simulink model "tracking_model"  (R2017a)
(part 6 of 14)

37e-11+cos(x_3).^2.*sin(x_3).^2.*7.5816135984375e-6+cos(x_4).^2.*sin(x_3).^4.*6.757062187003037e-11+cos(x_5).^2.*sin(x_3).^4.*6.757062187003037e-11+cos(x_6).^2.*sin(x_3).^4.*6.757062187003037e-11+cos(x_3).^2.*cos(x_4).^2.*sin(x_3).^2.*1.351412437400607e-10+cos(x_3).^2.*cos(x_5).^2.*sin(x_3).^2.*1.351412437400607e-10+cos(x_3).^2.*cos(x_6).^2.*sin(x_3).^2.*1.351412437400607e-10)-(x_7.*x_9.*cos(x_3).^5.*cos(x_5).*sin(x_4).^2.*sin(x_5).*sin(x_6).^2.*2.269248239967731e-24)./(cos(x_3).^4.*3.79080679921875e-6+sin(x_3).^4.*3.79080679921875e-6+cos(x_3).^4.*cos(x_4).^2.*6.757062187003037e-11+cos(x_3).^4.*cos(x_5).^2.*6.757062187003037e-11+cos(x_3).^4.*cos(x_6).^2.*6.757062187003037e-11+cos(x_3).^2.*sin(x_3).^2.*7.5816135984375e-6+cos(x_4).^2.*sin(x_3).^4.*6.757062187003037e-11+cos(x_5).^2.*sin(x_3).^4.*6.757062187003037e-11+cos(x_6).^2.*sin(x_3).^4.*6.757062187003037e-11+cos(x_3).^2.*cos(x_4).^2.*sin(x_3).^2.*1.351412437400607e-10+cos(x_3).^2.*cos(x_5).^2.*sin(x_3).^2.*1.351412437400607e-10+cos(x_3).^2.*cos(x_6).^2.*sin(x_3).^2.*1.351412437400607e-10)-(x_8.*x_9.*cos(x_3).*cos(x_5).*sin(x_3).^4.*sin(x_5).^3.*sin(x_6).^2.*1.310151082203454e-24)./(cos(x_3).^4.*3.79080679921875e-6+sin(x_3).^4.*3.79080679921875e-6+cos(x_3).^4.*cos(x_4).^2.*6.757062187003037e-11+cos(x_3).^4.*cos(x_5).^2.*6.757062187003037e-11+cos(x_3).^4.*cos(x_6).^2.*6.757062187003037e-11+cos(x_3).^2.*sin(x_3).^2.*7.5816135984375e-6+cos(x_4).^2.*sin(x_3).^4.*6.757062187003037e-11+cos(x_5).^2.*sin(x_3).^4.*6.757062187003037e-11+cos(x_6).^2.*sin(x_3).^4.*6.757062187003037e-11+cos(x_3).^2.*cos(x_4).^2.*sin(x_3).^2.*1.351412437400607e-10+cos(x_3).^2.*cos(x_5).^2.*sin(x_3).^2.*1.351412437400607e-10+cos(x_3).^2.*cos(x_6).^2.*sin(x_3).^2.*1.351412437400607e-10)-(x_8.*x_9.*cos(x_3).*cos(x_6).*sin(x_3).^4.*sin(x_4).^2.*sin(x_6).^3.*1.310151082203454e-24)./(cos(x_3).^4.*3.79080679921875e-6+sin(x_3).^4.*3.79080679921875e-6+cos(x_3).^4.*cos(x_4).^2.*6.757062187003037e-11+cos(x_3).^4.*cos(x_5).^2.*6.757062187003037e-11+cos(x_3).^4.*cos(x_6).^2.*6.757062187003037e-11+cos(x_3).^2.*sin(x_3).^2.*7.5816135984375e-6+cos(x_4).^2.*sin(x_3).^4.*6.757062187003037e-11+cos(x_5).^2.*sin(x_3).^4.*6.757062187003037e-11+cos(x_6).^2.*sin(x_3).^4.*6.757062187003037e-11+cos(x_3).^2.*cos(x_4).^2.*sin(x_3).^2.*1.351412437400607e-10+cos(x_3).^2.*cos(x_5).^2.*sin(x_3).^2.*1.351412437400607e-10+cos(x_3).^2.*cos(x_6).^2.*sin(x_3).^2.*1.351412437400607e-10)-(x_8.*x_9.*cos(x_3).^2.*cos(x_5).*sin(x_3).^3.*sin(x_5).*sin(x_6).^4.*2.269248239967731e-24)./(cos(x_3).^4.*3.79080679921875e-6+sin(x_3).^4.*3.79080679921875e-6+cos(x_3).^4.*cos(x_4).^2.*6.757062187003037e-11+cos(x_3).^4.*cos(x_5).^2.*6.757062187003037e-11+cos(x_3).^4.*cos(x_6).^2.*6.757062187003037e-11+cos(x_3).^2.*sin(x_3).^2.*7.5816135984375e-6+cos(x_4).^2.*sin(x_3).^4.*6.757062187003037e-11+cos(x_5).^2.*sin(x_3).^4.*6.757062187003037e-11+cos(x_6).^2.*sin(x_3).^4.*6.757062187003037e-11+cos(x_3).^2.*cos(x_4).^2.*sin(x_3).^2.*1.351412437400607e-10+cos(x_3).^2.*cos(x_5).^2.*sin(x_3).^2.*1.351412437400607e-10+cos(x_3).^2.*cos(x_6).^2.*sin(x_3).^2.*1.351412437400607e-10)+(x_8.*x_9.*cos(x_3).^2.*cos(x_6).*sin(x_3).^3.*sin(x_4).^4.*sin(x_6).*2.269248239967731e-24)./(cos(x_3).^4.*3.79080679921875e-6+sin(x_3).^4.*3.79080679921875e-6+cos(x_3).^4.*cos(x_4).^2.*6.757062187003037e-11+cos(x_3).^4.*cos(x_5).^2.*6.757062187003037e-11+cos(x_3).^4.*cos(x_6).^2.*6.757062187003037e-11+cos(x_3).^2.*sin(x_3).^2.*7.5816135984375e-6+cos(x_4).^2.*sin(x_3).^4.*6.757062187003037e-11+cos(x_5).^2.*sin(x_3).^4.*6.757062187003037e-11+cos(x_6).^2.*sin(x_3).^4.*6.757062187003037e-11+cos(x_3).^2.*cos(x_4).^2.*sin(x_3).^2.*1.351412437400607e-10+cos(x_3).^2.*cos(x_5).^2.*sin(x_3).^2.*1.351412437400607e-10+cos(x_3).^2.*cos(x_6).^2.*sin(x_3).^2.*1.351412437400607e-10)-(x_8.*x_9.*cos(x_3).^3.*cos(x_5).*sin(x_3).^2.*sin(x_5).*sin(x_6).^4.*1.310151082203454e-24)./(cos(x_3).^4.*3.79080679921875e-6+sin(x_3).^4.*3.79080679921875e-6+cos(x_3).^4.*cos(x_4).^2.*6.757062187003037e-11+cos(x_3).^4.*cos(x_5).^2.*6.757062187003037e-11+cos(x_3).^4.*cos(x_6).^2.*6.757062187003037e-11+cos(x_3).^2.*sin(x_3).^2.*7.5816135984375e-6+cos(x_4).^2.*sin(x_3).^4.*6.757062187003037e-11+cos(x_5).^2.*sin(x_3).^4.*6.757062187003037e-11+cos(x_6).^2.*sin(x_3).^4.*6.757062187003037e-11+cos(x_3).^2.*cos(x_4).^2.*sin(x_3).^2.*1.351412437400607e-10+cos(x_3).^2.*cos(x_5).^2.*sin(x_3).^2.*1.351412437400607e-10+cos(x_3).^2.*cos(x_6).^2.*sin(x_3).^2.*1.351412437400607e-10)-(x_8.*x_9.*cos(x_3).^3.*cos(x_6).*sin(x_3).^2.*sin(x_4).^4.*sin(x_6).*1.310151082203454e-24)./(cos(x_3).^4.*3.79080679921875e-6+sin(x_3).^4.*3.79080679921875e-6+cos(x_3).^4.*cos(x_4).^2.*6.757062187003037e-11+cos(x_3).^4.*cos(x_5).^2.*6.757062187003037e-11+cos(x_3).^4.*cos(x_6).^2.*6.757062187003037e-11+cos(x_3).^2.*sin(x_3).^2.*7.5816135984375e-6+cos(x_4).^2.*sin(x_3).^4.*6.757062187003037e-11+cos(x_5).^2.*sin(x_3).^4.*6.757062187003037e-11+cos(x_6).^2.*sin(x_3).^4.*6.757062187003037e-11+cos(x_3).^2.*cos(x_4).^2.*sin(x_3).^2.*1.351412437400607e-10+cos(x_3).^2.*cos(x_5).^2.*sin(x_3).^2.*1.351412437400607e-10+cos(x_3).^2.*cos(x_6).^2.*sin(x_3).^2.*1.351412437400607e-10)-(x_8.*x_9.*cos(x_3).^4.*cos(x_5).*sin(x_3).*sin(x_5).^3.*sin(x_6).^2.*2.269248239967731e-24)./(cos(x_3).^4.*3.79080679921875e-6+sin(x_3).^4.*3.79080679921875e-6+cos(x_3).^4.*cos(x_4).^2.*6.757062187003037e-11+cos(x_3).^4.*cos(x_5).^2.*6.757062187003037e-11+cos(x_3).^4.*cos(x_6).^2.*6.757062187003037e-11+cos(x_3).^2.*sin(x_3).^2.*7.5816135984375e-6+cos(x_4).^2.*sin(x_3).^4.*6.757062187003037e-11+cos(x_5).^2.*sin(x_3).^4.*6.757062187003037e-11+cos(x_6).^2.*sin(x_3).^4.*6.757062187003037e-11+cos(x_3).^2.*cos(x_4).^2.*sin(x_3).^2.*1.351412437400607e-10+cos(x_3).^2.*cos(x_5).^2.*sin(x_3).^2.*1.351412437400607e-10+cos(x_3).^2.*cos(x_6).^2.*sin(x_3).^2.*1.351412437400607e-10)+(x_8.*x_9.*cos(x_3).^4.*cos(x_6).*sin(x_3).*sin(x_4).^2.*sin(x_6).^3.*2.269248239967731e-24)./(cos(x_3).^4.*3.79080679921875e-6+sin(x_3).^4.*3.79080679921875e-6+cos(x_3).^4.*cos(x_4).^2.*6.757062187003037e-11+cos(x_3).^4.*cos(x_5).^2.*6.757062187003037e-11+cos(x_3).^4.*cos(x_6).^2.*6.757062187003037e-11+cos(x_3).^2.*sin(x_3).^2.*7.5816135984375e-6+cos(x_4).^2.*sin(x_3).^4.*6.757062187003037e-11+cos(x_5).^2.*sin(x_3).^4.*6.757062187003037e-11+cos(x_6).^2.*sin(x_3).^4.*6.757062187003037e-11+cos(x_3).^2.*cos(x_4).^2.*sin(x_3).^2.*1.351412437400607e-10+cos(x_3).^2.*cos(x_5).^2.*sin(x_3).^2.*1.351412437400607e-10+cos(x_3).^2.*cos(x_6).^2.*sin(x_3).^2.*1.351412437400607e-10)+(x_8.*x_9.*cos(x_3).^5.*cos(x_4).*sin(x_4).*sin(x_5).^2.*sin(x_6).^2.*2.620302164406908e-24)./(cos(x_3).^4.*3.79080679921875e-6+sin(x_3).^4.*3.79080679921875e-6+cos(x_3).^4.*cos(x_4).^2.*6.757062187003037e-11+cos(x_3).^4.*cos(x_5).^2.*6.757062187003037e-11+cos(x_3).^4.*cos(x_6).^2.*6.757062187003037e-11+cos(x_3).^2.*sin(x_3).^2.*7.5816135984375e-6+cos(x_4).^2.*sin(x_3).^4.*6.757062187003037e-11+cos(x_5).^2.*sin(x_3).^4.*6.757062187003037e-11+cos(x_6).^2.*sin(x_3).^4.*6.757062187003037e-11+cos(x_3).^2.*cos(x_4).^2.*sin(x_3).^2.*1.351412437400607e-10+cos(x_3).^2.*cos(x_5).^2.*sin(x_3).^2.*1.351412437400607e-10+cos(x_3).^2.*cos(x_6).^2.*sin(x_3).^2.*1.351412437400607e-10)+(x_7.*x_9.*cos(x_3).^5.*cos(x_6).*sin(x_4).^2.*sin(x_5).^2.*sin(x_6).*2.269248239967731e-24)./(cos(x_3).^4.*3.79080679921875e-6+sin(x_3).^4.*3.79080679921875e-6+cos(x_3).^4.*cos(x_4).^2.*6.757062187003037e-11+cos(x_3).^4.*cos(x_5).^2.*6.757062187003037e-11+cos(x_3).^4.*cos(x_6).^2.*6.757062187003037e-11+cos(x_3).^2.*sin(x_3).^2.*7.5816135984375e-6+cos(x_4).^2.*sin(x_3).^4.*6.757062187003037e-11+cos(x_5).^2.*sin(x_3).^4.*6.757062187003037e-11+cos(x_6).^2.*sin(x_3).^4.*6.757062187003037e-11+cos(x_3).^2.*cos(x_4).^2.*sin(x_3).^2.*1.351412437400607e-10+cos(x_3).^2.*cos(x_5).^2.*sin(x_3).^2.*1.351412437400607e-10+cos(x_3).^2.*cos(x_6).^2.*sin(x_3).^2.*1.351412437400607e-10)-(x_8.*x_9.*cos(x_3).*cos(x_6).*sin(x_3).^4.*sin(x_5).^2.*sin(x_6).^3.*1.310151082203454e-24)./(cos(x_3).^4.*3.79080679921875e-6+sin(x_3).^4.*3.79080679921875e-6+cos(x_3).^4.*cos(x_4).^2.*6.757062187003037e-11+cos(x_3).^4.*cos(x_5).^2.*6.757062187003037e-11+cos(x_3).^4.*cos(x_6).^2.*6.757062187003037e-11+cos(x_3).^2.*sin(x_3).^2.*7.5816135984375e-6+cos(x_4).^2.*sin(x_3).^4.*6.757062187003037e-11+cos(x_5).^2.*sin(x_3).^4.*6.757062187003037e-11+cos(x_6).^2.*sin(x_3).^4.*6.757062187003037e-11+cos(x_3).^2.*cos(x_4).^2.*sin(x_3).^2.*1.351412437400607e-10+cos(x_3).^2.*cos(x_5).^2.*sin(x_3).^2.*1.351412437400607e-10+cos(x_3).^2.*cos(x_6).^2.*sin(x_3).^2.*1.351412437400607e-10)+(x_8.*x_9.*cos(x_3).^2.*cos(x_6).*sin(x_3).^3.*sin(x_5).^4.*sin(x_6).*2.269248239967731e-24)./(cos(x_3).^4.*3.79080679921875e-6+sin(x_3).^4.*3.79080679921875e-6+cos(x_3).^4.*cos(x_4).^2.*6.757062187003037e-11+cos(x_3).^4.*cos(x_5).^2.*6.757062187003037e-11+cos(x_3).^4.*cos(x_6).^2.*6.757062187003037e-11+cos(x_3).^2.*sin(x_3).^2.*7.5816135984375e-6+cos(x_4).^2.*sin(x_3).^4.*6.757062187003037e-11+cos(x_5).^2.*sin(x_3).^4.*6.757062187003037e-11+cos(x_6).^2.*sin(x_3).^4.*6.757062187003037e-11+cos(x_3).^2.*cos(x_4).^2.*sin(x_3).^2.*1.351412437400607e-10+cos(x_3).^2.*cos(x_5).^2.*sin(x_3).^2.*1.351412437400607e-10+cos(x_3).^2.*cos(x_6).^2.*sin(x_3).^2.*1.351412437400607e-10)-(x_8.*x_9.*cos(x_3).^3.*cos(x_6).*sin(x_3).^2.*sin(x_5).^4.*sin(x_6).*1.310151082203454e-24)./(cos(x_3).^4.*3.79080679921875e-6+sin(x_3).^4.*3.79080679921875e-6+cos(x_3).^4.*cos(x_4).^2.*6.757062187003037e-11+cos(x_3).^4.*cos(x_5).^2.*6.757062187003037e-11+cos(x_3).^4.*cos(x_6).^2.*6.757062187003037e-11+cos(x_3).^2.*sin(x_3).^2.*7.5816135984375e-6+cos(x_4).^2.*sin(x_3).^4.*6.757062187003037e-11+cos(x_5).^2.*sin(x_3).^4.*6.757062187003037e-11+cos(x_6).^2.*sin(x_3).^4.*6.757062187003037e-11+cos(x_3).^2.*cos(x_4).^2.*sin(x_3).^2.*1.351412437400607e-10+cos(x_3).^2.*cos(x_5).^2.*sin(x_3).^2.*1.351412437400607e-10+cos(x_3).^2.*cos(x_6).^2.*sin(x_3).^2.*1.351412437400607e-10)+(x_8.*x_9.*cos(x_3).^4.*cos(x_6).*sin(x_3).*sin(x_5).^2.*sin(x_6).^3.*2.269248239967731e-24)./(cos(x_3).^4.*3.79080679921875e-6+sin(x_3).^4.*3.79080679921875e-6+cos(x_3).^4.*cos(x_4).^2.*6.757062187003037e-11+cos(x_3).^4.*cos(x_5).^2.*6.757062187003037e-11+cos(x_3).^4.*cos(x_6).^2.*6.757062187003037e-11+cos(x_3).^2.*sin(x_3).^2.*7.5816135984375e-6+cos(x_4).^2.*sin(x_3).^4.*6.757062187003037e-11+cos(x_5).^2.*sin(x_3).^4.*6.757062187003037e-11+cos(x_6).^2.*sin(x_3).^4.*6.757062187003037e-11+cos(x_3).^2.*cos(x_4).^2.*sin(x_3).^2.*1.351412437400607e-10+cos(x_3).^2.*cos(x_5).^2.*sin(x_3).^2.*1.351412437400607e-10+cos(x_3).^2.*cos(x_6).^2.*sin(x_3).^2.*1.351412437400607e-10)-(x_8.*x_9.*cos(x_3).^5.*cos(x_5).*sin(x_4).^2.*sin(x_5).*sin(x_6).^2.*1.310151082203454e-24)./(cos(x_3).^4.*3.79080679921875e-6+sin(x_3).^4.*3.79080679921875e-6+cos(x_3).^4.*cos(x_4).^2.*6.757062187003037e-11+cos(x_3).^4.*cos(x_5).^2.*6.757062187003037e-11+cos(x_3).^4.*cos(x_6).^2.*6.757062187003037e-11+cos(x_3).^2.*sin(x_3).^2.*7.5816135984375e-6+cos(x_4).^2.*sin(x_3).^4.*6.757062187003037e-11+cos(x_5).^2.*sin(x_3).^4.*6.757062187003037e-11+cos(x_6).^2.*sin(x_3).^4.*6.757062187003037e-11+cos(x_3).^2.*cos(x_4).^2.*sin(x_3).^2.*1.351412437400607e-10+cos(x_3).^2.*cos(x_5).^2.*sin(x_3).^2.*1.351412437400607e-10+cos(x_3).^2.*cos(x_6).^2.*sin(x_3).^2.*1.351412437400607e-10)-(x_8.*x_9.*cos(x_3).^5.*cos(x_6).*sin(x_4).^2.*sin(x_5).^2.*sin(x_6).*1.310151082203454e-24)./(cos(x_3).^4.*3.79080679921875e-6+sin(x_3).^4.*3.79080679921875e-6+cos(x_3).^4.*cos(x_4).^2.*6.757062187003037e-11+cos(x_3).^4.*cos(x_5).^2.*6.757062187003037e-11+cos(x_3).^4.*cos(x_6).^2.*6.757062187003037e-11+cos(x_3).^2.*sin(x_3).^2.*7.5816135984375e-6+cos(x_4).^2.*sin(x_3).^4.*6.757062187003037e-11+cos(x_5).^2.*sin(x_3).^4.*6.757062187003037e-11+cos(x_6).^2.*sin(x_3).^4.*6.757062187003037e-11+cos(x_3).^2.*cos(x_4).^2.*sin(x_3).^2.*1.351412437400607e-10+cos(x_3).^2.*cos(x_5).^2.*sin(x_3).^2.*1.351412437400607e-10+cos(x_3).^2.*cos(x_6).^2.*sin(x_3).^2.*1.351412437400607e-10)-(x_7.*x_9.*cos(x_3).^2.*cos(x_4).*sin(x_3).^2.*sin(x_4).*sin(x_5).^2.*4.39121857220618e-18)./(cos(x_3).^4.*1.5163227196875e-5+sin(x_3).^4.*1.5163227196875e-5+cos(x_3).^4.*cos(x_4).^2.*2.702824874801215e-10+cos(x_3).^4.*cos(x_5).^2.*2.702824874801215e-10+cos(x_3).^4.*cos(x_6).^2.*2.702824874801215e-10+cos(x_3).^2.*sin(x_3).^2.*3.032645439375e-5+cos(x_4).^2.*sin(x_3).^4.*2.702824874801215e-10+cos(x_5).^2.*sin(x_3).^4.*2.702824874801215e-10+cos(x_6).^2.*sin(x_3).^4.*2.702824874801215e-10+cos(x_3).^2.*cos(x_4).^2.*sin(x_3).^2.*5.40564974960243e-10+cos(x_3).^2.*cos(x_5).^2.*sin(x_3).^2.*5.40564974960243e-10+cos(x_3).^2.*cos(x_6).^2.*sin(x_3).^2.*5.40564974960243e-10)-(x_7.*x_9.*cos(x_3).^2.*cos(x_4).*sin(x_3).^2.*sin(x_4).*sin(x_6).^2.*4.39121857220618e-18)./(cos(x_3).^4.*1.5163227196875e-5+sin(x_3).^4.*1.5163227196875e-5+cos(x_3).^4.*cos(x_4).^2.*2.702824874801215e-10+cos(x_3).^4.*cos(x_5).^2.*2.702824874801215e-10+cos(x_3).^4.*cos(x_6).^2.*2.702824874801215e-10+cos(x_3).^2.*sin(x_3).^2.*3.032645439375e-5+cos(x_4).^2.*sin(x_3).^4.*2.702824874801215e-10+cos(x_5).^2.*sin(x_3).^4.*2.702824874801215e-10+cos(x_6).^2.*sin(x_3).^4.*2.702824874801215e-10+cos(x_3).^2.*cos(x_4).^2.*sin(x_3).^2.*5.40564974960243e-10+cos(x_3).^2.*cos(x_5).^2.*sin(x_3).^2.*5.40564974960243e-10+cos(x_3).^2.*cos(x_6).^2.*sin(x_3).^2.*5.40564974960243e-10)+(x_7.*x_9.*cos(x_3).^2.*cos(x_5).*sin(x_3).^2.*sin(x_4).^2.*sin(x_5).*5.998516123203674e-18)./(cos(x_3).^4.*1.5163227196875e-5+sin(x_3).^4.*1.5163227196875e-5+cos(x_3).^4.*cos(x_4).^2.*2.702824874801215e-10+cos(x_3).^4.*cos(x_5).^2.*2.702824874801215e-10+cos(x_3).^4.*cos(x_6).^2.*2.702824874801215e-10+cos(x_3).^2.*sin(x_3).^2.*3.032645439375e-5+cos(x_4).^2.*sin(x_3).^4.*2.702824874801215e-10+cos(x_5).^2.*sin(x_3).^4.*2.702824874801215e-10+cos(x_6).^2.*sin(x_3).^4.*2.702824874801215e-10+cos(x_3).^2.*cos(x_4).^2.*sin(x_3).^2.*5.40564974960243e-10+cos(x_3).^2.*cos(x_5).^2.*sin(x_3).^2.*5.40564974960243e-10+cos(x_3).^2.*cos(x_6).^2.*sin(x_3).^2.*5.40564974960243e-10)-(x_8.*x_9.*cos(x_3).^2.*cos(x_4).*sin(x_3).^2.*sin(x_4).*sin(x_5).^2.*4.39121857220618e-18)./(cos(x_3).^4.*1.5163227196875e-5+sin(x_3).^4.*1.5163227196875e-5+cos(x_3).^4.*cos(x_4).^2.*2.702824874801215e-10+cos(x_3).^4.*cos(x_5).^2.*2.702824874801215e-10+cos(x_3).^4.*cos(x_6).^2.*2.702824874801215e-10+cos(x_3).^2.*sin(x_3).^2.*3.032645439375e-5+cos(x_4).^2.*sin(x_3).^4.*2.702824874801215e-10+cos(x_5).^2.*sin(x_3).^4.*2.702824874801215e-10+cos(x_6).^2.*sin(x_3).^4.*2.702824874801215e-10+cos(x_3).^2.*cos(x_4).^2.*sin(x_3).^2.*5.40564974960243e-10+cos(x_3).^2.*cos(x_5).^2.*sin(x_3).^2.*5.40564974960243e-10+cos(x_3).^2.*cos(x_6).^2.*sin(x_3).^2.*5.40564974960243e-10)-(x_8.*x_9.*cos(x_3).^2.*cos(x_4).*sin(x_3).^2.*sin(x_4).*sin(x_6).^2.*4.39121857220618e-18)./(cos(x_3).^4.*1.5163227196875e-5+sin(x_3).^4.*1.5163227196875e-5+cos(x_3).^4.*cos(x_4).^2.*2.702824874801215e-10+cos(x_3).^4.*cos(x_5).^2.*2.702824874801215e-10+cos(x_3).^4.*cos(x_6).^2.*2.702824874801215e-10+cos(x_3).^2.*sin(x_3).^2.*3.032645439375e-5+cos(x_4).^2.*sin(x_3).^4.*2.702824874801215e-10+cos(x_5).^2.*sin(x_3).^4.*2.702824874801215e-10+cos(x_6).^2.*sin(x_3).^4.*2.702824874801215e-10+cos(x_3).^2.*cos(x_4).^2.*sin(x_3).^2.*5.40564974960243e-10+cos(x_3).^2.*cos(x_5).^2.*sin(x_3).^2.*5.40564974960243e-10+cos(x_3).^2.*cos(x_6).^2.*sin(x_3).^2.*5.40564974960243e-10)-(x_8.*x_9.*cos(x_3).^2.*cos(x_5).*sin(x_3).^2.*sin(x_4).^2.*sin(x_5).*1.607297550997493e-18)./(cos(x_3).^4.*1.5163227196875e-5+sin(x_3).^4.*1.5163227196875e-5+cos(x_3).^4.*cos(x_4).^2.*2.702824874801215e-10+cos(x_3).^4.*cos(x_5).^2.*2.702824874801215e-10+cos(x_3).^4.*cos(x_6).^2.*2.702824874801215e-10+cos(x_3).^2.*sin(x_3).^2.*3.032645439375e-5+cos(x_4).^2.*sin(x_3).^4.*2.702824874801215e-10+cos(x_5).^2.*sin(x_3).^4.*2.702824874801215e-10+cos(x_6).^2.*sin(x_3).^4.*2.702824874801215e-10+cos(x_3).^2.*cos(x_4).^2.*sin(x_3).^2.*5.40564974960243e-10+cos(x_3).^2.*cos(x_5).^2.*sin(x_3).^2.*5.40564974960243e-10+cos(x_3).^2.*cos(x_6).^2.*sin(x_3).^2.*5.40564974960243e-10)+(x_7.*x_9.*cos(x_3).^2.*cos(x_5).*sin(x_3).^2.*sin(x_5).*sin(x_6).^2.*5.998516123203674e-18)./(cos(x_3).^4.*1.5163227196875e-5+sin(x_3).^4.*1.5163227196875e-5+cos(x_3).^4.*cos(x_4).^2.*2.702824874801215e-10+cos(x_3).^4.*cos(x_5).^2.*2.702824874801215e-10+cos(x_3).^4.*cos(x_6).^2.*2.702824874801215e-10+cos(x_3).^2.*sin(x_3).^2.*3.032645439375e-5+cos(x_4).^2.*sin(x_3).^4.*2.702824874801215e-10+cos(x_5).^2.*sin(x_3).^4.*2.702824874801215e-10+cos(x_6).^2.*sin(x_3).^4.*2.702824874801215e-10+cos(x_3).^2.*cos(x_4).^2.*sin(x_3).^2.*5.40564974960243e-10+cos(x_3).^2.*cos(x_5).^2.*sin(x_3).^2.*5.40564974960243e-10+cos(x_3).^2.*cos(x_6).^2.*sin(x_3).^2.*5.40564974960243e-10)-(x_7.*x_9.*cos(x_3).^2.*cos(x_6).*sin(x_3).^2.*sin(x_4).^2.*sin(x_6).*1.607297550997493e-18)./(cos(x_3).^4.*1.5163227196875e-5+sin(x_3).^4.*1.5163227196875e-5+cos(x_3).^4.*cos(x_4).^2.*2.702824874801215e-10+cos(x_3).^4.*cos(x_5).^2.*2.702824874801215e-10+cos(x_3).^4.*cos(x_6).^2.*2.702824874801215e-10+cos(x_3).^2.*sin(x_3).^2.*3.032645439375e-5+cos(x_4).^2.*sin(x_3).^4.*2.702824874801215e-10+cos(x_5).^2.*sin(x_3).^4.*2.702824874801215e-10+cos(x_6).^2.*sin(x_3).^4.*2.702824874801215e-10+cos(x_3).^2.*cos(x_4).^2.*sin(x_3).^2.*5.40564974960243e-10+cos(x_3).^2.*cos(x_5).^2.*sin(x_3).^2.*5.40564974960243e-10+cos(x_3).^2.*cos(x_6).^2.*sin(x_3).^2.*5.40564974960243e-10)-(x_7.*x_9.*cos(x_3).^2.*cos(x_6).*sin(x_3).^2.*sin(x_5).^2.*sin(x_6).*1.607297550997493e-18)./(cos(x_3).^4.*1.5163227196875e-5+sin(x_3).^4.*1.5163227196875e-5+cos(x_3).^4.*cos(x_4).^2.*2.702824874801215e-10+cos(x_3).^4.*cos(x_5).^2.*2.702824874801215e-10+cos(x_3).^4.*cos(x_6).^2.*2.702824874801215e-10+cos(x_3).^2.*sin(x_3).^2.*3.032645439375e-5+cos(x_4).^2.*sin(x_3).^4.*2.702824874801215e-10+cos(x_5).^2.*sin(x_3).^4.*2.702824874801215e-10+cos(x_6).^2.*sin(x_3).^4.*2.702824874801215e-10+cos(x_3).^2.*cos(x_4).^2.*sin(x_3).^2.*5.40564974960243e-10+cos(x_3).^2.*cos(x_5).^2.*sin(x_3).^2.*5.40564974960243e-10+cos(x_3).^2.*cos(x_6).^2.*sin(x_3).^2.*5.40564974960243e-10)-(x_8.*x_9.*cos(x_3).^2.*cos(x_5).*sin(x_3).^2.*sin(x_5).*sin(x_6).^2.*1.607297550997493e-18)./(cos(x_3).^4.*1.5163227196875e-5+sin(x_3).^4.*1.5163227196875e-5+cos(x_3).^4.*cos(x_4).^2.*2.702824874801215e-10+cos(x_3).^4.*cos(x_5).^2.*2.702824874801215e-10+cos(x_3).^4.*cos(x_6).^2.*2.702824874801215e-10+cos(x_3).^2.*sin(x_3).^2.*3.032645439375e-5+cos(x_4).^2.*sin(x_3).^4.*2.702824874801215e-10+cos(x_5).^2.*sin(x_3).^4.*2.702824874801215e-10+cos(x_6).^2.*sin(x_3).^4.*2.702824874801215e-10+cos(x_3).^2.*cos(x_4).^2.*sin(x_3).^2.*5.40564974960243e-10+cos(x_3).^2.*cos(x_5).^2.*sin(x_3).^2.*5.40564974960243e-10+cos(x_3).^2.*cos(x_6).^2.*sin(x_3).^2.*5.40564974960243e-10)+(x_8.*x_9.*cos(x_3).^2.*cos(x_6).*sin(x_3).^2.*sin(x_4).^2.*sin(x_6).*5.998516123203674e-18)./(cos(x_3).^4.*1.5163227196875e-5+sin(x_3).^4.*1.5163227196875e-5+cos(x_3).^4.*cos(x_4).^2.*2.702824874801215e-10+cos(x_3).^4.*cos(x_5).^2.*2.702824874801215e-10+cos(x_3).^4.*cos(x_6).^2.*2.702824874801215e-10+cos(x_3).^2.*sin(x_3).^2.*3.032645439375e-5+cos(x_4).^2.*sin(x_3).^4.*2.702824874801215e-10+cos(x_5).^2.*sin(x_3).^4.*2.702824874801215e-10+cos(x_6).^2.*sin(x_3).^4.*2.702824874801215e-10+cos(x_3).^2.*cos(x_4).^2.*sin(x_3).^2.*5.40564974960243e-10+cos(x_3).^2.*cos(x_5).^2.*sin(x_3).^2.*5.40564974960243e-10+cos(x_3).^2.*cos(x_6).^2.*sin(x_3).^2.*5.40564974960243e-10)+(x_8.*x_9.*cos(x_3).^2.*cos(x_6).*sin(x_3).^2.*sin(x_5).^2.*sin(x_6).*5.998516123203674e-18)./(cos(x_3).^4.*1.5163227196875e-5+sin(x_3).^4.*1.5163227196875e-5+cos(x_3).^4.*cos(x_4).^2.*2.702824874801215e-10+cos(x_3).^4.*cos(x_5).^2.*2.702824874801215e-10+cos(x_3).^4.*cos(x_6).^2.*2.702824874801215e-10+cos(x_3).^2.*sin(x_3).^2.*3.032645439375e-5+cos(x_4).^2.*sin(x_3).^4.*2.702824874801215e-10+cos(x_5).^2.*sin(x_3).^4.*2.702824874801215e-10+cos(x_6).^2.*sin(x_3).^4.*2.702824874801215e-10+cos(x_3).^2.*cos(x_4).^2.*sin(x_3).^2.*5.40564974960243e-10+cos(x_3).^2.*cos(x_5).^2.*sin(x_3).^2.*5.40564974960243e-10+cos(x_3).^2.*cos(x_6).^2.*sin(x_3).^2.*5.40564974960243e-10)-(x_7.*x_9.*cos(x_4).*sin(x_3).^5.*sin(x_4).*sin(x_5).^2.*sin(x_6).^2.*2.620302164406908e-24)./(cos(x_3).^4.*3.79080679921875e-6+sin(x_3).^4.*3.79080679921875e-6+cos(x_3).^4.*cos(x_4).^2.*6.757062187003037e-11+cos(x_3).^4.*cos(x_5).^2.*6.757062187003037e-11+cos(x_3).^4.*cos(x_6).^2.*6.757062187003037e-11+cos(x_3).^2.*sin(x_3).^2.*7.5816135984375e-6+cos(x_4).^2.*sin(x_3).^4.*6.757062187003037e-11+cos(x_5).^2.*sin(x_3).^4.*6.757062187003037e-11+cos(x_6).^2.*sin(x_3).^4.*6.757062187003037e-11+cos(x_3).^2.*cos(x_4).^2.*sin(x_3).^2.*1.351412437400607e-10+cos(x_3).^2.*cos(x_5).^2.*sin(x_3).^2.*1.351412437400607e-10+cos(x_3).^2.*cos(x_6).^2.*sin(x_3).^2.*1.351412437400607e-10)+(x_7.*x_9.*cos(x_5).*sin(x_3).^5.*sin(x_4).^2.*sin(x_5).*sin(x_6).^2.*1.310151082203454e-24)./(cos(x_3).^4.*3.79080679921875e-6+sin(x_3).^4.*3.79080679921875e-6+cos(x_3).^4.*cos(x_4).^2.*6.757062187003037e-11+cos(x_3).^4.*cos(x_5).^2.*6.757062187003037e-11+cos(x_3).^4.*cos(x_6).^2.*6.757062187003037e-11+cos(x_3).^2.*sin(x_3).^2.*7.5816135984375e-6+cos(x_4).^2.*sin(x_3).^4.*6.757062187003037e-11+cos(x_5).^2.*sin(x_3).^4.*6.757062187003037e-11+cos(x_6).^2.*sin(x_3).^4.*6.757062187003037e-11+cos(x_3).^2.*cos(x_4).^2.*sin(x_3).^2.*1.351412437400607e-10+cos(x_3).^2.*cos(x_5).^2.*sin(x_3).^2.*1.351412437400607e-10+cos(x_3).^2.*cos(x_6).^2.*sin(x_3).^2.*1.351412437400607e-10)+(x_7.*x_9.*cos(x_6).*sin(x_3).^5.*sin(x_4).^2.*sin(x_5).^2.*sin(x_6).*1.310151082203454e-24)./(cos(x_3).^4.*3.79080679921875e-6+sin(x_3).^4.*3.79080679921875e-6+cos(x_3).^4.*cos(x_4).^2.*6.757062187003037e-11+cos(x_3).^4.*cos(x_5).^2.*6.757062187003037e-11+cos(x_3).^4.*cos(x_6).^2.*6.757062187003037e-11+cos(x_3).^2.*sin(x_3).^2.*7.5816135984375e-6+cos(x_4).^2.*sin(x_3).^4.*6.757062187003037e-11+cos(x_5).^2.*sin(x_3).^4.*6.757062187003037e-11+cos(x_6).^2.*sin(x_3).^4.*6.757062187003037e-11+cos(x_3).^2.*cos(x_4).^2.*sin(x_3).^2.*1.351412437400607e-10+cos(x_3).^2.*cos(x_5).^2.*sin(x_3).^2.*1.351412437400607e-10+cos(x_3).^2.*cos(x_6).^2.*sin(x_3).^2.*1.351412437400607e-10)-(x_8.*x_9.*cos(x_5).*sin(x_3).^5.*sin(x_4).^2.*sin(x_5).*sin(x_6).^2.*2.269248239967731e-24)./(cos(x_3).^4.*3.79080679921875e-6+sin(x_3).^4.*3.79080679921875e-6+cos(x_3).^4.*cos(x_4).^2.*6.757062187003037e-11+cos(x_3).^4.*cos(x_5).^2.*6.757062187003037e-11+cos(x_3).^4.*cos(x_6).^2.*6.757062187003037e-11+cos(x_3).^2.*sin(x_3).^2.*7.5816135984375e-6+cos(x_4).^2.*sin(x_3).^4.*6.757062187003037e-11+cos(x_5).^2.*sin(x_3).^4.*6.757062187003037e-11+cos(x_6).^2.*sin(x_3).^4.*6.757062187003037e-11+cos(x_3).^2.*cos(x_4).^2.*sin(x_3).^2.*1.351412437400607e-10+cos(x_3).^2.*cos(x_5).^2.*sin(x_3).^2.*1.351412437400607e-10+cos(x_3).^2.*cos(x_6).^2.*sin(x_3).^2.*1.351412437400607e-10)+(x_8.*x_9.*cos(x_6).*sin(x_3).^5.*sin(x_4).^2.*sin(x_5).^2.*sin(x_6).*2.269248239967731e-24)./(cos(x_3).^4.*3.79080679921875e-6+sin(x_3).^4.*3.79080679921875e-6+cos(x_3).^4.*cos(x_4).^2.*6.757062187003037e-11+cos(x_3).^4.*cos(x_5).^2.*6.757062187003037e-11+cos(x_3).^4.*cos(x_6).^2.*6.757062187003037e-11+cos(x_3).^2.*sin(x_3).^2.*7.5816135984375e-6+cos(x_4).^2.*sin(x_3).^4.*6.757062187003037e-11+cos(x_5).^2.*sin(x_3).^4.*6.757062187003037e-11+cos(x_6).^2.*sin(x_3).^4.*6.757062187003037e-11+cos(x_3).^2.*cos(x_4).^2.*sin(x_3).^2.*1.351412437400607e-10+cos(x_3).^2.*cos(x_5).^2.*sin(x_3).^2.*1.351412437400607e-10+cos(x_3).^2.*cos(x_6).^2.*sin(x_3).^2.*1.351412437400607e-10)-(x_7.*x_9.*cos(x_3).^2.*cos(x_4).*sin(x_3).^3.*sin(x_4).^3.*sin(x_5).^2.*5.240604328813817e-24)./(cos(x_3).^4.*3.79080679921875e-6+sin(x_3).^4.*3.79080679921875e-6+cos(x_3).^4.*cos(x_4).^2.*6.757062187003037e-11+cos(x_3).^4.*cos(x_5).^2.*6.757062187003037e-11+cos(x_3).^4.*cos(x_6).^2.*6.757062187003037e-11+cos(x_3).^2.*sin(x_3).^2.*7.5816135984375e-6+cos(x_4).^2.*sin(x_3).^4.*6.757062187003037e-11+cos(x_5).^2.*sin(x_3).^4.*6.757062187003037e-11+cos(x_6).^2.*sin(x_3).^4.*6.757062187003037e-11+cos(x_3).^2.*cos(x_4).^2.*sin(x_3).^2.*1.351412437400607e-10+cos(x_3).^2.*cos(x_5).^2.*sin(x_3).^2.*1.351412437400607e-10+cos(x_3).^2.*cos(x_6).^2.*sin(x_3).^2.*1.351412437400607e-10)-(x_7.*x_9.*cos(x_3).^2.*cos(x_4).*sin(x_3).^3.*sin(x_4).^3.*sin(x_6).^2.*5.240604328813817e-24)./(cos(x_3).^4.*3.79080679921875e-6+sin(x_3).^4.*3.79080679921875e-6+cos(x_3).^4.*cos(x_4).^2.*6.757062187003037e-11+cos(x_3).^4.*cos(x_5).^2.*6.757062187003037e-11+cos(x_3).^4.*cos(x_6).^2.*6.757062187003037e-11+cos(x_3).^2.*sin(x_3).^2.*7.5816135984375e-6+cos(x_4).^2.*sin(x_3).^4.*6.757062187003037e-11+cos(x_5).^2.*sin(x_3).^4.*6.757062187003037e-11+cos(x_6).^2.*sin(x_3).^4.*6.757062187003037e-11+cos(x_3).^2.*cos(x_4).^2.*sin(x_3).^2.*1.351412437400607e-10+cos(x_3).^2.*cos(x_5).^2.*sin(x_3).^2.*1.351412437400607e-10+cos(x_3).^2.*cos(x_6).^2.*sin(x_3).^2.*1.351412437400607e-10)+(x_7.*x_9.*cos(x_3).^2.*cos(x_5).*sin(x_3).^3.*sin(x_4).^2.*sin(x_5).^3.*2.620302164406908e-24)./(cos(x_3).^4.*3.79080679921875e-6+sin(x_3).^4.*3.79080679921875e-6+cos(x_3).^4.*cos(x_4).^2.*6.757062187003037e-11+cos(x_3).^4.*cos(x_5).^2.*6.757062187003037e-11+cos(x_3).^4.*cos(x_6).^2.*6.757062187003037e-11+cos(x_3).^2.*sin(x_3).^2.*7.5816135984375e-6+cos(x_4).^2.*sin(x_3).^4.*6.757062187003037e-11+cos(x_5).^2.*sin(x_3).^4.*6.757062187003037e-11+cos(x_6).^2.*sin(x_3).^4.*6.757062187003037e-11+cos(x_3).^2.*cos(x_4).^2.*sin(x_3).^2.*1.351412437400607e-10+cos(x_3).^2.*cos(x_5).^2.*sin(x_3).^2.*1.351412437400607e-10+cos(x_3).^2.*cos(x_6).^2.*sin(x_3).^2.*1.351412437400607e-10)-(x_7.*x_9.*cos(x_3).^3.*cos(x_5).*sin(x_3).^2.*sin(x_4).^2.*sin(x_5).^3.*4.538496479935463e-24)./(cos(x_3).^4.*3.79080679921875e-6+sin(x_3).^4.*3.79080679921875e-6+cos(x_3).^4.*cos(x_4).^2.*6.757062187003037e-11+cos(x_3).^4.*cos(x_5).^2.*6.757062187003037e-11+cos(x_3).^4.*cos(x_6).^2.*6.757062187003037e-11+cos(x_3).^2.*sin(x_3).^2.*7.5816135984375e-6+cos(x_4).^2.*sin(x_3).^4.*6.757062187003037e-11+cos(x_5).^2.*sin(x_3).^4.*6.757062187003037e-11+cos(x_6).^2.*sin(x_3).^4.*6.757062187003037e-11+cos(x_3).^2.*cos(x_4).^2.*sin(x_3).^2.*1.351412437400607e-10+cos(x_3).^2.*cos(x_5).^2.*sin(x_3).^2.*1.351412437400607e-10+cos(x_3).^2.*cos(x_6).^2.*sin(x_3).^2.*1.351412437400607e-10)+(x_8.*x_9.*cos(x_3).^3.*cos(x_4).*sin(x_3).^2.*sin(x_4).^3.*sin(x_5).^2.*5.240604328813817e-24)./(cos(x_3).^4.*3.79080679921875e-6+sin(x_3).^4.*3.79080679921875e-6+cos(x_3).^4.*cos(x_4).^2.*6.757062187003037e-11+cos(x_3).^4.*cos(x_5).^2.*6.757062187003037e-11+cos(x_3).^4.*cos(x_6).^2.*6.757062187003037e-11+cos(x_3).^2.*sin(x_3).^2.*7.5816135984375e-6+cos(x_4).^2.*sin(x_3).^4.*6.757062187003037e-11+cos(x_5).^2.*sin(x_3).^4.*6.757062187003037e-11+cos(x_6).^2.*sin(x_3).^4.*6.757062187003037e-11+cos(x_3).^2.*cos(x_4).^2.*sin(x_3).^2.*1.351412437400607e-10+cos(x_3).^2.*cos(x_5).^2.*sin(x_3).^2.*1.351412437400607e-10+cos(x_3).^2.*cos(x_6).^2.*sin(x_3).^2.*1.351412437400607e-10)-(x_8.*x_9.*cos(x_3).^2.*cos(x_5).*sin(x_3).^3.*sin(x_4).^2.*sin(x_5).^3.*4.538496479935463e-24)./(cos(x_3).^4.*3.79080679921875e-6+sin(x_3).^4.*3.79080679921875e-6+cos(x_3).^4.*cos(x_4).^2.*6.757062187003037e-11+cos(x_3).^4.*cos(x_5).^2.*6.757062187003037e-11+cos(x_3).^4.*cos(x_6).^2.*6.757062187003037e-11+cos(x_3).^2.*sin(x_3).^2.*7.5816135984375e-6+cos(x_4).^2.*sin(x_3).^4.*6.757062187003037e-11+cos(x_5).^2.*sin(x_3).^4.*6.757062187003037e-11+cos(x_6).^2.*sin(x_3).^4.*6.757062187003037e-11+cos(x_3).^2.*cos(x_4).^2.*sin(x_3).^2.*1.351412437400607e-10+cos(x_3).^2.*cos(x_5).^2.*sin(x_3).^2.*1.351412437400607e-10+cos(x_3).^2.*cos(x_6).^2.*sin(x_3).^2.*1.351412437400607e-10)+(x_8.*x_9.*cos(x_3).^3.*cos(x_4).*sin(x_3).^2.*sin(x_4).^3.*sin(x_6).^2.*5.240604328813817e-24)./(cos(x_3).^4.*3.79080679921875e-6+sin(x_3).^4.*3.79080679921875e-6+cos(x_3).^4.*cos(x_4).^2.*6.757062187003037e-11+cos(x_3).^4.*cos(x_5).^2.*6.757062187003037e-11+cos(x_3).^4.*cos(x_6).^2.*6.757062187003037e-11+cos(x_3).^2.*sin(x_3).^2.*7.5816135984375e-6+cos(x_4).^2.*sin(x_3).^4.*6.757062187003037e-11+cos(x_5).^2.*sin(x_3).^4.*6.757062187003037e-11+cos(x_6).^2.*sin(x_3).^4.*6.757062187003037e-11+cos(x_3).^2.*cos(x_4).^2.*sin(x_3).^2.*1.351412437400607e-10+cos(x_3).^2.*cos(x_5).^2.*sin(x_3).^2.*1.351412437400607e-10+cos(x_3).^2.*cos(x_6).^2.*sin(x_3).^2.*1.351412437400607e-10)-(x_8.*x_9.*cos(x_3).^3.*cos(x_5).*sin(x_3).^2.*sin(x_4).^2.*sin(x_5).^3.*2.620302164406908e-24)./(cos(x_3).^4.*3.79080679921875e-6+sin(x_3).^4.*3.79080679921875e-6+cos(x_3).^4.*cos(x_4).^2.*6.757062187003037e-11+cos(x_3).^4.*cos(x_5).^2.*6.757062187003037e-11+cos(x_3).^4.*cos(x_6).^2.*6.757062187003037e-11+cos(x_3).^2.*sin(x_3).^2.*7.5816135984375e-6+cos(x_4).^2.*sin(x_3).^4.*6.757062187003037e-11+cos(x_5).^2.*sin(x_3).^4.*6.757062187003037e-11+cos(x_6).^2.*sin(x_3).^4.*6.757062187003037e-11+cos(x_3).^2.*cos(x_4).^2.*sin(x_3).^2.*1.351412437400607e-10+cos(x_3).^2.*cos(x_5).^2.*sin(x_3).^2.*1.351412437400607e-10+cos(x_3).^2.*cos(x_6).^2.*sin(x_3).^2.*1.351412437400607e-10)+(x_7.*x_9.*cos(x_3).^2.*cos(x_5).*sin(x_3).^3.*sin(x_5).^3.*sin(x_6).^2.*2.620302164406908e-24)./(cos(x_3).^4.*3.79080679921875e-6+sin(x_3).^4.*3.79080679921875e-6+cos(x_3).^4.*cos(x_4).^2.*6.757062187003037e-11+cos(x_3).^4.*cos(x_5).^2.*6.757062187003037e-11+cos(x_3).^4.*cos(x_6).^2.*6.757062187003037e-11+cos(x_3).^2.*sin(x_3).^2.*7.5816135984375e-6+cos(x_4).^2.*sin(x_3).^4.*6.757062187003037e-11+cos(x_5).^2.*sin(x_3).^4.*6.757062187003037e-11+cos(x_6).^2.*sin(x_3).^4.*6.757062187003037e-11+cos(x_3).^2.*cos(x_4).^2.*sin(x_3).^2.*1.351412437400607e-10+cos(x_3).^2.*cos(x_5).^2.*sin(x_3).^2.*1.351412437400607e-10+cos(x_3).^2.*cos(x_6).^2.*sin(x_3).^2.*1.351412437400607e-10)+(x_7.*x_9.*cos(x_3).^2.*cos(x_6).*sin(x_3).^3.*sin(x_4).^2.*sin(x_6).^3.*2.620302164406908e-24)./(cos(x_3).^4.*3.79080679921875e-6+sin(x_3).^4.*3.79080679921875e-6+cos(x_3).^4.*cos(x_4).^2.*6.757062187003037e-11+cos(x_3).^4.*cos(x_5).^2.*6.757062187003037e-11+cos(x_3).^4.*cos(x_6).^2.*6.757062187003037e-11+cos(x_3).^2.*sin(x_3).^2.*7.5816135984375e-6+cos(x_4).^2.*sin(x_3).^4.*6.757062187003037e-11+cos(x_5).^2.*sin(x_3).^4.*6.757062187003037e-11+cos(x_6).^2.*sin(x_3).^4.*6.757062187003037e-11+cos(x_3).^2.*cos(x_4).^2.*sin(x_3).^2.*1.351412437400607e-10+cos(x_3).^2.*cos(x_5).^2.*sin(x_3).^2.*1.351412437400607e-10+cos(x_3).^2.*cos(x_6).^2.*sin(x_3).^2.*1.351412437400607e-10)-(x_7.*x_9.*cos(x_3).^3.*cos(x_5).*sin(x_3).^2.*sin(x_5).^3.*sin(x_6).^2.*4.538496479935463e-24)./(cos(x_3).^4.*3.79080679921875e-6+sin(x_3).^4.*3.79080679921875e-6+cos(x_3).^4.*cos(x_4).^2.*6.757062187003037e-11+cos(x_3).^4.*cos(x_5).^2.*6.757062187003037e-11+cos(x_3).^4.*cos(x_6).^2.*6.757062187003037e-11+cos(x_3).^2.*sin(x_3).^2.*7.5816135984375e-6+cos(x_4).^2.*sin(x_3).^4.*6.757062187003037e-11+cos(x_5).^2.*sin(x_3).^4.*6.757062187003037e-11+cos(x_6).^2.*sin(x_3).^4.*6.757062187003037e-11+cos(x_3).^2.*cos(x_4).^2.*sin(x_3).^2.*1.351412437400607e-10+cos(x_3).^2.*cos(x_5).^2.*sin(x_3).^2.*1.351412437400607e-10+cos(x_3).^2.*cos(x_6).^2.*sin(x_3).^2.*1.351412437400607e-10)+(x_7.*x_9.*cos(x_3).^3.*cos(x_6).*sin(x_3).^2.*sin(x_4).^2.*sin(x_6).^3.*4.538496479935463e-24)./(cos(x_3).^4.*3.79080679921875e-6+sin(x_3).^4.*3.79080679921875e-6+cos(x_3).^4.*cos(x_4).^2.*6.757062187003037e-11+cos(x_3).^4.*cos(x_5).^2.*6.757062187003037e-11+cos(x_3).^4.*cos(x_6).^2.*6.757062187003037e-11+cos(x_3).^2.*sin(x_3).^2.*7.5816135984375e-6+cos(x_4).^2.*sin(x_3).^4.*6.757062187003037e-11+cos(x_5).^2.*sin(x_3).^4.*6.757062187003037e-11+cos(x_6).^2.*sin(x_3).^4.*6.757062187003037e-11+cos(x_3).^2.*cos(x_4).^2.*sin(x_3).^2.*1.351412437400607e-10+cos(x_3).^2.*cos(x_5).^2.*sin(x_3).^2.*1.351412437400607e-10+cos(x_3).^2.*cos(x_6).^2.*sin(x_3).^2.*1.351412437400607e-10)+(x_7.*x_9.*cos(x_3).^2.*cos(x_6).*sin(x_3).^3.*sin(x_5).^2.*sin(x_6).^3.*2.620302164406908e-24)./(cos(x_3).^4.*3.79080679921875e-6+sin(x_3).^4.*3.79080679921875e-6+cos(x_3).^4.*cos(x_4).^2.*6.757062187003037e-11+cos(x_3).^4.*cos(x_5).^2.*6.757062187003037e-11+cos(x_3).^4.*cos(x_6).^2.*6.757062187003037e-11+cos(x_3).^2.*sin(x_3).^2.*7.5816135984375e-6+cos(x_4).^2.*sin(x_3).^4.*6.757062187003037e-11+cos(x_5).^2.*sin(x_3).^4.*6.757062187003037e-11+cos(x_6).^2.*sin(x_3).^4.*6.757062187003037e-11+cos(x_3).^2.*cos(x_4).^2.*sin(x_3).^2.*1.351412437400607e-10+cos(x_3).^2.*cos(x_5).^2.*sin(x_3).^2.*1.351412437400607e-10+cos(x_3).^2.*cos(x_6).^2.*sin(x_3).^2.*1.351412437400607e-10)+(x_7.*x_9.*cos(x_3).^3.*cos(x_6).*sin(x_3).^2.*sin(x_5).^2.*sin(x_6).^3.*4.538496479935463e-24)./(cos(x_3).^4.*3.79080679921875e-6+sin(x_3).^4.*3.79080679921875e-6+cos(x_3).^4.*cos(x_4).^2.*6.757062187003037e-11+cos(x_3).^4.*cos(x_5).^2.*6.757062187003037e-11+cos(x_3).^4.*cos(x_6).^2.*6.757062187003037e-11+cos(x_3).^2.*sin(x_3).^2.*7.5816135984375e-6+cos(x_4).^2.*sin(x_3).^4.*6.757062187003037e-11+cos(x_5).^2.*sin(x_3).^4.*6.757062187003037e-11+cos(x_6).^2.*sin(x_3).^4.*6.757062187003037e-11+cos(x_3).^2.*cos(x_4).^2.*sin(x_3).^2.*1.351412437400607e-10+cos(x_3).^2.*cos(x_5).^2.*sin(x_3).^2.*1.351412437400607e-10+cos(x_3).^2.*cos(x_6).^2.*sin(x_3).^2.*1.351412437400607e-10)-(x_8.*x_9.*cos(x_3).^2.*cos(x_5).*sin(x_3).^3.*sin(x_5).^3.*sin(x_6).^2.*4.538496479935463e-24)./(cos(x_3).^4.*3.79080679921875e-6+sin(x_3).^4.*3.79080679921875e-6+cos(x_3).^4.*cos(x_4).^2.*6.757062187003037e-11+cos(x_3).^4.*cos(x_5).^2.*6.757062187003037e-11+cos(x_3).^4.*cos(x_6).^2.*6.757062187003037e-11+cos(x_3).^2.*sin(x_3).^2.*7.5816135984375e-6+cos(x_4).^2.*sin(x_3).^4.*6.757062187003037e-11+cos(x_5).^2.*sin(x_3).^4.*6.757062187003037e-11+cos(x_6).^2.*sin(x_3).^4.*6.757062187003037e-11+cos(x_3).^2.*cos(x_4).^2.*sin(x_3).^2.*1.351412437400607e-10+cos(x_3).^2.*cos(x_5).^2.*sin(x_3).^2.*1.351412437400607e-10+cos(x_3).^2.*cos(x_6).^2.*sin(x_3).^2.*1.351412437400607e-10)+(x_8.*x_9.*cos(x_3).^2.*cos(x_6).*sin(x_3).^3.*sin(x_4).^2.*sin(x_6).^3.*4.538496479935463e-24)./(cos(x_3).^4.*3.79080679921875e-6+sin(x_3).^4.*3.79080679921875e-6+cos(x_3).^4.*cos(x_4).^2.*6.757062187003037e-11+cos(x_3).^4.*cos(x_5).^2.*6.757062187003037e-11+cos(x_3).^4.*cos(x_6).^2.*6.757062187003037e-11+cos(x_3).^2.*sin(x_3).^2.*7.5816135984375e-6+cos(x_4).^2.*sin(x_3).^4.*6.757062187003037e-11+cos(x_5).^2.*sin(x_3).^4.*6.757062187003037e-11+cos(x_6).^2.*sin(x_3).^4.*6.757062187003037e-11+cos(x_3).^2.*cos(x_4).^2.*sin(x_3).^2.*1.351412437400607e-10+cos(x_3).^2.*cos(x_5).^2.*sin(x_3).^2.*1.351412437400607e-10+cos(x_3).^2.*cos(x_6).^2.*sin(x_3).^2.*1.351412437400607e-10)-(x_8.*x_9.*cos(x_3).^3.*cos(x_5).*sin(x_3).^2.*sin(x_5).^3.*sin(x_6).^2.*2.620302164406908e-24)./(cos(x_3).^4.*3.79080679921875e-6+sin(x_3).^4.*3.79080679921875e-6+cos(x_3).^4.*cos(x_4).^2.*6.757062187003037e-11+cos(x_3).^4.*cos(x_5).^2.*6.757062187003037e-11+cos(x_3).^4.*cos(x_6).^2.*6.757062187003037e-11+cos(x_3).^2.*sin(x_3).^2.*7.5816135984375e-6+cos(x_4).^2.*sin(x_3).^4.*6.757062187003037e-11+cos(x_5).^2.*sin(x_3).^4.*6.757062187003037e-11+cos(x_6).^2.*sin(x_3).^4.*6.757062187003037e-11+cos(x_3).^2.*cos(x_4).^2.*sin(x_3).^2.*1.351412437400607e-10+cos(x_3).^2.*cos(x_5).^2.*sin(x_3).^2.*1.351412437400607e-10+cos(x_3).^2.*cos(x_6).^2.*sin(x_3).^2.*1.351412437400607e-10)-(x_8.*x_9.*cos(x_3).^3.*cos(x_6).*sin(x_3).^2.*sin(x_4).^2.*sin(x_6).^3.*2.620302164406908e-24)./(cos(x_3).^4.*3.79080679921875e-6+sin(x_3).^4.*3.79080679921875e-6+cos(x_3).^4.*cos(x_4).^2.*6.757062187003037e-11+cos(x_3).^4.*cos(x_5).^2.*6.757062187003037e-11+cos(x_3).^4.*cos(x_6).^2.*6.757062187003037e-11+cos(x_3).^2.*sin(x_3).^2.*7.5816135984375e-6+cos(x_4).^2.*sin(x_3).^4.*6.757062187003037e-11+cos(x_5).^2.*sin(x_3).^4.*6.757062187003037e-11+cos(x_6).^2.*sin(x_3).^4.*6.757062187003037e-11+cos(x_3).^2.*cos(x_4).^2.*sin(x_3).^2.*1.351412437400607e-10+cos(x_3).^2.*cos(x_5).^2.*sin(x_3).^2.*1.351412437400607e-10+cos(x_3).^2.*cos(x_6).^2.*sin(x_3).^2.*1.351412437400607e-10)+(x_8.*x_9.*cos(x_3).^2.*cos(x_6).*sin(x_3).^3.*sin(x_5).^2.*sin(x_6).^3.*4.538496479935463e-24)./(cos(x_3).^4.*3.79080679921875e-6+sin(x_3).^4.*3.79080679921875e-6+cos(x_3).^4.*cos(x_4).^2.*6.757062187003037e-11+cos(x_3).^4.*cos(x_5).^2.*6.757062187003037e-11+cos(x_3).^4.*cos(x_6).^2.*6.757062187003037e-11+cos(x_3).^2.*sin(x_3).^2.*7.5816135984375e-6+cos(x_4).^2.*sin(x_3).^4.*6.757062187003037e-11+cos(x_5).^2.*sin(x_3).^4.*6.757062187003037e-11+cos(x_6).^2.*sin(x_3).^4.*6.757062187003037e-11+cos(x_3).^2.*cos(x_4).^2.*sin(x_3).^2.*1.351412437400607e-10+cos(x_3).^2.*cos(x_5).^2.*sin(x_3).^2.*1.351412437400607e-10+cos(x_3).^2.*cos(x_6).^2.*sin(x_3).^2.*1.351412437400607e-10)-(x_8.*x_9.*cos(x_3).^3.*cos(x_6).*sin(x_3).^2.*sin(x_5).^2.*sin(x_6).^3.*2.620302164406908e-24)./(cos(x_3).^4.*3.79080679921875e-6+sin(x_3).^4.*3.79080679921875e-6+cos(x_3).^4.*cos(x_4).^2.*6.757062187003037e-11+cos(x_3).^4.*cos(x_5).^2.*6.757062187003037e-11+cos(x_3).^4.*cos(x_6).^2.*6.757062187003037e-11+cos(x_3).^2.*sin(x_3).^2.*7.5816135984375e-6+cos(x_4).^2.*sin(x_3).^4.*6.757062187003037e-11+cos(x_5).^2.*sin(x_3).^4.*6.757062187003037e-11+cos(x_6).^2.*sin(x_3).^4.*6.757062187003037e-11+cos(x_3).^2.*cos(x_4).^2.*sin(x_3).^2.*1.351412437400607e-10+cos(x_3).^2.*cos(x_5).^2.*sin(x_3).^2.*1.351412437400607e-10+cos(x_3).^2.*cos(x_6).^2.*sin(x_3).^2.*1.351412437400607e-10)-(x_7.*x_9.*cos(x_3).^4.*cos(x_4).*sin(x_3).*sin(x_4).*sin(x_5).^2.*sin(x_6).^2.*2.620302164406908e-24)./(cos(x_3).^4.*3.79080679921875e-6+sin(x_3).^4.*3.79080679921875e-6+cos(x_3).^4.*cos(x_4).^2.*6.757062187003037e-11+cos(x_3).^4.*cos(x_5).^2.*6.757062187003037e-11+cos(x_3).^4.*cos(x_6).^2.*6.757062187003037e-11+cos(x_3).^2.*sin(x_3).^2.*7.5816135984375e-6+cos(x_4).^2.*sin(x_3).^4.*6.757062187003037e-11+cos(x_5).^2.*sin(x_3).^4.*6.757062187003037e-11+cos(x_6).^2.*sin(x_3).^4.*6.757062187003037e-11+cos(x_3).^2.*cos(x_4).^2.*sin(x_3).^2.*1.351412437400607e-10+cos(x_3).^2.*cos(x_5).^2.*sin(x_3).^2.*1.351412437400607e-10+cos(x_3).^2.*cos(x_6).^2.*sin(x_3).^2.*1.351412437400607e-10)-(x_7.*x_9.*cos(x_3).*cos(x_5).*sin(x_3).^4.*sin(x_4).^2.*sin(x_5).*sin(x_6).^2.*2.269248239967731e-24)./(cos(x_3).^4.*3.79080679921875e-6+sin(x_3).^4.*3.79080679921875e-6+cos(x_3).^4.*cos(x_4).^2.*6.757062187003037e-11+cos(x_3).^4.*cos(x_5).^2.*6.757062187003037e-11+cos(x_3).^4.*cos(x_6).^2.*6.757062187003037e-11+cos(x_3).^2.*sin(x_3).^2.*7.5816135984375e-6+cos(x_4).^2.*sin(x_3).^4.*6.757062187003037e-11+cos(x_5).^2.*sin(x_3).^4.*6.757062187003037e-11+cos(x_6).^2.*sin(x_3).^4.*6.757062187003037e-11+cos(x_3).^2.*cos(x_4).^2.*sin(x_3).^2.*1.351412437400607e-10+cos(x_3).^2.*cos(x_5).^2.*sin(x_3).^2.*1.351412437400607e-10+cos(x_3).^2.*cos(x_6).^2.*sin(x_3).^2.*1.351412437400607e-10)+(x_7.*x_9.*cos(x_3).^4.*cos(x_5).*sin(x_3).*sin(x_4).^2.*sin(x_5).*sin(x_6).^2.*1.310151082203454e-24)./(cos(x_3).^4.*3.79080679921875e-6+sin(x_3).^4.*3.79080679921875e-6+cos(x_3).^4.*cos(x_4).^2.*6.757062187003037e-11+cos(x_3).^4.*cos(x_5).^2.*6.757062187003037e-11+cos(x_3).^4.*cos(x_6).^2.*6.757062187003037e-11+cos(x_3).^2.*sin(x_3).^2.*7.5816135984375e-6+cos(x_4).^2.*sin(x_3).^4.*6.757062187003037e-11+cos(x_5).^2.*sin(x_3).^4.*6.757062187003037e-11+cos(x_6).^2.*sin(x_3).^4.*6.757062187003037e-11+cos(x_3).^2.*cos(x_4).^2.*sin(x_3).^2.*1.351412437400607e-10+cos(x_3).^2.*cos(x_5).^2.*sin(x_3).^2.*1.351412437400607e-10+cos(x_3).^2.*cos(x_6).^2.*sin(x_3).^2.*1.351412437400607e-10)+(x_8.*x_9.*cos(x_3).*cos(x_4).*sin(x_3).^4.*sin(x_4).*sin(x_5).^2.*sin(x_6).^2.*2.620302164406908e-24)./(cos(x_3).^4.*3.79080679921875e-6+sin(x_3).^4.*3.79080679921875e-6+cos(x_3).^4.*cos(x_4).^2.*6.757062187003037e-11+cos(x_3).^4.*cos(x_5).^2.*6.757062187003037e-11+cos(x_3).^4.*cos(x_6).^2.*6.757062187003037e-11+cos(x_3).^2.*sin(x_3).^2.*7.5816135984375e-6+cos(x_4).^2.*sin(x_3).^4.*6.757062187003037e-11+cos(x_5).^2.*sin(x_3).^4.*6.757062187003037e-11+cos(x_6).^2.*sin(x_3).^4.*6.757062187003037e-11+cos(x_3).^2.*cos(x_4).^2.*sin(x_3).^2.*1.351412437400607e-10+cos(x_3).^2.*cos(x_5).^2.*sin(x_3).^2.*1.351412437400607e-10+cos(x_3).^2.*cos(x_6).^2.*sin(x_3).^2.*1.351412437400607e-10)+(x_7.*x_9.*cos(x_3).*cos(x_6).*sin(x_3).^4.*sin(x_4).^2.*sin(x_5).^2.*sin(x_6).*2.269248239967731e-24)./(cos(x_3).^4.*3.79080679921875e-6+sin(x_3).^4.*3.79080679921875e-6+cos(x_3).^4.*cos(x_4).^2.*6.757062187003037e-11+cos(x_3).^4.*cos(x_5).^2.*6.757062187003037e-11+cos(x_3).^4.*cos(x_6).^2.*6.757062187003037e-11+cos(x_3).^2.*sin(x_3).^2.*7.5816135984375e-6+cos(x_4).^2.*sin(x_3).^4.*6.757062187003037e-11+cos(x_5).^2.*sin(x_3).^4.*6.757062187003037e-11+cos(x_6).^2.*sin(x_3).^4.*6.757062187003037e-11+cos(x_3).^2.*cos(x_4).^2.*sin(x_3).^2.*1.351412437400607e-10+cos(x_3).^2.*cos(x_5).^2.*sin(x_3).^2.*1.351412437400607e-10+cos(x_3).^2.*cos(x_6).^2.*sin(x_3).^2.*1.351412437400607e-10)+(x_7.*x_9.*cos(x_3).^4.*cos(x_6).*sin(x_3).*sin(x_4).^2.*sin(x_5).^2.*sin(x_6).*1.310151082203454e-24)./(cos(x_3).^4.*3.79080679921875e-6+sin(x_3).^4.*3.79080679921875e-6+cos(x_3).^4.*cos(x_4).^2.*6.757062187003037e-11+cos(x_3).^4.*cos(x_5).^2.*6.757062187003037e-11+cos(x_3).^4.*cos(x_6).^2.*6.757062187003037e-11+cos(x_3).^2.*sin(x_3).^2.*7.5816135984375e-6+cos(x_4).^2.*sin(x_3).^4.*6.757062187003037e-11+cos(x_5).^2.*sin(x_3).^4.*6.757062187003037e-11+cos(x_6).^2.*sin(x_3).^4.*6.757062187003037e-11+cos(x_3).^2.*cos(x_4).^2.*sin(x_3).^2.*1.351412437400607e-10+cos(x_3).^2.*cos(x_5).^2.*sin(x_3).^2.*1.351412437400607e-10+cos(x_3).^2.*cos(x_6).^2.*sin(x_3).^2.*1.351412437400607e-10)-(x_8.*x_9.*cos(x_3).*cos(x_5).*sin(x_3).^4.*sin(x_4).^2.*sin(x_5).*sin(x_6).^2.*1.310151082203454e-24)./(cos(x_3).^4.*3.79080679921875e-6+sin(x_3).^4.*3.79080679921875e-6+cos(x_3).^4.*cos(x_4).^2.*6.757062187003037e-11+cos(x_3).^4.*cos(x_5).^2.*6.757062187003037e-11+cos(x_3).^4.*cos(x_6).^2.*6.757062187003037e-11+cos(x_3).^2.*sin(x_3).^2.*7.5816135984375e-6+cos(x_4).^2.*sin(x_3).^4.*6.757062187003037e-11+cos(x_5).^2.*sin(x_3).^4.*6.757062187003037e-11+cos(x_6).^2.*sin(x_3).^4.*6.757062187003037e-11+cos(x_3).^2.*cos(x_4).^2.*sin(x_3).^2.*1.351412437400607e-10+cos(x_3).^2.*cos(x_5).^2.*sin(x_3).^2.*1.351412437400607e-10+cos(x_3).^2.*cos(x_6).^2.*sin(x_3).^2.*1.351412437400607e-10)-(x_8.*x_9.*cos(x_3).^4.*cos(x_5).*sin(x_3).*sin(x_4).^2.*sin(x_5).*sin(x_6).^2.*2.269248239967731e-24)./(cos(x_3).^4.*3.79080679921875e-6+sin(x_3).^4.*3.79080679921875e-6+cos(x_3).^4.*cos(x_4).^2.*6.757062187003037e-11+cos(x_3).^4.*cos(x_5).^2.*6.757062187003037e-11+cos(x_3).^4.*cos(x_6).^2.*6.757062187003037e-11+cos(x_3).^2.*sin(x_3).^2.*7.5816135984375e-6+cos(x_4).^2.*sin(x_3).^4.*6.757062187003037e-11+cos(x_5).^2.*sin(x_3).^4.*6.757062187003037e-11+cos(x_6).^2.*sin(x_3).^4.*6.757062187003037e-11+cos(x_3).^2.*cos(x_4).^2.*sin(x_3).^2.*1.351412437400607e-10+cos(x_3).^2.*cos(x_5).^2.*sin(x_3).^2.*1.351412437400607e-10+cos(x_3).^2.*cos(x_6).^2.*sin(x_3).^2.*1.351412437400607e-10)-(x_8.*x_9.*cos(x_3).*cos(x_6).*sin(x_3).^4.*sin(x_4).^2.*sin(x_5).^2.*sin(x_6).*1.310151082203454e-24)./(cos(x_3).^4.*3.79080679921875e-6+sin(x_3).^4.*3.79080679921875e-6+cos(x_3).^4.*cos(x_4).^2.*6.757062187003037e-11+cos(x_3).^4.*cos(x_5).^2.*6.757062187003037e-11+cos(x_3).^4.*cos(x_6).^2.*6.757062187003037e-11+cos(x_3).^2.*sin(x_3).^2.*7.5816135984375e-6+cos(x_4).^2.*sin(x_3).^4.*6.757062187003037e-11+cos(x_5).^2.*sin(x_3).^4.*6.757062187003037e-11+cos(x_6).^2.*sin(x_3).^4.*6.757062187003037e-11+cos(x_3).^2.*cos(x_4).^2.*sin(x_3).^2.*1.351412437400607e-10+cos(x_3).^2.*cos(x_5).^2.*sin(x_3).^2.*1.351412437400607e-10+cos(x_3).^2.*cos(x_6).^2.*sin(x_3).^2.*1.351412437400607e-10)+(x_8.*x_9.*cos(x_3).^4.*cos(x_6).*sin(x_3).*sin(x_4).^2.*sin(x_5).^2.*sin(x_6).*2.269248239967731e-24)./(cos(x_3).^4.*3.79080679921875e-6+sin(x_3).^4.*3.79080679921875e-6+cos(x_3).^4.*cos(x_4).^2.*6.757062187003037e-11+cos(x_3).^4.*cos(x_5).^2.*6.757062187003037e-11+cos(x_3).^4.*cos(x_6).^2.*6.757062187003037e-11+cos(x_3).^2.*sin(x_3).^2.*7.5816135984375e-6+cos(x_4).^2.*sin(x_3).^4.*6.757062187003037e-11+cos(x_5).^2.*sin(x_3).^4.*6.757062187003037e-11+cos(x_6).^2.*sin(x_3).^4.*6.757062187003037e-11+cos(x_3).^2.*cos(x_4).^2.*sin(x_3).^2.*1.351412437400607e-10+cos(x_3).^2.*cos(x_5).^2.*sin(x_3).^2.*1.351412437400607e-10+cos(x_3).^2.*cos(x_6).^2.*sin(x_3).^2.*1.351412437400607e-10)-(x_7.*x_9.*cos(x_3).^2.*cos(x_4).*sin(x_3).^3.*sin(x_4).*sin(x_5).^2.*sin(x_6).^2.*5.240604328813817e-24)./(cos(x_3).^4.*3.79080679921875e-6+sin(x_3).^4.*3.79080679921875e-6+cos(x_3).^4.*cos(x_4).^2.*6.757062187003037e-11+cos(x_3).^4.*cos(x_5).^2.*6.757062187003037e-11+cos(x_3).^4.*cos(x_6).^2.*6.757062187003037e-11+cos(x_3).^2.*sin(x_3).^2.*7.5816135984375e-6+cos(x_4).^2.*sin(x_3).^4.*6.757062187003037e-11+cos(x_5).^2.*sin(x_3).^4.*6.757062187003037e-11+cos(x_6).^2.*sin(x_3).^4.*6.757062187003037e-11+cos(x_3).^2.*cos(x_4).^2.*sin(x_3).^2.*1.351412437400607e-10+cos(x_3).^2.*cos(x_5).^2.*sin(x_3).^2.*1.351412437400607e-10+cos(x_3).^2.*cos(x_6).^2.*sin(x_3).^2.*1.351412437400607e-10)+(x_7.*x_9.*cos(x_3).^2.*cos(x_5).*sin(x_3).^3.*sin(x_4).^2.*sin(x_5).*sin(x_6).^2.*2.620302164406908e-24)./(cos(x_3).^4.*3.79080679921875e-6+sin(x_3).^4.*3.79080679921875e-6+cos(x_3).^4.*cos(x_4).^2.*6.757062187003037e-11+cos(x_3).^4.*cos(x_5).^2.*6.757062187003037e-11+cos(x_3).^4.*cos(x_6).^2.*6.757062187003037e-11+cos(x_3).^2.*sin(x_3).^2.*7.5816135984375e-6+cos(x_4).^2.*sin(x_3).^4.*6.757062187003037e-11+cos(x_5).^2.*sin(x_3).^4.*6.757062187003037e-11+cos(x_6).^2.*sin(x_3).^4.*6.757062187003037e-11+cos(x_3).^2.*cos(x_4).^2.*sin(x_3).^2.*1.351412437400607e-10+cos(x_3).^2.*cos(x_5).^2.*sin(x_3).^2.*1.351412437400607e-10+cos(x_3).^2.*cos(x_6).^2.*sin(x_3).^2.*1.351412437400607e-10)-(x_7.*x_9.*cos(x_3).^3.*cos(x_5).*sin(x_3).^2.*sin(x_4).^2.*sin(x_5).*sin(x_6).^2.*4.538496479935463e-24)./(cos(x_3).^4.*3.79080679921875e-6+sin(x_3).^4.*3.79080679921875e-6+cos(x_3).^4.*cos(x_4).^2.*6.757062187003037e-11+cos(x_3).^4.*cos(x_5).^2.*6.757062187003037e-11+cos(x_3).^4.*cos(x_6).^2.*6.757062187003037e-11+cos(x_3).^2.*sin(x_3).^2.*7.5816135984375e-6+cos(x_4).^2.*sin(x_3).^4.*6.757062187003037e-11+cos(x_5).^2.*sin(x_3).^4.*6.757062187003037e-11+cos(x_6).^2.*sin(x_3).^4.*6.757062187003037e-11+cos(x_3).^2.*cos(x_4).^2.*sin(x_3).^2.*1.351412437400607e-10+cos(x_3).^2.*cos(x_5).^2.*sin(x_3).^2.*1.351412437400607e-10+cos(x_3).^2.*cos(x_6).^2.*sin(x_3).^2.*1.351412437400607e-10)+(x_8.*x_9.*cos(x_3).^3.*cos(x_4).*sin(x_3).^2.*sin(x_4).*sin(x_5).^2.*sin(x_6).^2.*5.240604328813817e-24)./(cos(x_3).^4.*3.79080679921875e-6+sin(x_3).^4.*3.79080679921875e-6+cos(x_3).^4.*cos(x_4).^2.*6.757062187003037e-11+cos(x_3).^4.*cos(x_5).^2.*6.757062187003037e-11+cos(x_3).^4.*cos(x_6).^2.*6.757062187003037e-11+cos(x_3).^2.*sin(x_3).^2.*7.5816135984375e-6+cos(x_4).^2.*sin(x_3).^4.*6.757062187003037e-11+cos(x_5).^2.*sin(x_3).^4.*6.757062187003037e-11+cos(x_6).^2.*sin(x_3).^4.*6.757062187003037e-11+cos(x_3).^2.*cos(x_4).^2.*sin(x_3).^2.*1.351412437400607e-10+cos(x_3).^2.*cos(x_5).^2.*sin(x_3).^2.*1.351412437400607e-10+cos(x_3).^2.*cos(x_6).^2.*sin(x_3).^2.*1.351412437400607e-10)+(x_7.*x_9.*cos(x_3).^2.*cos(x_6).*sin(x_3).^3.*sin(x_4).^2.*sin(x_5).^2.*sin(x_6).*2.620302164406908e-24)./(cos(x_3).^4.*3.79080679921875e-6+sin(x_3).^4.*3.79080679921875e-6+cos(x_3).^4.*cos(x_4).^2.*6.757062187003037e-11+cos(x_3).^4.*cos(x_5).^2.*6.757062187003037e-11+cos(x_3).^4.*cos(x_6).^2.*6.757062187003037e-11+cos(x_3).^2.*sin(x_3).^2.*7.5816135984375e-6+cos(x_4).^2.*sin(x_3).^4.*6.757062187003037e-11+cos(x_5).^2.*sin(x_3).^4.*6.757062187003037e-11+cos(x_6).^2.*sin(x_3).^4.*6.757062187003037e-11+cos(x_3).^2.*cos(x_4).^2.*sin(x_3).^2.*1.351412437400607e-10+cos(x_3).^2.*cos(x_5).^2.*sin(x_3).^2.*1.351412437400607e-10+cos(x_3).^2.*cos(x_6).^2.*sin(x_3).^2.*1.351412437400607e-10)+(x_7.*x_9.*cos(x_3).^3.*cos(x_6).*sin(x_3).^2.*sin(x_4).^2.*sin(x_5).^2.*sin(x_6).*4.538496479935463e-24)./(cos(x_3).^4.*3.79080679921875e-6+sin(x_3).^4.*3.79080679921875e-6+cos(x_3).^4.*cos(x_4).^2.*6.757062187003037e-11+cos(x_3).^4.*cos(x_5).^2.*6.757062187003037e-11+cos(x_3).^4.*cos(x_6).^2.*6.757062187003037e-11+cos(x_3).^2.*sin(x_3).^2.*7.5816135984375e-6+cos(x_4).^2.*sin(x_3).^4.*6.757062187003037e-11+cos(x_5).^2.*sin(x_3).^4.*6.757062187003037e-11+cos(x_6).^2.*sin(x_3).^4.*6.757062187003037e-11+cos(x_3).^2.*cos(x_4).^2.*sin(x_3).^2.*1.351412437400607e-10+cos(x_3).^2.*cos(x_5).^2.*sin(x_3).^2.*1.351412437400607e-10+cos(x_3).^2.*cos(x_6).^2.*sin(x_3).^2.*1.351412437400607e-10)-(x_8.*x_9.*cos(x_3).^2.*cos(x_5).*sin(x_3).^3.*sin(x_4).^2.*sin(x_5).*sin(x_6).^2.*4.538496479935463e-24)./(cos(x_3).^4.*3.79080679921875e-6+sin(x_3).^4.*3.79080679921875e-6+cos(x_3).^4.*cos(x_4).^2.*6.757062187003037e-11+cos(x_3).^4.*cos(x_5).^2.*6.757062187003037e-11+cos(x_3).^4.*cos(x_6).^2.*6.757062187003037e-11+cos(x_3).^2.*sin(x_3).^2.*7.5816135984375e-6+cos(x_4).^2.*sin(x_3).^4.*6.757062187003037e-11+cos(x_5).^2.*sin(x_3).^4.*6.757062187003037e-11+cos(x_6).^2.*sin(x_3).^4.*6.757062187003037e-11+cos(x_3).^2.*cos(x_4).^2.*sin(x_3).^2.*1.351412437400607e-10+cos(x_3).^2.*cos(x_5).^2.*sin(x_3).^2.*1.351412437400607e-10+cos(x_3).^2.*cos(x_6).^2.*sin(x_3).^2.*1.351412437400607e-10)-(x_8.*x_9.*cos(x_3).^3.*cos(x_5).*sin(x_3).^2.*sin(x_4).^2.*sin(x_5).*sin(x_6).^2.*2.620302164406908e-24)./(cos(x_3).^4.*3.79080679921875e-6+sin(x_3).^4.*3.79080679921875e-6+cos(x_3).^4.*cos(x_4).^2.*6.757062187003037e-11+cos(x_3).^4.*cos(x_5).^2.*6.757062187003037e-11+cos(x_3).^4.*cos(x_6).^2.*6.757062187003037e-11+cos(x_3).^2.*sin(x_3).^2.*7.5816135984375e-6+cos(x_4).^2.*sin(x_3).^4.*6.757062187003037e-11+cos(x_5).^2.*sin(x_3).^4.*6.757062187003037e-11+cos(x_6).^2.*sin(x_3).^4.*6.757062187003037e-11+cos(x_3).^2.*cos(x_4).^2.*sin(x_3).^2.*1.351412437400607e-10+cos(x_3).^2.*cos(x_5).^2.*sin(x_3).^2.*1.351412437400607e-10+cos(x_3).^2.*cos(x_6).^2.*sin(x_3).^2.*1.351412437400607e-10)+(x_8.*x_9.*cos(x_3).^2.*cos(x_6).*sin(x_3).^3.*sin(x_4).^2.*sin(x_5).^2.*sin(x_6).*4.538496479935463e-24)./(cos(x_3).^4.*3.79080679921875e-6+sin(x_3).^4.*3.79080679921875e-6+cos(x_3).^4.*cos(x_4).^2.*6.757062187003037e-11+cos(x_3).^4.*cos(x_5).^2.*6.757062187003037e-11+cos(x_3).^4.*cos(x_6).^2.*6.757062187003037e-11+cos(x_3).^2.*sin(x_3).^2.*7.5816135984375e-6+cos(x_4).^2.*sin(x_3).^4.*6.757062187003037e-11+cos(x_5).^2.*sin(x_3).^4.*6.757062187003037e-11+cos(x_6).^2.*sin(x_3).^4.*6.757062187003037e-11+cos(x_3).^2.*cos(x_4).^2.*sin(x_3).^2.*1.351412437400607e-10+cos(x_3).^2.*cos(x_5).^2.*sin(x_3).^2.*1.351412437400607e-10+cos(x_3).^2.*cos(x_6).^2.*sin(x_3).^2.*1.351412437400607e-10)-(x_8.*x_9.*cos(x_3).^3.*cos(x_6).*sin(x_3).^2.*sin(x_4).^2.*sin(x_5).^2.*sin(x_6).*2.620302164406908e-24)./(cos(x_3).^4.*3.79080679921875e-6+sin(x_3).^4.*3.79080679921875e-6+cos(x_3).^4.*cos(x_4).^2.*6.757062187003037e-11+cos(x_3).^4.*cos(x_5).^2.*6.757062187003037e-11+cos(x_3).^4.*cos(x_6).^2.*6.757062187003037e-11+cos(x_3).^2.*sin(x_3).^2.*7.5816135984375e-6+cos(x_4).^2.*sin(x_3).^4.*6.757062187003037e-11+cos(x_5).^2.*sin(x_3).^4.*6.757062187003037e-11+cos(x_6).^2.*sin(x_3).^4.*6.757062187003037e-11+cos(x_3).^2.*cos(x_4).^2.*sin(x_3).^2.*1.351412437400607e-10+cos(x_3).^2.*cos(x_5).^2.*sin(x_3).^2.*1.351412437400607e-10+cos(x_3).^2.*cos(x_6).^2.*sin(x_3).^2.*1.351412437400607e-10);(x_9.^2.*cos(x_3).^4.*5.98214987126306e-52)./(cos(x_3).^4.*3.79080679921875e-6+sin(x_3).^4.*3.79080679921875e-6+cos(x_3).^4.*cos(x_4).^2.*6.757062187003037e-11+cos(x_3).^4.*cos(x_5).^2.*6.757062187003037e-11+cos(x_3).^4.*cos(x_6).^2.*6.757062187003037e-11+cos(x_3).^2.*sin(x_3).^2.*7.5816135984375e-6+cos(x_4).^2.*sin(x_3).^4.*6.757062187003037e-11+cos(x_5).^2.*sin(x_3).^4.*6.757062187003037e-11+cos(x_6).^2.*sin(x_3).^4.*6.757062187003037e-11+cos(x_3).^2.*cos(x_4).^2.*sin(x_3).^2.*1.351412437400607e-10+cos(x_3).^2.*cos(x_5).^2.*sin(x_3).^2.*1.351412437400607e-10+cos(x_3).^2.*cos(x_6).^2.*sin(x_3).^2.*1.351412437400607e-10)-(x_9.^2.*cos(x_3).^3.*4.881831459032421e-50)./(cos(x_3).^4.*1.5163227196875e-5+sin(x_3).^4.*1.5163227196875e-5+cos(x_3).^4.*cos(x_4).^2.*2.702824874801215e-10+cos(x_3).^4.*cos(x_5).^2.*2.702824874801215e-10+cos(x_3).^4.*cos(x_6).^2.*2.702824874801215e-10+cos(x_3).^2.*sin(x_3).^2.*3.032645439375e-5+cos(x_4).^2.*sin(x_3).^4.*2.702824874801215e-10+cos(x_5).^2.*sin(x_3).^4.*2.702824874801215e-10+cos(x_6).^2.*sin(x_3).^4.*2.702824874801215e-10+cos(x_3).^2.*cos(x_4).^2.*sin(x_3).^2.*5.40564974960243e-10+cos(x_3).^2.*cos(x_5).^2.*sin(x_3).^2.*5.40564974960243e-10+cos(x_3).^2.*cos(x_6).^2.*sin(x_3).^2.*5.40564974960243e-10)-(x_9.^2.*cos(x_3).^2.*6.326760468668602e-44)./(cos(x_3).^2.*6.49519052838329e-1+sin(x_3).^2.*6.49519052838329e-1)+(x_9.^2.*sin(x_3).^4.*5.98214987126306e-52)./(cos(x_3).^4.*3.79080679921875e-6+sin(x_3).^4.*3.79080679921875e-6+cos(x_3).^4.*cos(x_4).^2.*6.757062187003037e-11+cos(x_3).^4.*cos(x_5).^2.*6.757062187003037e-11+cos(x_3).^4.*cos(x_6).^2.*6.757062187003037e-11+cos(x_3).^2.*sin(x_3).^2.*7.5816135984375e-6+cos(x_4).^2.*sin(x_3).^4.*6.757062187003037e-11+cos(x_5).^2.*sin(x_3).^4.*6.757062187003037e-11+cos(x_6).^2.*sin(x_3).^4.*6.757062187003037e-11+cos(x_3).^2.*cos(x_4).^2.*sin(x_3).^2.*1.351412437400607e-10+cos(x_3).^2.*cos(x_5).^2.*sin(x_3).^2.*1.351412437400607e-10+cos(x_3).^2.*cos(x_6).^2.*sin(x_3).^2.*1.351412437400607e-10)-(x_9.^2.*sin(x_3).^3.*1.308082797032587e-50)./(cos(x_3).^4.*1.5163227196875e-5+sin(x_3).^4.*1.5163227196875e-5+cos(x_3).^4.*cos(x_4).^2.*2.702824874801215e-10+cos(x_3).^4.*cos(x_5).^2.*2.702824874801215e-10+cos(x_3).^4.*cos(x_6).^2.*2.702824874801215e-10+cos(x_3).^2.*sin(x_3).^2.*3.032645439375e-5+cos(x_4).^2.*sin(x_3).^4.*2.702824874801215e-10+cos(x_5).^2.*sin(x_3).^4.*2.702824874801215e-10+cos(x_6).^2.*sin(x_3).^4.*2.702824874801215e-10+cos(x_3).^2.*cos(x_4).^2.*sin(x_3).^2.*5.40564974960243e-10+cos(x_3).^2.*cos(x_5).^2.*sin(x_3).^2.*5.40564974960243e-10+cos(x_3).^2.*cos(x_6).^2.*sin(x_3).^2.*5.40564974960243e-10)-(x_9.^2.*sin(x_3).^2.*6.326760468668602e-44)./(cos(x_3).^2.*6.49519052838329e-1+sin(x_3).^2.*6.49519052838329e-1)+(th_ref.*cos(x_3).^4.*3.808623727011755e-7)./(cos(x_3).^4.*3.628125e-2+sin(x_3).^4.*3.628125e-2+cos(x_3).^2.*sin(x_3).^2.*7.25625e-2)-(th_ref.*cos(x_3).^3.*3.108089821597464e-5)./(cos(x_3).^4.*1.45125e-1+sin(x_3).^4.*1.45125e-1+cos(x_3).^2.*sin(x_3).^2.*2.9025e-1)+(thp_ref.*cos(x_3).^4.*3.808623727011755e-7)./(cos(x_3).^4.*3.628125e-2+sin(x_3).^4.*3.628125e-2+cos(x_3).^2.*sin(x_3).^2.*7.25625e-2)-(thp_ref.*cos(x_3).^3.*3.108089821597464e-5)./(cos(x_3).^4.*1.45125e-1+sin(x_3).^4.*1.45125e-1+cos(x_3).^2.*sin(x_3).^2.*2.9025e-1)+(thpp_ref.*cos(x_3).^4.*9.521559317529389e-8)./(cos(x_3).^4.*3.628125e-2+sin(x_3).^4.*3.628125e-2+cos(x_3).^2.*sin(x_3).^2.*7.25625e-2)-(thpp_ref.*cos(x_3).^3.*7.770224553993659e-6)./(cos(x_3).^4.*1.45125e-1+sin(x_3).^4.*1.45125e-1+cos(x_3).^2.*sin(x_3).^2.*2.9025e-1)-(x_3.*cos(x_3).^4.*3.808623727011755e-7)./(cos(x_3).^4.*3.628125e-2+sin(x_3).^4.*3.628125e-2+cos(x_3).^2.*sin(x_3).^2.*7.25625e-2)-(x_1.*cos(x_3).^3.*1.970449989648948e-5)./(cos(x_3).^4.*1.45125e-1+sin(x_3).^4.*1.45125e-1+cos(x_3).^2.*sin(x_3).^2.*2.9025e-1)+(x_2.*cos(x_3).^3.*1.137639831948516e-5)./(cos(x_3).^4.*1.45125e-1+sin(x_3).^4.*1.45125e-1+cos(x_3).^2.*sin(x_3).^2.*2.9025e-1)+(x_3.*cos(x_3).^3.*3.108089821597464e-5)./(cos(x_3).^4.*1.45125e-1+sin(x_3).^4.*1.45125e-1+cos(x_3).^2.*sin(x_3).^2.*2.9025e-1)-(x_9.*cos(x_3).^4.*3.808623727011755e-7)./(cos(x_3).^4.*3.628125e-2+sin(x_3).^4.*3.628125e-2+cos(x_3).^2.*sin(x_3).^2.*7.25625e-2)-(x_1.*cos(x_3).^2.*5.885754424068536e-4)./(cos(x_3).^4.*5.805e-1+sin(x_3).^4.*5.805e-1+cos(x_3).^2.*sin(x_3).^2.*1.161)+(x_2.*cos(x_3).^2.*8.373366947017072e-4)./(cos(x_3).^4.*5.805e-1+sin(x_3).^4.*5.805e-1+cos(x_3).^2.*sin(x_3).^2.*1.161)-(x_7.*cos(x_3).^3.*1.970449989648948e-5)./(cos(x_3).^4.*1.45125e-1+sin(x_3).^4.*1.45125e-1+cos(x_3).^2.*sin(x_3).^2.*2.9025e-1)+(x_8.*cos(x_3).^3.*1.137639831948516e-5)./(cos(x_3).^4.*1.45125e-1+sin(x_3).^4.*1.45125e-1+cos(x_3).^2.*sin(x_3).^2.*2.9025e-1)+(x_9.*cos(x_3).^3.*3.108089821597464e-5)./(cos(x_3).^4.*1.45125e-1+sin(x_3).^4.*1.45125e-1+cos(x_3).^2.*sin(x_3).^2.*2.9025e-1)-(x_7.*cos(x_3).^2.*5.885754424068536e-4)./(cos(x_3).^4.*5.805e-1+sin(x_3).^4.*5.805e-1+cos(x_3).^2.*sin(x_3).^2.*1.161)+(x_8.*cos(x_3).^2.*8.373366947017072e-4)./(cos(x_3).^4.*5.805e-1+sin(x_3).^4.*5.805e-1+cos(x_3).^2.*sin(x_3).^2.*1.161)+(x_ref.*cos(x_3).^3.*1.970449989648948e-5)./(cos(x_3).^4.*1.45125e-1+sin(x_3).^4.*1.45125e-1+cos(x_3).^2.*sin(x_3).^2.*2.9025e-1)+(x_ref.*cos(x_3).^2.*5.885754424068536e-4)./(cos(x_3).^4.*5.805e-1+sin(x_3).^4.*5.805e-1+cos(x_3).^2.*sin(x_3).^2.*1.161)+(xp_ref.*cos(x_3).^3.*1.970449989648948e-5)./(cos(x_3).^4.*1.45125e-1+sin(x_3).^4.*1.45125e-1+cos(x_3).^2.*sin(x_3).^2.*2.9025e-1)+(xp_ref.*cos(x_3).^2.*5.885754424068536e-4)./(cos(x_3).^4.*5.805e-1+sin(x_3).^4.*5.805e-1+cos(x_3).^2.*sin(x_3).^2.*1.161)+(xpp_ref.*cos(x_3).^3.*4.92612497412237e-6)./(cos(x_3).^4.*1.45125e-1+sin(x_3).^4.*1.45125e-1+cos(x_3).^2.*sin(x_3).^2.*2.9025e-1)+(xpp_ref.*cos(x_3).^2.*1.471438606017134e-4)./(cos(x_3).^4.*5.805e-1+sin(x_3).^4.*5.805e-1+cos(x_3).^2.*sin(x_3).^2.*1.161)-(y_ref.*cos(x_3).^3.*1.137639831948516e-5)./(cos(x_3).^4.*1.45125e-1+sin(x_3).^4.*1.45125e-1+cos(x_3).^2.*sin(x_3).^2.*2.9025e-1)-(y_ref.*cos(x_3).^2.*8.373366947017072e-4)./(cos(x_3).^4.*5.805e-1+sin(x_3).^4.*5.805e-1+cos(x_3).^2.*sin(x_3).^2.*1.161)-(yp_ref.*cos(x_3).^3.*1.137639831948516e-5)./(cos(x_3).^4.*1.45125e-1+sin(x_3).^4.*1.45125e-1+cos(x_3).^2.*sin(x_3).^2.*2.9025e-1)-(yp_ref.*cos(x_3).^2.*8.373366947017072e-4)./(cos(x_3).^4.*5.805e-1+sin(x_3).^4.*5.805e-1+cos(x_3).^2.*sin(x_3).^2.*1.161)-(ypp_ref.*cos(x_3).^3.*2.844099579871289e-6)./(cos(x_3).^4.*1.45125e-1+sin(x_3).^4.*1.45125e-1+cos(x_3).^2.*sin(x_3).^2.*2.9025e-1)-(ypp_ref.*cos(x_3).^2.*2.093341736754268e-4)./(cos(x_3).^4.*5.805e-1+sin(x_3).^4.*5.805e-1+cos(x_3).^2.*sin(x_3).^2.*1.161)+(th_ref.*sin(x_3).^4.*3.808623727011755e-7)./(cos(x_3).^4.*3.628125e-2+sin(x_3).^4.*3.628125e-2+cos(x_3).^2.*sin(x_3).^2.*7.25625e-2)-(th_ref.*sin(x_3).^3.*8.328101577004326e-6)./(cos(x_3).^4.*1.45125e-1+sin(x_3).^4.*1.45125e-1+cos(x_3).^2.*sin(x_3).^2.*2.9025e-1)+(thp_ref.*sin(x_3).^4.*3.808623727011755e-7)./(cos(x_3).^4.*3.628125e-2+sin(x_3).^4.*3.628125e-2+cos(x_3).^2.*sin(x_3).^2.*7.25625e-2)-(thp_ref.*sin(x_3).^3.*8.328101577004326e-6)./(cos(x_3).^4.*1.45125e-1+sin(x_3).^4.*1.45125e-1+cos(x_3).^2.*sin(x_3).^2.*2.9025e-1)+(thpp_ref.*sin(x_3).^4.*9.521559317529389e-8)./(cos(x_3).^4.*3.628125e-2+sin(x_3).^4.*3.628125e-2+cos(x_3).^2.*sin(x_3).^2.*7.25625e-2)-(thpp_ref.*sin(x_3).^3.*2.082025394251082e-6)./(cos(x_3).^4.*1.45125e-1+sin(x_3).^4.*1.45125e-1+cos(x_3).^2.*sin(x_3).^2.*2.9025e-1)-(x_3.*sin(x_3).^4.*3.808623727011755e-7)./(cos(x_3).^4.*3.628125e-2+sin(x_3).^4.*3.628125e-2+cos(x_3).^2.*sin(x_3).^2.*7.25625e-2)-(x_1.*sin(x_3).^3.*1.137639831948516e-5)./(cos(x_3).^4.*1.45125e-1+sin(x_3).^4.*1.45125e-1+cos(x_3).^2.*sin(x_3).^2.*2.9025e-1)-(x_2.*sin(x_3).^3.*1.970449989648948e-5)./(cos(x_3).^4.*1.45125e-1+sin(x_3).^4.*1.45125e-1+cos(x_3).^2.*sin(x_3).^2.*2.9025e-1)+(x_3.*sin(x_3).^3.*8.328101577004326e-6)./(cos(x_3).^4.*1.45125e-1+sin(x_3).^4.*1.45125e-1+cos(x_3).^2.*sin(x_3).^2.*2.9025e-1)-(x_9.*sin(x_3).^4.*3.808623727011755e-7)./(cos(x_3).^4.*3.628125e-2+sin(x_3).^4.*3.628125e-2+cos(x_3).^2.*sin(x_3).^2.*7.25625e-2)+(x_1.*sin(x_3).^2.*1.268203822630854e-3)./(cos(x_3).^4.*5.805e-1+sin(x_3).^4.*5.805e-1+cos(x_3).^2.*sin(x_3).^2.*1.161)-(x_2.*sin(x_3).^2.*1.019442570336e-3)./(cos(x_3).^4.*5.805e-1+sin(x_3).^4.*5.805e-1+cos(x_3).^2.*sin(x_3).^2.*1.161)-(x_7.*sin(x_3).^3.*1.137639831948516e-5)./(cos(x_3).^4.*1.45125e-1+sin(x_3).^4.*1.45125e-1+cos(x_3).^2.*sin(x_3).^2.*2.9025e-1)-(x_8.*sin(x_3).^3.*1.970449989648948e-5)./(cos(x_3).^4.*1.45125e-1+sin(x_3).^4.*1.45125e-1+cos(x_3).^2.*sin(x_3).^2.*2.9025e-1)+(x_9.*sin(x_3).^3.*8.328101577004326e-6)./(cos(x_3).^4.*1.45125e-1+sin(x_3).^4.*1.45125e-1+cos(x_3).^2.*sin(x_3).^2.*2.9025e-1)+(x_7.*sin(x_3).^2.*1.268203822630854e-3)./(cos(x_3).^4.*5.805e-1+sin(x_3).^4.*5.805e-1+cos(x_3).^2.*sin(x_3).^2.*1.161)-(x_8.*sin(x_3).^2.*1.019442570336e-3)./(cos(x_3).^4.*5.805e-1+sin(x_3).^4.*5.805e-1+cos(x_3).^2.*sin(x_3).^2.*1.161)+(x_ref.*sin(x_3).^3.*1.137639831948516e-5)./(cos(x_3).^4.*1.45125e-1+sin(x_3).^4.*1.45125e-1+cos(x_3).^2.*sin(x_3).^2.*2.9025e-1)-(x_ref.*sin(x_3).^2.*1.268203822630854e-3)./(cos(x_3).^4.*5.805e-1+sin(x_3).^4.*5.805e-1+cos(x_3).^2.*sin(x_3).^2.*1.161)+(xp_ref.*sin(x_3).^3.*1.137639831948516e-5)./(cos(x_3).^4.*1.45125e-1+sin(x_3).^4.*1.45125e-1+cos(x_3).^2.*sin(x_3).^2.*2.9025e-1)-(xp_ref.*sin(x_3).^2.*1.268203822630854e-3)./(cos(x_3).^4.*5.805e-1+sin(x_3).^4.*5.805e-1+cos(x_3).^2.*sin(x_3).^2.*1.161)+(xpp_ref.*sin(x_3).^3.*2.844099579871289e-6)./(cos(x_3).^4.*1.45125e-1+sin(x_3).^4.*1.45125e-1+cos(x_3).^2.*sin(x_3).^2.*2.9025e-1)-(xpp_ref.*sin(x_3).^2.*3.170509556577134e-4)./(cos(x_3).^4.*5.805e-1+sin(x_3).^4.*5.805e-1+cos(x_3).^2.*sin(x_3).^2.*1.161)+(y_ref.*sin(x_3).^3.*1.970449989648948e-5)./(cos(x_3).^4.*1.45125e-1+sin(x_3).^4.*1.45125e-1+cos(x_3).^2.*sin(x_3).^2.*2.9025e-1)+(y_ref.*sin(x_3).^2.*1.019442570336e-3)./(cos(x_3).^4.*5.805e-1+sin(x_3).^4.*5.805e-1+cos(x_3).^2.*sin(x_3).^2.*1.161)+(yp_ref.*sin(x_3).^3.*1.970449989648948e-5)./(cos(x_3).^4.*1.45125e-1+sin(x_3).^4.*1.45125e-1+cos(x_3).^2.*sin(x_3).^2.*2.9025e-1)+(yp_ref.*sin(x_3).^2.*1.019442570336e-3)./(cos(x_3).^4.*5.805e-1+sin(x_3).^4.*5.805e-1+cos(x_3).^2.*sin(x_3).^2.*1.161)+(ypp_ref.*sin(x_3).^3.*4.92612497412237e-6)./(cos(x_3).^4.*1.45125e-1+sin(x_3).^4.*1.45125e-1+cos(x_3).^2.*sin(x_3).^2.*2.9025e-1)+(ypp_ref.*sin(x_3).^2.*2.54860642584e-4)./(cos(x_3).^4.*5.805e-1+sin(x_3).^4.*5.805e-1+cos(x_3).^2.*sin(x_3).^2.*1.161)+(th_ref.*cos(x_3).^2.*sin(x_3).^2.*7.617247454023511e-7)./(cos(x_3).^4.*3.628125e-2+sin(x_3).^4.*3.628125e-2+cos(x_3).^2.*sin(x_3).^2.*7.25625e-2)-(th_ref.*cos(x_3).^4.*sin(x_4).^2.*1.357691522274898e-11)./(cos(x_3).^4.*3.628125e-2+sin(x_3).^4.*3.628125e-2+cos(x_3).^2.*sin(x_3).^2.*7.25625e-2)-(th_ref.*cos(x_3).^4.*sin(x_5).^2.*1.357691522274898e-11)./(cos(x_3).^4.*3.628125e-2+sin(x_3).^4.*3.628125e-2+cos(x_3).^2.*sin(x_3).^2.*7.25625e-2)+(th_ref.*cos(x_3).^4.*sin(x_4).^4.*1.209968745785898e-16)./(cos(x_3).^4.*3.628125e-2+sin(x_3).^4.*3.628125e-2+cos(x_3).^2.*sin(x_3).^2.*7.25625e-2)-(th_ref.*cos(x_3).^4.*sin(x_6).^2.*1.357691522274898e-11)./(cos(x_3).^4.*3.628125e-2+sin(x_3).^4.*3.628125e-2+cos(x_3).^2.*sin(x_3).^2.*7.25625e-2)+(th_ref.*cos(x_3).^4.*sin(x_5).^4.*1.209968745785898e-16)./(cos(x_3).^4.*3.628125e-2+sin(x_3).^4.*3.628125e-2+cos(x_3).^2.*sin(x_3).^2.*7.25625e-2)+(th_ref.*cos(x_3).^4.*sin(x_6).^4.*1.209968745785898e-16)./(cos(x_3).^4.*3.628125e-2+sin(x_3).^4.*3.628125e-2+cos(x_3).^2.*sin(x_3).^2.*7.25625e-2)+(th_ref.*cos(x_3).^3.*sin(x_4).^2.*5.539832106967747e-10)./(cos(x_3).^4.*1.45125e-1+sin(x_3).^4.*1.45125e-1+cos(x_3).^2.*sin(x_3).^2.*2.9025e-1)+(th_ref.*cos(x_3).^3.*sin(x_5).^2.*5.539832106967747e-10)./(cos(x_3).^4.*1.45125e-1+sin(x_3).^4.*1.45125e-1+cos(x_3).^2.*sin(x_3).^2.*2.9025e-1)+(th_ref.*cos(x_3).^3.*sin(x_6).^2.*5.539832106967747e-10)./(cos(x_3).^4.*1.45125e-1+sin(x_3).^4.*1.45125e-1+cos(x_3).^2.*sin(x_3).^2.*2.9025e-1)+(thp_ref.*cos(x_3).^2.*sin(x_3).^2.*7.617247454023511e-7)./(cos(x_3).^4.*3.628125e-2+sin(x_3).^4.*3.628125e-2+cos(x_3).^2.*sin(x_3).^2.*7.25625e-2)-(thp_ref.*cos(x_3).^4.*sin(x_4).^2.*1.357691522274898e-11)./(cos(x_3).^4.*3.628125e-2+sin(x_3).^4.*3.628125e-2+cos(x_3).^2.*sin(x_3).^2.*7.25625e-2)-(thp_ref.*cos(x_3).^4.*sin(x_5).^2.*1.357691522274898e-11)./(cos(x_3).^4.*3.628125e-2+sin(x_3).^4.*3.628125e-2+cos(x_3).^2.*sin(x_3).^2.*7.25625e-2)+(thp_ref.*cos(x_3).^4.*sin(x_4).^4.*1.209968745785898e-16)./(cos(x_3).^4.*3.628125e-2+sin(x_3).^4.*3.628125e-2+cos(x_3).^2.*sin(x_3).^2.*7.25625e-2)-(thp_ref.*cos(x_3).^4.*sin(x_6).^2.*1.357691522274898e-11)./(cos(x_3).^4.*3.628125e-2+sin(x_3).^4.*3.628125e-2+cos(x_3).^2.*sin(x_3).^2.*7.25625e-2)+(thp_ref.*cos(x_3).^4.*sin(x_5).^4.*1.209968745785898e-16)./(cos(x_3).^4.*3.628125e-2+sin(x_3).^4.*3.628125e-2+cos(x_3).^2.*sin(x_3).^2.*7.25625e-2)+(thp_ref.*cos(x_3).^4.*sin(x_6).^4.*1.209968745785898e-16)./(cos(x_3).^4.*3.628125e-2+sin(x_3).^4.*3.628125e-2+cos(x_3).^2.*sin(x_3).^2.*7.25625e-2)+(thp_ref.*cos(x_3).^3.*sin(x_4).^2.*5.539832106967747e-10)./(cos(x_3).^4.*1.45125e-1+sin(x_3).^4.*1.45125e-1+cos(x_3).^2.*sin(x_3).^2.*2.9025e-1)+(thp_ref.*cos(x_3).^3.*sin(x_5).^2.*5.539832106967747e-10)./(cos(x_3).^4.*1.45125e-1+sin(x_3).^4.*1.45125e-1+cos(x_3).^2.*sin(x_3).^2.*2.9025e-1)+(thp_ref.*cos(x_3).^3.*sin(x_6).^2.*5.539832106967747e-10)./(cos(x_3).^4.*1.45125e-1+sin(x_3).^4.*1.45125e-1+cos(x_3).^2.*sin(x_3).^2.*2.9025e-1)+(thpp_ref.*cos(x_3).^2.*sin(x_3).^2.*1.904311863505878e-7)./(cos(x_3).^4.*3.628125e-2+sin(x_3).^4.*3.628125e-2+cos(x_3).^2.*sin(x_3).^2.*7.25625e-2)-(thpp_ref.*cos(x_3).^4.*sin(x_4).^2.*3.394228805687245e-12)./(cos(x_3).^4.*3.628125e-2+sin(x_3).^4.*3.628125e-2+cos(x_3).^2.*sin(x_3).^2.*7.25625e-2)-(thpp_ref.*cos(x_3).^4.*sin(x_5).^2.*3.394228805687245e-12)./(cos(x_3).^4.*3.628125e-2+sin(x_3).^4.*3.628125e-2+cos(x_3).^2.*sin(x_3).^2.*7.25625e-2)+(thpp_ref.*cos(x_3).^4.*sin(x_4).^4.*3.024921864464745e-17)./(cos(x_3).^4.*3.628125e-2+sin(x_3).^4.*3.628125e-2+cos(x_3).^2.*sin(x_3).^2.*7.25625e-2)-(thpp_ref.*cos(x_3).^4.*sin(x_6).^2.*3.394228805687245e-12)./(cos(x_3).^4.*3.628125e-2+sin(x_3).^4.*3.628125e-2+cos(x_3).^2.*sin(x_3).^2.*7.25625e-2)+(thpp_ref.*cos(x_3).^4.*sin(x_5).^4.*3.024921864464745e-17)./(cos(x_3).^4.*3.628125e-2+sin(x_3).^4.*3.628125e-2+cos(x_3).^2.*sin(x_3).^2.*7.25625e-2)+(thpp_ref.*cos(x_3).^4.*sin(x_6).^4.*3.024921864464745e-17)./(cos(x_3).^4.*3.628125e-2+sin(x_3).^4.*3.628125e-2+cos(x_3).^2.*sin(x_3).^2.*7.25625e-2)+(thpp_ref.*cos(x_3).^3.*sin(x_4).^2.*1.384958026741937e-10)./(cos(x_3).^4.*1.45125e-1+sin(x_3).^4.*1.45125e-1+cos(x_3).^2.*sin(x_3).^2.*2.9025e-1)+(thpp_ref.*cos(x_3).^3.*sin(x_5).^2.*1.384958026741937e-10)./(cos(x_3).^4.*1.45125e-1+sin(x_3).^4.*1.45125e-1+cos(x_3).^2.*sin(x_3).^2.*2.9025e-1)+(thpp_ref.*cos(x_3).^3.*sin(x_6).^2.*1.384958026741937e-10)./(cos(x_3).^4.*1.45125e-1+sin(x_3).^4.*1.45125e-1+cos(x_3).^2.*sin(x_3).^2.*2.9025e-1)-(x_3.*cos(x_3).^2.*sin(x_3).^2.*7.617247454023511e-7)./(cos(x_3).^4.*3.628125e-2+sin(x_3).^4.*3.628125e-2+cos(x_3).^2.*sin(x_3).^2.*7.25625e-2)+(x_3.*cos(x_3).^4.*sin(x_4).^2.*1.357691522274898e-11)./(cos(x_3).^4.*3.628125e-2+sin(x_3).^4.*3.628125e-2+cos(x_3).^2.*sin(x_3).^2.*7.25625e-2)+(x_3.*cos(x_3).^4.*sin(x_5).^2.*1.357691522274898e-11)./(cos(x_3).^4.*3.628125e-2+sin(x_3).^4.*3.628125e-2+cos(x_3).^2.*sin(x_3).^2.*7.25625e-2)-(x_3.*cos(x_3).^4.*sin(x_4).^4.*1.209968745785898e-16)./(cos(x_3).^4.*3.628125e-2+sin(x_3).^4.*3.628125e-2+cos(x_3).^2.*sin(x_3).^2.*7.25625e-2)+(x_3.*cos(x_3).^4.*sin(x_6).^2.*1.357691522274898e-11)./(cos(x_3).^4.*3.628125e-2+sin(x_3).^4.*3.628125e-2+cos(x_3).^2.*sin(x_3).^2.*7.25625e-2)+(x_1.*cos(x_3).^3.*sin(x_4).^2.*3.51211282311688e-10)./(cos(x_3).^4.*1.45125e-1+sin(x_3).^4.*1.45125e-1+cos(x_3).^2.*sin(x_3).^2.*2.9025e-1)-(x_3.*cos(x_3).^4.*sin(x_5).^4.*1.209968745785898e-16)./(cos(x_3).^4.*3.628125e-2+sin(x_3).^4.*3.628125e-2+cos(x_3).^2.*sin(x_3).^2.*7.25625e-2)-(x_9.*cos(x_3).^2.*sin(x_3).^2.*7.617247454023511e-7)./(cos(x_3).^4.*3.628125e-2+sin(x_3).^4.*3.628125e-2+cos(x_3).^2.*sin(x_3).^2.*7.25625e-2)+(x_1.*cos(x_3).^3.*sin(x_5).^2.*3.51211282311688e-10)./(cos(x_3).^4.*1.45125e-1+sin(x_3).^4.*1.45125e-1+cos(x_3).^2.*sin(x_3).^2.*2.9025e-1)-(x_2.*cos(x_3).^3.*sin(x_4).^2.*2.027719283850867e-10)./(cos(x_3).^4.*1.45125e-1+sin(x_3).^4.*1.45125e-1+cos(x_3).^2.*sin(x_3).^2.*2.9025e-1)-(x_3.*cos(x_3).^4.*sin(x_6).^4.*1.209968745785898e-16)./(cos(x_3).^4.*3.628125e-2+sin(x_3).^4.*3.628125e-2+cos(x_3).^2.*sin(x_3).^2.*7.25625e-2)+(x_1.*cos(x_3).^3.*sin(x_6).^2.*3.51211282311688e-10)./(cos(x_3).^4.*1.45125e-1+sin(x_3).^4.*1.45125e-1+cos(x_3).^2.*sin(x_3).^2.*2.9025e-1)-(x_2.*cos(x_3).^3.*sin(x_5).^2.*2.027719283850867e-10)./(cos(x_3).^4.*1.45125e-1+sin(x_3).^4.*1.45125e-1+cos(x_3).^2.*sin(x_3).^2.*2.9025e-1)-(x_3.*cos(x_3).^3.*sin(x_4).^2.*5.539832106967747e-10)./(cos(x_3).^4.*1.45125e-1+sin(x_3).^4.*1.45125e-1+cos(x_3).^2.*sin(x_3).^2.*2.9025e-1)-(x_2.*cos(x_3).^3.*sin(x_6).^2.*2.027719283850867e-10)./(cos(x_3).^4.*1.45125e-1+sin(x_3).^4.*1.45125e-1+cos(x_3).^2.*sin(x_3).^2.*2.9025e-1)-(x_3.*cos(x_3).^3.*sin(x_5).^2.*5.539832106967747e-10)./(cos(x_3).^4.*1.45125e-1+sin(x_3).^4.*1.45125e-1+cos(x_3).^2.*sin(x_3).^2.*2.9025e-1)+(x_9.*cos(x_3).^4.*sin(x_4).^2.*1.357691522274898e-11)./(cos(x_3).^4.*3.628125e-2+sin(x_3).^4.*3.628125e-2+cos(x_3).^2.*sin(x_3).^2.*7.25625e-2)-(x_3.*cos(x_3).^3.*sin(x_6).^2.*5.539832106967747e-10)./(cos(x_3).^4.*1.45125e-1+sin(x_3).^4.*1.45125e-1+cos(x_3).^2.*sin(x_3).^2.*2.9025e-1)+(x_9.*cos(x_3).^4.*sin(x_5).^2.*1.357691522274898e-11)./(cos(x_3).^4.*3.628125e-2+sin(x_3).^4.*3.628125e-2+cos(x_3).^2.*sin(x_3).^2.*7.25625e-2)-(x_9.*cos(x_3).^4.*sin(x_4).^4.*1.209968745785898e-16)./(cos(x_3).^4.*3.628125e-2+sin(x_3).^4.*3.628125e-2+cos(x_3).^2.*sin(x_3).^2.*7.25625e-2)+(x_9.*cos(x_3).^4.*sin(x_6).^2.*1.357691522274898e-11)./(cos(x_3).^4.*3.628125e-2+sin(x_3).^4.*3.628125e-2+cos(x_3).^2.*sin(x_3).^2.*7.25625e-2)+(x_7.*cos(x_3).^3.*sin(x_4).^2.*3.51211282311688e-10)./(cos(x_3).^4.*1.45125e-1+sin(x_3).^4.*1.45125e-1+cos(x_3).^2.*sin(x_3).^2.*2.9025e-1)-(x_9.*cos(x_3).^4.*sin(x_5).^4.*1.209968745785898e-16)./(cos(x_3).^4.*3.628125e-2+sin(x_3).^4.*3.628125e-2+cos(x_3).^2.*sin(x_3).^2.*7.25625e-2)+(x_7.*cos(x_3).^3.*sin(x_5).^2.*3.51211282311688e-10)./(cos(x_3).^4.*1.45125e-1+sin(x_3).^4.*1.45125e-1+cos(x_3).^2.*sin(x_3).^2.*2.9025e-1)-(x_8.*cos(x_3).^3.*sin(x_4).^2.*2.027719283850867e-10)./(cos(x_3).^4.*1.45125e-1+sin(x_3).^4.*1.45125e-1+cos(x_3).^2.*sin(x_3).^2.*2.9025e-1)-(x_9.*cos(x_3).^4.*sin(x_6).^4.*1.209968745785898e-16)./(cos(x_3).^4.*3.628125e-2+sin(x_3).^4.*3.628125e-2+cos(x_3).^2.*sin(x_3).^2.*7.25625e-2)+(x_7.*cos(x_3).^3.*sin(x_6).^2.*3.51211282311688e-10)./(cos(x_3).^4.*1.45125e-1+sin(x_3).^4.*1.45125e-1+cos(x_3).^2.*sin(x_3).^2.*2.9025e-1)-(x_8.*cos(x_3).^3.*sin(x_5).^2.*2.027719283850867e-10)./(cos(x_3).^4.*1.45125e-1+sin(x_3).^4.*1.45125e-1+cos(x_3).^2.*sin(x_3).^2.*2.9025e-1)-(x_9.*cos(x_3).^3.*sin(x_4).^2.*5.539832106967747e-10)./(cos(x_3).^4.*1.45125e-1+sin(x_3).^4.*1.45125e-1+cos(x_3).^2.*sin(x_3).^2.*2.9025e-1)-(x_8.*cos(x_3).^3.*sin(x_6).^2.*2.027719283850867e-10)./(cos(x_3).^4.*1.45125e-1+sin(x_3).^4.*1.45125e-1+cos(x_3).^2.*sin(x_3).^2.*2.9025e-1)-(x_9.*cos(x_3).^3.*sin(x_5).^2.*5.539832106967747e-10)./(cos(x_3).^4.*1.45125e-1+sin(x_3).^4.*1.45125e-1+cos(x_3).^2.*sin(x_3).^2.*2.9025e-1)-(x_9.*cos(x_3).^3.*sin(x_6).^2.*5.539832106967747e-10)./(cos(x_3).^4.*1.45125e-1+sin(x_3).^4.*1.45125e-1+cos(x_3).^2.*sin(x_3).^2.*2.9025e-1)-(x_ref.*cos(x_3).^3.*sin(x_4).^2.*3.51211282311688e-10)./(cos(x_3).^4.*1.45125e-1+sin(x_3).^4.*1.45125e-1+cos(x_3).^2.*sin(x_3).^2.*2.9025e-1)-(x_ref.*cos(x_3).^3.*sin(x_5).^2.*3.51211282311688e-10)./(cos(x_3).^4.*1.45125e-1+sin(x_3).^4.*1.45125e-1+cos(x_3).^2.*sin(x_3).^2.*2.9025e-1)-(x_ref.*cos(x_3).^3.*sin(x_6).^2.*3.51211282311688e-10)./(cos(x_3).^4.*1.45125e-1+sin(x_3).^4.*1.45125e-1+cos(x_3).^2.*sin(x_3).^2.*2.9025e-1)-(xp_ref.*cos(x_3).^3.*sin(x_4).^2.*3.51211282311688e-10)./(cos(x_3).^4.*1.45125e-1+sin(x_3).^4.*1.45125e-1+cos(x_3).^2.*sin(x_3).^2.*2.9025e-1)-(xp_ref.*cos(x_3).^3.*sin(x_5).^2.*3.51211282311688e-10)./(cos(x_3).^4.*1.45125e-1+sin(x_3).^4.*1.45125e-1+cos(x_3).^2.*sin(x_3).^2.*2.9025e-1)-(xp_ref.*cos(x_3).^3.*sin(x_6).^2.*3.51211282311688e-10)./(cos(x_3).^4.*1.45125e-1+sin(x_3).^4.*1.45125e-1+cos(x_3).^2.*sin(x_3).^2.*2.9025e-1)-(xpp_ref.*cos(x_3).^3.*sin(x_4).^2.*8.780282057792199e-11)./(cos(x_3).^4.*1.45125e-1+sin(x_3).^4.*1.45125e-1+cos(x_3).^2.*sin(x_3).^2.*2.9025e-1)-(xpp_ref.*cos(x_3).^3.*sin(x_5).^2.*8.780282057792199e-11)./(cos(x_3).^4.*1.45125e-1+sin(x_3).^4.*1.45125e-1+cos(x_3).^2.*sin(x_3).^2.*2.9025e-1)-(xpp_ref.*cos(x_3).^3.*sin(x_6).^2.*8.780282057792199e-11)./(cos(x_3).^4.*1.45125e-1+sin(x_3).^4.*1.45125e-1+cos(x_3).^2.*sin(x_3).^2.*2.9025e-1)+(y_ref.*cos(x_3).^3.*sin(x_4).^2.*2.027719283850867e-10)./(cos(x_3).^4.*1.45125e-1+sin(x_3).^4.*1.45125e-1+cos(x_3).^2.*sin(x_3).^2.*2.9025e-1)+(y_ref.*cos(x_3).^3.*sin(x_5).^2.*2.027719283850867e-10)./(cos(x_3).^4.*1.45125e-1+sin(x_3).^4.*1.45125e-1+cos(x_3).^2.*sin(x_3).^2.*2.9025e-1)+(y_ref.*cos(x_3).^3.*sin(x_6).^2.*2.027719283850867e-10)./(cos(x_3).^4.*1.45125e-1+sin(x_3).^4.*1.45125e-1+cos(x_3).^2.*sin(x_3).^2.*2.9025e-1)+(yp_ref.*cos(x_3).^3.*sin(x_4).^2.*2.027719283850867e-10)./(cos(x_3).^4.*1.45125e-1+sin(x_3).^4.*1.45125e-1+cos(x_3).^2.*sin(x_3).^2.*2.9025e-1)+(yp_ref.*cos(x_3).^3.*sin(x_5).^2.*2.027719283850867e-10)./(cos(x_3).^4.*1.45125e-1+sin(x_3).^4.*1.45125e-1+cos(x_3).^2.*sin(x_3).^2.*2.9025e-1)+(yp_ref.*cos(x_3).^3.*sin(x_6).^2.*2.027719283850867e-10)./(cos(x_3).^4.*1.45125e-1+sin(x_3).^4.*1.45125e-1+cos(x_3).^2.*sin(x_3).^2.*2.9025e-1)+(ypp_ref.*cos(x_3).^3.*sin(x_4).^2.*5.069298209627167e-11)./(cos(x_3).^4.*1.45125e-1+sin(x_3).^4.*1.45125e-1+cos(x_3).^2.*sin(x_3).^2.*2.9025e-1)+(ypp_ref.*cos(x_3).^3.*sin(x_5).^2.*5.069298209627167e-11)./(cos(x_3).^4.*1.45125e-1+sin(x_3).^4.*1.45125e-1+cos(x_3).^2.*sin(x_3).^2.*2.9025e-1)+(ypp_ref.*cos(x_3).^3.*sin(x_6).^2.*5.069298209627167e-11)./(cos(x_3).^4.*1.45125e-1+sin(x_3).^4.*1.45125e-1+cos(x_3).^2.*sin(x_3).^2.*2.9025e-1)-(th_ref.*sin(x_3).^4.*sin(x_4).^2.*1.357691522274898e-11)./(cos(x_3).^4.*3.628125e-2+sin(x_3).^4.*3.628125e-2+cos(x_3).^2.*sin(x_3).^2.*7.25625e-2)-(th_ref.*sin(x_3).^4.*sin(x_5).^2.*1.357691522274898e-11)./(cos(x_3).^4.*3.628125e-2+sin(x_3).^4.*3.628125e-2+cos(x_3).^2.*sin(x_3).^2.*7.25625e-2)+(th_ref.*sin(x_3).^4.*sin(x_4).^4.*1.209968745785898e-16)./(cos(x_3).^4.*3.628125e-2+sin(x_3).^4.*3.628125e-2+cos(x_3).^2.*sin(x_3).^2.*7.25625e-2)-(th_ref.*sin(x_3).^4.*sin(x_6).^2.*1.357691522274898e-11)./(cos(x_3).^4.*3.628125e-2+sin(x_3).^4.*3.628125e-2+cos(x_3).^2.*sin(x_3).^2.*7.25625e-2)+(th_ref.*sin(x_3).^4.*sin(x_5).^4.*1.209968745785898e-16)./(cos(x_3).^4.*3.628125e-2+sin(x_3).^4.*3.628125e-2+cos(x_3).^2.*sin(x_3).^2.*7.25625e-2)+(th_ref.*sin(x_3).^4.*sin(x_6).^4.*1.209968745785898e-16)./(cos(x_3).^4.*3.628125e-2+sin(x_3).^4.*3.628125e-2+cos(x_3).^2.*sin(x_3).^2.*7.25625e-2)+(th_ref.*sin(x_3).^3.*sin(x_4).^2.*1.484393539266013e-10)./(cos(x_3).^4.*1.45125e-1+sin(x_3).^4.*1.45125e-1+cos(x_3).^2.*sin(x_3).^2.*2.9025e-1)+(th_ref.*sin(x_3).^3.*sin(x_5).^2.*1.484393539266013e-10)./(cos(x_3).^4.*1.45125e-1+sin(x_3).^4.*1.45125e-1+cos(x_3).^2.*sin(x_3).^2.*2.9025e-1)+(th_ref.*sin(x_3).^3.*sin(x_6).^2.*1.484393539266013e-10)./(cos(x_3).^4.*1.45125e-1+sin(x_3).^4.*1.45125e-1+cos(x_3).^2.*sin(x_3).^2.*2.9025e-1)-(thp_ref.*sin(x_3).^4.*sin(x_4).^2.*1.357691522274898e-11)./(cos(x_3).^4.*3.628125e-2+sin(x_3).^4.*3.628125e-2+cos(x_3).^2.*sin(x_3).^2.*7.25625e-2)-(thp_ref.*sin(x_3).^4.*sin(x_5).^2.*1.357691522274898e-11)./(cos(x_3).^4.*3.628125e-2+sin(x_3).^4.*3.628125e-2+cos(x_3).^2.*sin(x_3).^2.*7.25625e-2)+(thp_ref.*sin(x_3).^4.*sin(x_4).^4.*1.209968745785898e-16)./(cos(x_3).^4.*3.628125e-2+sin(x_3).^4.*3.628125e-2+cos(x_3).^2.*sin(x_3).^2.*7.25625e-2)-(thp_ref.*sin(x_3).^4.*sin(x_6).^2.*1.357691522274898e-11)./(cos(x_3).^4.*3.628125e-2+sin(x_3).^4.*3.628125e-2+cos(x_3).^2.*sin(x_3).^2.*7.25625e-2)+(thp_ref.*sin(x_3).^4.*sin(x_5).^4.*1.209968745785898e-16)./(cos(x_3).^4.*3.628125e-2+sin(x_3).^4.*3.628125e-2+cos(x_3).^2.*sin(x_3).^2.*7.25625e-2)+(thp_ref.*sin(x_3).^4.*sin(x_6).^4.*1.209968745785898e-16)./(cos(x_3).^4.*3.628125e-2+sin(x_3).^4.*3.628125e-2+cos(x_3).^2.*sin(x_3).^2.*7.25625e-2)+(thp_ref.*sin(x_3).^3.*sin(x_4).^2.*1.484393539266013e-10)./(cos(x_3).^4.*1.45125e-1+sin(x_3).^4.*1.45125e-1+cos(x_3).^2.*sin(x_3).^2.*2.9025e-1)+(thp_ref.*sin(x_3).^3.*sin(x_5).^2.*1.484393539266013e-10)./(cos(x_3).^4.*1.45125e-1+sin(x_3).^4.*1.45125e-1+cos(x_3).^2.*sin(x_3).^2.*2.9025e-1)+(thp_ref.*sin(x_3).^3.*sin(x_6).^2.*1.484393539266013e-10)./(cos(x_3).^4.*1.45125e-1+sin(x_3).^4.*1.45125e-1+cos(x_3).^2.*sin(x_3).^2.*2.9025e-1)-(thpp_ref.*sin(x_3).^4.*sin(x_4).^2.*3.394228805687245e-12)./(cos(x_3).^4.*3.628125e-2+sin(x_3).^4.*3.628125e-2+cos(x_3).^2.*sin(x_3).^2.*7.25625e-2)-(thpp_ref.*sin(x_3).^4.*sin(x_5).^2.*3.394228805687245e-12)./(cos(x_3).^4.*3.628125e-2+sin(x_3).^4.*3.628125e-2+cos(x_3).^2.*sin(x_3).^2.*7.25625e-2)+(thpp_ref.*sin(x_3).^4.*sin(x_4).^4.*3.024921864464745e-17)./(cos(x_3).^4.*3.628125e-2+sin(x_3).^4.*3.628125e-2+cos(x_3).^2.*sin(x_3).^2.*7.25625e-2)-(thpp_ref.*sin(x_3).^4.*sin(x_6).^2.*3.394228805687245e-12)./(cos(x_3).^4.*3.628125e-2+sin(x_3).^4.*3.628125e-2+cos(x_3).^2.*sin(x_3).^2.*7.25625e-2)+(thpp_ref.*sin(x_3).^4.*sin(x_5).^4.*3.024921864464745e-17)./(cos(x_3).^4.*3.628125e-2+sin(x_3).^4.*3.628125e-2+cos(x_3).^2.*sin(x_3).^2.*7.25625e-2)+(thpp_ref.*sin(x_3).^4.*sin(x_6).^4.*3.024921864464745e-17)./(cos(x_3).^4.*3.628125e-2+sin(x_3).^4.*3.628125e-2+cos(x_3).^2.*sin(x_3).^2.*7.25625e-2)+(thpp_ref.*sin(x_3).^3.*sin(x_4).^2.*3.710983848165032e-11)./(cos(x_3).^4.*1.45125e-1+sin(x_3).^4.*1.45125e-1+cos(x_3).^2.*sin(x_3).^2.*2.9025e-1)+(thpp_ref.*sin(x_3).^3.*sin(x_5).^2.*3.710983848165032e-11)./(cos(x_3).^4.*1.45125e-1+sin(x_3).^4.*1.45125e-1+cos(x_3).^2.*sin(x_3).^2.*2.9025e-1)+(thpp_ref.*sin(x_3).^3.*sin(x_6).^2.*3.710983848165032e-11)./(cos(x_3).^4.*1.45125e-1+sin(x_3).^4.*1.45125e-1+cos(x_3).^2.*sin(x_3).^2.*2.9025e-1)+(x_3.*sin(x_3).^4.*sin(x_4).^2.*1.357691522274898e-11)./(cos(x_3).^4.*3.628125e-2+sin(x_3).^4.*3.628125e-2+cos(x_3).^2.*sin(x_3).^2.*7.25625e-2)+(x_3.*sin(x_3).^4.*sin(x_5).^2.*1.357691522274898e-11)./(cos(x_3).^4.*3.628125e-2+sin(x_3).^4.*3.628125e-2+cos(x_3).^2.*sin(x_3).^2.*7.25625e-2)-(x_3.*sin(x_3).^4.*sin(x_4).^4.*1.209968745785898e-16)./(cos(x_3).^4.*3.628125e-2+sin(x_3).^4.*3.628125e-2+cos(x_3).^2.*sin(x_3).^2.*7.25625e-2)+(x_3.*sin(x_3).^4.*sin(x_6).^2.*1.357691522274898e-11)./(cos(x_3).^4.*3.628125e-2+sin(x_3).^4.*3.628125e-2+cos(x_3).^2.*sin(x_3).^2.*7.25625e-2)+(x_1.*sin(x_3).^3.*sin(x_4).^2.*2.027719283850867e-10)./(cos(x_3).^4.*1.45125e-1+sin(x_3).^4.*1.45125e-1+cos(x_3).^2.*sin(x_3).^2.*2.9025e-1)-(x_3.*sin(x_3).^4.*sin(x_5).^4.*1.209968745785898e-16)./(cos(x_3).^4.*3.628125e-2+sin(x_3).^4.*3.628125e-2+cos(x_3).^2.*sin(x_3).^2.*7.25625e-2)+(x_1.*sin(x_3).^3.*sin(x_5).^2.*2.027719283850867e-10)./(cos(x_3).^4.*1.45125e-1+sin(x_3).^4.*1.45125e-1+cos(x_3).^2.*sin(x_3).^2.*2.9025e-1)+(x_2.*sin(x_3).^3.*sin(x_4).^2.*3.51211282311688e-10)./(cos(x_3).^4.*1.45125e-1+sin(x_3).^4.*1.45125e-1+cos(x_3).^2.*sin(x_3).^2.*2.9025e-1)-(x_3.*sin(x_3).^4.*sin(x_6).^4.*1.209968745785898e-16)./(cos(x_3).^4.*3.628125e-2+sin(x_3).^4.*3.628125e-2+cos(x_3).^2.*sin(x_3).^2.*7.25625e-2)+(x_1.*sin(x_3).^3.*sin(x_6).^2.*2.027719283850867e-10)./(cos(x_3).^4.*1.45125e-1+sin(x_3).^4.*1.45125e-1+cos(x_3).^2.*sin(x_3).^2.*2.9025e-1)+(x_2.*sin(x_3).^3.*sin(x_5).^2.*3.51211282311688e-10)./(cos(x_3).^4.*1.45125e-1+sin(x_3).^4.*1.45125e-1+cos(x_3).^2.*sin(x_3).^2.*2.9025e-1)-(x_3.*sin(x_3).^3.*sin(x_4).^2.*1.484393539266013e-10)./(cos(x_3).^4.*1.45125e-1+sin(x_3).^4.*1.45125e-1+cos(x_3).^2.*sin(x_3).^2.*2.9025e-1)+(x_2.*sin(x_3).^3.*sin(x_6).^2.*3.51211282311688e-10)./(cos(x_3).^4.*1.45125e-1+sin(x_3).^4.*1.45125e-1+cos(x_3).^2.*sin(x_3).^2.*2.9025e-1)-(x_3.*sin(x_3).^3.*sin(x_5).^2.*1.484393539266013e-10)./(cos(x_3).^4.*1.45125e-1+sin(x_3).^4.*1.45125e-1+cos(x_3).^2.*sin(x_3).^2.*2.9025e-1)+(x_9.*sin(x_3).^4.*sin(x_4).^2.*1.357691522274898e-11)./(cos(x_3).^4.*3.628125e-2+sin(x_3).^4.*3.628125e-2+cos(x_3).^2.*sin(x_3).^2.*7.25625e-2)-(x_3.*sin(x_3).^3.*sin(x_6).^2.*1.484393539266013e-10)./(cos(x_3).^4.*1.45125e-1+sin(x_3).^4.*1.45125e-1+cos(x_3).^2.*sin(x_3).^2.*2.9025e-1)+(x_9.*sin(x_3).^4.*sin(x_5).^2.*1.357691522274898e-11)./(cos(x_3).^4.*3.628125e-2+sin(x_3).^4.*3.628125e-2+cos(x_3).^2.*sin(x_3).^2.*7.25625e-2)-(x_9.*sin(x_3).^4.*sin(x_4).^4.*1.209968745785898e-16)./(cos(x_3).^4.*3.628125e-2+sin(x_3).^4.*3.628125e-2+cos(x_3).^2.*sin(x_3).^2.*7.25625e-2)+(x_9.*sin(x_3).^4.*sin(x_6).^2.*1.357691522274898e-11)./(cos(x_3).^4.*3.628125e-2+sin(x_3).^4.*3.628125e-2+cos(x_3).^2.*sin(x_3).^2.*7.25625e-2)+(x_7.*sin(x_3).^3.*sin(x_4).^2.*2.027719283850867e-10)./(cos(x_3).^4.*1.45125e-1+sin(x_3).^4.*1.45125e-1+cos(x_3).^2.*sin(x_3).^2.*2.9025e-1)-(x_9.*sin(x_3).^4.*sin(x_5).^4.*1.209968745785898e-16)./(cos(x_3).^4.*3.628125e-2+sin(x_3).^4.*3.628125e-2+cos(x_3).^2.*sin(x_3).^2.*7.25625e-2)+(x_7.*sin(x_3).^3.*sin(x_5).^2.*2.027719283850867e-10)./(cos(x_3).^4.*1.45125e-1+sin(x_3).^4.*1.45125e-1+cos(x_3).^2.*sin(x_3).^2.*2.9025e-1)+(x_8.*sin(x_3).^3.*sin(x_4).^2.*3.51211282311688e-10)./(cos(x_3).^4.*1.45125e-1+sin(x_3).^4.*1.45125e-1+cos(x_3).^2.*sin(x_3).^2.*2.9025e-1)-(x_9.*sin(x_3).^4.*sin(x_6).^4.*1.209968745785898e-16)./(cos(x_3).^4.*3.628125e-2+sin(x_3).^4.*3.628125e-2+cos(x_3).^2.*sin(x_3).^2.*7.25625e-2)+(x_7.*sin(x_3).^3.*sin(x_6).^2.*2.027719283850867e-10)./(cos(x_3).^4.*1.45125e-1+sin(x_3).^4.*1.45125e-1+cos(x_3).^2.*sin(x_3).^2.*2.9025e-1)+(x_8.*sin(x_3).^3.*sin(x_5).^2.*3.51211282311688e-10)./(cos(x_3).^4.*1.45125e-1+sin(x_3).^4.*1.45125e-1+cos(x_3).^2.*sin(x_3).^2.*2.9025e-1)-(x_9.*sin(x_3).^3.*sin(x_4).^2.*1.484393539266013e-10)./(cos(x_3).^4.*1.45125e-1+sin(x_3).^4.*1.45125e-1+cos(x_3).^2.*sin(x_3).^2.*2.9025e-1)+(x_8.*sin(x_3).^3.*sin(x_6).^2.*3.51211282311688e-10)./(cos(x_3).^4.*1.45125e-1+sin(x_3).^4.*1.45125e-1+cos(x_3).^2.*sin(x_3).^2.*2.9025e-1)-(x_9.*sin(x_3).^3.*sin(x_5).^2.*1.484393539266013e-10)./(cos(x_3).^4.*1.45125e-1+sin(x_3).^4.*1.45125e-1+cos(x_3).^2.*sin(x_3).^2.*2.9025e-1)-(x_9.*sin(x_3).^3.*sin(x_6).^2.*1.484393539266013e-10)./(cos(x_3).^4.*1.45125e-1+sin(x_3).^4.*1.45125e-1+cos(x_3).^2.*sin(x_3).^2.*2.9025e-1)-(x_ref.*sin(x_3).^3.*sin(x_4).^2.*2.027719283850867e-10)./(cos(x_3).^4.*1.45125e-1+sin(x_3).^4.*1.45125e-1+cos(x_3).^2.*sin(x_3).^2.*2.9025e-1)-(x_ref.*sin(x_3).^3.*sin(x_5).^2.*2.027719283850867e-10)./(cos(x_3).^4.*1.45125e-1+sin(x_3).^4.*1.45125e-1+cos(x_3).^2.*sin(x_3).^2.*2.9025e-1)-(x_ref.*sin(x_3).^3.*sin(x_6).^2.*2.027719283850867e-10)./(cos(x_3).^4.*1.45125e-1+sin(x_3).^4.*1.45125e-1+cos(x_3).^2.*sin(x_3).^2.*2.9025e-1)-(xp_ref.*sin(x_3).^3.*sin(x_4).^2.*2.027719283850867e-10)./(cos(x_3).^4.*1.45125e-1+sin(x_3).^4.*1.45125e-1+cos(x_3).^2.*sin(x_3).^2.*2.9025e-1)-(xp_ref.*sin(x_3).^3.*sin(x_5).^2.*2.027719283850867e-10)./(cos(x_3).^4.*1.45125e-1+sin(x_3).^4.*1.45125e-1+cos(x_3).^2.*sin(x_3).^2.*2.9025e-1)-(xp_ref.*sin(x_3).^3.*sin(x_6).^2.*2.027719283850867e-10)./(cos(x_3).^4.*1.45125e-1+sin(x_3).^4.*1.45125e-1+cos(x_3).^2.*sin(x_3).^2.*2.9025e-1)-(xpp_ref.*sin(x_3).^3.*sin(x_4).^2.*5.069298209627167e-11)./(cos(x_3).^4.*1.45125e-1+sin(x_3).^4.*1.45125e-1+cos(x_3).^2.*sin(x_3).^2.*2.9025e-1)-(xpp_ref.*sin(x_3).^3.*sin(x_5).^2.*5.069298209627167e-11)./(cos(x_3).^4.*1.45125e-1+sin(x_3).^4.*1.45125e-1+cos(x_3).^2.*sin(x_3).^2.*2.9025e-1)-(xpp_ref.*sin(x_3).^3.*sin(x_6).^2.*5.069298209627167e-11)./(cos(x_3).^4.*1.45125e-1+sin(x_3).^4.*1.45125e-1+cos(x_3).^2.*sin(x_3).^2.*2.9025e-1)-(y_ref.*sin(x_3).^3.*sin(x_4).^2.*3.51211282311688e-10)./(cos(x_3).^4.*1.45125e-1+sin(x_3).^4.*1.45125e-1+cos(x_3).^2.*sin(x_3).^2.*2.9025e-1)-(y_ref.*sin(x_3).^3.*sin(x_5).^2.*3.51211282311688e-10)./(cos(x_3).^4.*1.45125e-1+sin(x_3).^4.*1.45125e-1+cos(x_3).^2.*sin(x_3).^2.*2.9025e-1)-(y_ref.*sin(x_3).^3.*sin(x_6).^2.*3.51211282311688e-10)./(cos(x_3).^4.*1.45125e-1+sin(x_3).^4.*1.45125e-1+cos(x_3).^2.*sin(x_3).^2.*2.9025e-1)-(yp_ref.*sin(x_3).^3.*sin(x_4).^2.*3.51211282311688e-10)./(cos(x_3).^4.*1.45125e-1+sin(x_3).^4.*1.45125e-1+cos(x_3).^2.*sin(x_3).^2.*2.9025e-1)-(yp_ref.*sin(x_3).^3.*sin(x_5).^2.*3.51211282311688e-10)./(cos(x_3).^4.*1.45125e-1+sin(x_3).^4.*1.45125e-1+cos(x_3).^2.*sin(x_3).^2.*2.9025e-1)-(yp_ref.*sin(x_3).^3.*sin(x_6).^2.*3.51211282311688e-10)./(cos(x_3).^4.*1.45125e-1+sin(x_3).^4.*1.45125e-1+cos(x_3).^2.*sin(x_3).^2.*2.9025e-1)-(ypp_ref.*sin(x_3).^3.*sin(x_4).^2.*8.780282057792199e-11)./(cos(x_3).^4.*1.45125e-1+sin(x_3).^4.*1.45125e-1+cos(x_3).^2.*sin(x_3).^2.*2.9025e-1)-(ypp_ref.*sin(x_3).^3.*sin(x_5).^2.*8.780282057792199e-11)./(cos(x_3).^4.*1.45125e-1+sin(x_3).^4.*1.45125e-1+cos(x_3).^2.*sin(x_3).^2.*2.9025e-1)-(ypp_ref.*sin(x_3).^3.*sin(x_6).^2.*8.780282057792199e-11)./(cos(x_3).^4.*1.45125e-1+sin(x_3).^4.*1.45125e-1+cos(x_3).^2.*sin(x_3).^2.*2.9025e-1)+(x_9.^2.*cos(x_3).^2.*sin(x_3).^2.*1.196429974252612e-51)./(cos(x_3).^4.*3.79080679921875e-6+sin(x_3).^4.*3.79080679921875e-6+cos(x_3).^4.*cos(x_4).^2.*6.757062187003037e-11+cos(x_3).^4.*cos(x_5).^2.*6.757062187003037e-11+cos(x_3).^4.*cos(x_6).^2.*6.757062187003037e-11+cos(x_3).^2.*sin(x_3).^2.*7.5816135984375e-6+cos(x_4).^2.*sin(x_3).^4.*6.757062187003037e-11+cos(x_5).^2.*sin(x_3).^4.*6.757062187003037e-11+cos(x_6).^2.*sin(x_3).^4.*6.757062187003037e-11+cos(x_3).^2.*cos(x_4).^2.*sin(x_3).^2.*1.351412437400607e-10+cos(x_3).^2.*cos(x_5).^2.*sin(x_3).^2.*1.351412437400607e-10+cos(x_3).^2.*cos(x_6).^2.*sin(x_3).^2.*1.351412437400607e-10)-(x_9.^2.*cos(x_3).^4.*sin(x_4).^2.*2.132506319169571e-56)./(cos(x_3).^4.*3.79080679921875e-6+sin(x_3).^4.*3.79080679921875e-6+cos(x_3).^4.*cos(x_4).^2.*6.757062187003037e-11+cos(x_3).^4.*cos(x_5).^2.*6.757062187003037e-11+cos(x_3).^4.*cos(x_6).^2.*6.757062187003037e-11+cos(x_3).^2.*sin(x_3).^2.*7.5816135984375e-6+cos(x_4).^2.*sin(x_3).^4.*6.757062187003037e-11+cos(x_5).^2.*sin(x_3).^4.*6.757062187003037e-11+cos(x_6).^2.*sin(x_3).^4.*6.757062187003037e-11+cos(x_3).^2.*cos(x_4).^2.*sin(x_3).^2.*1.351412437400607e-10+cos(x_3).^2.*cos(x_5).^2.*sin(x_3).^2.*1.351412437400607e-10+cos(x_3).^2.*cos(x_6).^2.*sin(x_3).^2.*1.351412437400607e-10)-(x_9.^2.*cos(x_3).^4.*sin(x_5).^2.*2.132506319169571e-56)./(cos(x_3).^4.*3.79080679921875e-6+sin(x_3).^4.*3.79080679921875e-6+cos(x_3).^4.*cos(x_4).^2.*6.757062187003037e-11+cos(x_3).^4.*cos(x_5).^2.*6.757062187003037e-11+cos(x_3).^4.*cos(x_6).^2.*6.757062187003037e-11+cos(x_3).^2.*sin(x_3).^2.*7.5816135984375e-6+cos(x_4).^2.*sin(x_3).^4.*6.757062187003037e-11+cos(x_5).^2.*sin(x_3).^4.*6.757062187003037e-11+cos(x_6).^2.*sin(x_3).^4.*6.757062187003037e-11+cos(x_3).^2.*cos(x_4).^2.*sin(x_3).^2.*1.351412437400607e-10+cos(x_3).^2.*cos(x_5).^2.*sin(x_3).^2.*1.351412437400607e-10+cos(x_3).^2.*cos(x_6).^2.*sin(x_3).^2.*1.351412437400607e-10)+(x_9.^2.*cos(x_3).^4.*sin(x_4).^4.*1.900480303554306e-61)./(cos(x_3).^4.*3.79080679921875e-6+sin(x_3).^4.*3.79080679921875e-6+cos(x_3).^4.*cos(x_4).^2.*6.757062187003037e-11+cos(x_3).^4.*cos(x_5).^2.*6.757062187003037e-11+cos(x_3).^4.*cos(x_6).^2.*6.757062187003037e-11+cos(x_3).^2.*sin(x_3).^2.*7.5816135984375e-6+cos(x_4).^2.*sin(x_3).^4.*6.757062187003037e-11+cos(x_5).^2.*sin(x_3).^4.*6.757062187003037e-11+cos(x_6).^2.*sin(x_3).^4.*6.757062187003037e-11+cos(x_3).^2.*cos(x_4).^2.*sin(x_3).^2.*1.351412437400607e-10+cos(x_3).^2.*cos(x_5).^2.*sin(x_3).^2.*1.351412437400607e-10+cos(x_3).^2.*cos(x_6).^2.*sin(x_3).^2.*1.351412437400607e-10)-(x_9.^2.*cos(x_3).^4.*sin(x_6).^2.*2.132506319169571e-56)./(cos(x_3).^4.*3.79080679921875e-6+sin(x_3).^4.*3.79080679921875e-6+cos(x_3).^4.*cos(x_4).^2.*6.757062187003037e-11+cos(x_3).^4.*cos(x_5).^2.*6.757062187003037e-11+cos(x_3).^4.*cos(x_6).^2.*6.757062187003037e-11+cos(x_3).^2.*sin(x_3).^2.*7.5816135984375e-6+cos(x_4).^2.*sin(x_3).^4.*6.757062187003037e-11+cos(x_5).^2.*sin(x_3).^4.*6.757062187003037e-11+cos(x_6).^2.*sin(x_3).^4.*6.757062187003037e-11+cos(x_3).^2.*cos(x_4).^2.*sin(x_3).^2.*1.351412437400607e-10+cos(x_3).^2.*cos(x_5).^2.*sin(x_3).^2.*1.351412437400607e-10+cos(x_3).^2.*cos(x_6).^2.*sin(x_3).^2.*1.351412437400607e-10)+(x_9.^2.*cos(x_3).^4.*sin(x_5).^4.*1.900480303554306e-61)./(cos(x_3).^4.*3.79080679921875e-6+sin(x_3).^4.*3.79080679921875e-6+cos(x_3).^4.*cos(x_4).^2.*6.757062187003037e-11+cos(x_3).^4.*cos(x_5).^2.*6.757062187003037e-11+cos(x_3).^4.*cos(x_6).^2.*6.757062187003037e-11+cos(x_3).^2.*sin(x_3).^2.*7.5816135984375e-6+cos(x_4).^2.*sin(x_3).^4.*6.757062187003037e-11+cos(x_5).^2.*sin(x_3).^4.*6.757062187003037e-11+cos(x_6).^2.*sin(x_3).^4.*6.757062187003037e-11+cos(x_3).^2.*cos(x_4).^2.*sin(x_3).^2.*1.351412437400607e-10+cos(x_3).^2.*cos(x_5).^2.*sin(x_3).^2.*1.351412437400607e-10+cos(x_3).^2.*cos(x_6).^2.*sin(x_3).^2.*1.351412437400607e-10)+(x_9.^2.*cos(x_3).^4.*sin(x_6).^4.*1.900480303554306e-61)./(cos(x_3).^4.*3.79080679921875e-6+sin(x_3).^4.*3.79080679921875e-6+cos(x_3).^4.*cos(x_4).^2.*6.757062187003037e-11+cos(x_3).^4.*cos(x_5).^2.*6.757062187003037e-11+cos(x_3).^4.*cos(x_6).^2.*6.757062187003037e-11+cos(x_3).^2.*sin(x_3).^2.*7.5816135984375e-6+cos(x_4).^2.*sin(x_3).^4.*6.757062187003037e-11+cos(x_5).^2.*sin(x_3).^4.*6.757062187003037e-11+cos(x_6).^2.*sin(x_3).^4.*6.757062187003037e-11+cos(x_3).^2.*cos(x_4).^2.*sin(x_3).^2.*1.351412437400607e-10+cos(x_3).^2.*cos(x_5).^2.*sin(x_3).^2.*1.351412437400607e-10+cos(x_3).^2.*cos(x_6).^2.*sin(x_3).^2.*1.351412437400607e-10)+(x_9.^2.*cos(x_3).^3.*sin(x_4).^2.*8.701333683996604e-55)./(cos(x_3).^4.*1.5163227196875e-5+sin(x_3).^4.*1.5163227196875e-5+cos(x_3).^4.*cos(x_4).^2.*2.702824874801215e-10+cos(x_3).^4.*cos(x_5).^2.*2.702824874801215e-10+cos(x_3).^4.*cos(x_6).^2.*2.702824874801215e-10+cos(x_3).^2.*sin(x_3).^2.*3.032645439375e-5+cos(x_4).^2.*sin(x_3).^4.*2.702824874801215e-10+cos(x_5).^2.*sin(x_3).^4.*2.702824874801215e-10+cos(x_6).^2.*sin(x_3).^4.*2.702824874801215e-10+cos(x_3).^2.*cos(x_4).^2.*sin(x_3).^2.*5.40564974960243e-10+cos(x_3).^2.*cos(x_5).^2.*sin(x_3).^2.*5.40564974960243e-10+cos(x_3).^2.*cos(x_6).^2.*sin(x_3).^2.*5.40564974960243e-10)+(x_9.^2.*cos(x_3).^3.*sin(x_5).^2.*8.701333683996604e-55)./(cos(x_3).^4.*1.5163227196875e-5+sin(x_3).^4.*1.5163227196875e-5+cos(x_3).^4.*cos(x_4).^2.*2.702824874801215e-10+cos(x_3).^4.*cos(x_5).^2.*2.702824874801215e-10+cos(x_3).^4.*cos(x_6).^2.*2.702824874801215e-10+cos(x_3).^2.*sin(x_3).^2.*3.032645439375e-5+cos(x_4).^2.*sin(x_3).^4.*2.702824874801215e-10+cos(x_5).^2.*sin(x_3).^4.*2.702824874801215e-10+cos(x_6).^2.*sin(x_3).^4.*2.702824874801215e-10+cos(x_3).^2.*cos(x_4).^2.*sin(x_3).^2.*5.40564974960243e-10+cos(x_3).^2.*cos(x_5).^2.*sin(x_3).^2.*5.40564974960243e-10+cos(x_3).^2.*cos(x_6).^2.*sin(x_3).^2.*5.40564974960243e-10)+(x_9.^2.*cos(x_3).^3.*sin(x_6).^2.*8.701333683996604e-55)./(cos(x_3).^4.*1.5163227196875e-5+sin(x_3).^4.*1.5163227196875e-5+cos(x_3).^4.*cos(x_4).^2.*2.702824874801215e-10+cos(x_3).^4.*cos(x_5).^2.*2.702824874801215e-10+cos(x_3).^4.*cos(x_6).^2.*2.702824874801215e-10+cos(x_3).^2.*sin(x_3).^2.*3.032645439375e-5+cos(x_4).^2.*sin(x_3).^4.*2.702824874801215e-10+cos(x_5).^2.*sin(x_3).^4.*2.702824874801215e-10+cos(x_6).^2.*sin(x_3).^4.*2.702824874801215e-10+cos(x_3).^2.*cos(x_4).^2.*sin(x_3).^2.*5.40564974960243e-10+cos(x_3).^2.*cos(x_5).^2.*sin(x_3).^2.*5.40564974960243e-10+cos(x_3).^2.*cos(x_6).^2.*sin(x_3).^2.*5.40564974960243e-10)-(x_1.*cos(x_3).*sin(x_3).*1.856779265037707e-3)./(cos(x_3).^4.*5.805e-1+sin(x_3).^4.*5.805e-1+cos(x_3).^2.*sin(x_3).^2.*1.161)-(x_2.*cos(x_3).*sin(x_3).*1.856779265037707e-3)./(cos(x_3).^4.*5.805e-1+sin(x_3).^4.*5.805e-1+cos(x_3).^2.*sin(x_3).^2.*1.161)-(x_7.*cos(x_3).*sin(x_3).*1.856779265037707e-3)./(cos(x_3).^4.*5.805e-1+sin(x_3).^4.*5.805e-1+cos(x_3).^2.*sin(x_3).^2.*1.161)-(x_8.*cos(x_3).*sin(x_3).*1.856779265037707e-3)./(cos(x_3).^4.*5.805e-1+sin(x_3).^4.*5.805e-1+cos(x_3).^2.*sin(x_3).^2.*1.161)+(x_ref.*cos(x_3).*sin(x_3).*1.856779265037707e-3)./(cos(x_3).^4.*5.805e-1+sin(x_3).^4.*5.805e-1+cos(x_3).^2.*sin(x_3).^2.*1.161)+(xp_ref.*cos(x_3).*sin(x_3).*1.856779265037707e-3)./(cos(x_3).^4.*5.805e-1+sin(x_3).^4.*5.805e-1+cos(x_3).^2.*sin(x_3).^2.*1.161)+(xpp_ref.*cos(x_3).*sin(x_3).*4.641948162594268e-4)./(cos(x_3).^4.*5.805e-1+sin(x_3).^4.*5.805e-1+cos(x_3).^2.*sin(x_3).^2.*1.161)-(x_9.^2.*sin(x_3).^4.*sin(x_4).^2.*2.132506319169571e-56)./(cos(x_3).^4.*3.79080679921875e-6+sin(x_3).^4.*3.79080679921875e-6+cos(x_3).^4.*cos(x_4).^2.*6.757062187003037e-11+cos(x_3).^4.*cos(x_5).^2.*6.757062187003037e-11+cos(x_3).^4.*cos(x_6).^2.*6.757062187003037e-11+cos(x_3).^2.*sin(x_3).^2.*7.5816135984375e-6+cos(x_4).^2.*sin(x_3).^4.*6.757062187003037e-11+cos(x_5).^2.*sin(x_3).^4.*6.757062187003037e-11+cos(x_6).^2.*sin(x_3).^4.*6.757062187003037e-11+cos(x_3).^2.*cos(x_4).^2.*sin(x_3).^2.*1.351412437400607e-10+cos(x_3).^2.*cos(x_5).^2.*sin(x_3).^2.*1.351412437400607e-10+cos(x_3).^2.*cos(x_6).^2.*sin(x_3).^2.*1.351412437400607e-10)-(x_9.^2.*sin(x_3).^4.*sin(x_5).^2.*2.132506319169571e-56)./(cos(x_3).^4.*3.79080679921875e-6+sin(x_3).^4.*3.79080679921875e-6+cos(x_3).^4.*cos(x_4).^2.*6.757062187003037e-11+cos(x_3).^4.*cos(x_5).^2.*6.757062187003037e-11+cos(x_3).^4.*cos(x_6).^2.*6.757062187003037e-11+cos(x_3).^2.*sin(x_3).^2.*7.5816135984375e-6+cos(x_4).^2.*sin(x_3).^4.*6.757062187003037e-11+cos(x_5).^2.*sin(x_3).^4.*6.757062187003037e-11+cos(x_6).^2.*sin(x_3).^4.*6.757062187003037e-11+cos(x_3).^2.*cos(x_4).^2.*sin(x_3).^2.*1.351412437400607e-10+cos(x_3).^2.*cos(x_5).^2.*sin(x_3).^2.*1.351412437400607e-10+cos(x_3).^2.*cos(x_6).^2.*sin(x_3).^2.*1.351412437400607e-10)+(x_9.^2.*sin(x_3).^4.*sin(x_4).^4.*1.900480303554306e-61)./(cos(x_3).^4.*3.79080679921875e-6+sin(x_3).^4.*3.79080679921875e-6+cos(x_3).^4.*cos(x_4).^2.*6.757062187003037e-11+cos(x_3).^4.*cos(x_5).^2.*6.757062187003037e-11+cos(x_3).^4.*cos(x_6).^2.*6.757062187003037e-11+cos(x_3).^2.*sin(x_3).^2.*7.5816135984375e-6+cos(x_4).^2.*sin(x_3).^4.*6.757062187003037e-11+cos(x_5).^2.*sin(x_3).^4.*6.757062187003037e-11+cos(x_6).^2.*sin(x_3).^4.*6.757062187003037e-11+cos(x_3).^2.*cos(x_4).^2.*sin(x_3).^2.*1.351412437400607e-10+cos(x_3).^2.*cos(x_5).^2.*sin(x_3).^2.*1.351412437400607e-10+cos(x_3).^2.*cos(x_6).^2.*sin(x_3).^2.*1.351412437400607e-10)-(x_9.^2.*sin(x_3).^4.*sin(x_6).^2.*2.132506319169571e-56)./(cos(x_3).^4.*3.79080679921875e-6+sin(x_3).^4.*3.79080679921875e-6+cos(x_3).^4.*cos(x_4).^2.*6.757062187003037e-11+cos(x_3).^4.*cos(x_5).^2.*6.757062187003037e-11+cos(x_3).^4.*cos(x_6).^2.*6.757062187003037e-11+cos(x_3).^2.*sin(x_3).^2.*7.5816135984375e-6+cos(x_4).^2.*sin(x_3).^4.*6.757062187003037e-11+cos(x_5).^2.*sin(x_3).^4.*6.757062187003037e-11+cos(x_6).^2.*sin(x_3).^4.*6.757062187003037e-11+cos(x_3).^2.*cos(x_4).^2.*sin(x_3).^2.*1.351412437400607e-10+cos(x_3).^2.*cos(x_5).^2.*sin(x_3).^2.*1.351412437400607e-10+cos(x_3).^2.*cos(x_6).^2.*sin(x_3).^2.*1.351412437400607e-10)+(x_9.^2.*sin(x_3).^4.*sin(x_5).^4.*1.900480303554306e-61)./(cos(x_3).^4.*3.79080679921875e-6+sin(x_3).^4.*3.79080679921875e-6+cos(x_3).^4.*cos(x_4).^2.*6.757062187003037e-11+cos(x_3).^4.*cos(x_5).^2.*6.757062187003037e-11+cos(x_3).^4.*cos(x_6).^2.*6.757062187003037e-11+cos(x_3).^2.*sin(x_3).^2.*7.5816135984375e-6+cos(x_4).^2.*sin(x_3).^4.*6.757062187003037e-11+cos(x_5).^2.*sin(x_3).^4.*6.757062187003037e-11+cos(x_6).^2.*sin(x_3).^4.*6.757062187003037e-11+cos(x_3).^2.*cos(x_4).^2.*sin(x_3).^2.*1.351412437400607e-10+cos(x_3).^2.*cos(x_5).^2.*sin(x_3).^2.*1.351412437400607e-10+cos(x_3).^2.*cos(x_6).^2.*sin(x_3).^2.*1.351412437400607e-10)+(x_9.^2.*sin(x_3).^4.*sin(x_6).^4.*1.900480303554306e-61)./(cos(x_3).^4.*3.79080679921875e-6+sin(x_3).^4.*3.79080679921875e-6+cos(x_3).^4.*cos(x_4).^2.*6.757062187003037e-11+cos(x_3).^4.*cos(x_5).^2.*6.757062187003037e-11+cos(x_3).^4.*cos(x_6).^2.*6.757062187003037e-11+cos(x_3).^2.*sin(x_3).^2.*7.5816135984375e-6+cos(x_4).^2.*sin(x_3).^4.*6.757062187003037e-11+cos(x_5).^2.*sin(x_3).^4.*6.757062187003037e-11+cos(x_6).^2.*sin(x_3).^4.*6.757062187003037e-11+cos(x_3).^2.*cos(x_4).^2.*sin(x_3).^2.*1.351412437400607e-10+cos(x_3).^2.*cos(x_5).^2.*sin(x_3).^2.*1.351412437400607e-10+cos(x_3).^2.*cos(x_6).^2.*sin(x_3).^2.*1.351412437400607e-10)+(x_9.^2.*sin(x_3).^3.*sin(x_4).^2.*2.331515333700616e-55)./(cos(x_3).^4.*1.5163227196875e-5+sin(x_3).^4.*1.5163227196875e-5+cos(x_3).^4.*cos(x_4).^2.*2.702824874801215e-10+cos(x_3).^4.*cos(x_5).^2.*2.702824874801215e-10+cos(x_3).^4.*cos(x_6).^2.*2.702824874801215e-10+cos(x_3).^2.*sin(x_3).^2.*3.032645439375e-5+cos(x_4).^2.*sin(x_3).^4.*2.702824874801215e-10+cos(x_5).^2.*sin(x_3).^4.*2.702824874801215e-10+cos(x_6).^2.*sin(x_3).^4.*2.702824874801215e-10+cos(x_3).^2.*cos(x_4).^2.*sin(x_3).^2.*5.40564974960243e-10+cos(x_3).^2.*cos(x_5).^2.*sin(x_3).^2.*5.40564974960243e-10+cos(x_3).^2.*cos(x_6).^2.*sin(x_3).^2.*5.40564974960243e-10)+(x_9.^2.*sin(x_3).^3.*sin(x_5).^2.*2.331515333700616e-55)./(cos(x_3).^4.*1.5163227196875e-5+sin(x_3).^4.*1.5163227196875e-5+cos(x_3).^4.*cos(x_4).^2.*2.702824874801215e-10+cos(x_3).^4.*cos(x_5).^2.*2.702824874801215e-10+cos(x_3).^4.*cos(x_6).^2.*2.702824874801215e-10+cos(x_3).^2.*sin(x_3).^2.*3.032645439375e-5+cos(x_4).^2.*sin(x_3).^4.*2.702824874801215e-10+cos(x_5).^2.*sin(x_3).^4.*2.702824874801215e-10+cos(x_6).^2.*sin(x_3).^4.*2.702824874801215e-10+cos(x_3).^2.*cos(x_4).^2.*sin(x_3).^2.*5.40564974960243e-10+cos(x_3).^2.*cos(x_5).^2.*sin(x_3).^2.*5.40564974960243e-10+cos(x_3).^2.*cos(x_6).^2.*sin(x_3).^2.*5.40564974960243e-10)+(x_9.^2.*sin(x_3).^3.*sin(x_6).^2.*2.331515333700616e-55)./(cos(x_3).^4.*1.5163227196875e-5+sin(x_3).^4.*1.5163227196875e-5+cos(x_3).^4.*cos(x_4).^2.*2.702824874801215e-10+cos(x_3).^4.*cos(x_5).^2.*2.702824874801215e-10+cos(x_3).^4.*cos(x_6).^2.*2.702824874801215e-10+cos(x_3).^2.*sin(x_3).^2.*3.032645439375e-5+cos(x_4).^2.*sin(x_3).^4.*2.702824874801215e-10+cos(x_5).^2.*sin(x_3).^4.*2.702824874801215e-10+cos(x_6).^2.*sin(x_3).^4.*2.702824874801215e-10+cos(x_3).^2.*cos(x_4).^2.*sin(x_3).^2.*5.40564974960243e-10+cos(x_3).^2.*cos(x_5).^2.*sin(x_3).^2.*5.40564974960243e-10+cos(x_3).^2.*cos(x_6).^2.*sin(x_3).^2.*5.40564974960243e-10)+(y_ref.*cos(x_3).*sin(x_3).*1.856779265037707e-3)./(cos(x_3).^4.*5.805e-1+sin(x_3).^4.*5.805e-1+cos(x_3).^2.*sin(x_3).^2.*1.161)+(yp_ref.*cos(x_3).*sin(x_3).*1.856779265037707e-3)./(cos(x_3).^4.*5.805e-1+sin(x_3).^4.*5.805e-1+cos(x_3).^2.*sin(x_3).^2.*1.161)+(ypp_ref.*cos(x_3).*sin(x_3).*4.641948162594268e-4)./(cos(x_3).^4.*5.805e-1+sin(x_3).^4.*5.805e-1+cos(x_3).^2.*sin(x_3).^2.*1.161)+(x_9.^2.*sin(x_4.*2.0).*cos(x_3).^4.*2.577480056318101e-16)./(cos(x_3).^4.*3.79080679921875e-6+sin(x_3).^4.*3.79080679921875e-6+cos(x_3).^4.*cos(x_4).^2.*6.757062187003037e-11+cos(x_3).^4.*cos(x_5).^2.*6.757062187003037e-11+cos(x_3).^4.*cos(x_6).^2.*6.757062187003037e-11+cos(x_3).^2.*sin(x_3).^2.*7.5816135984375e-6+cos(x_4).^2.*sin(x_3).^4.*6.757062187003037e-11+cos(x_5).^2.*sin(x_3).^4.*6.757062187003037e-11+cos(x_6).^2.*sin(x_3).^4.*6.757062187003037e-11+cos(x_3).^2.*cos(x_4).^2.*sin(x_3).^2.*1.351412437400607e-10+cos(x_3).^2.*cos(x_5).^2.*sin(x_3).^2.*1.351412437400607e-10+cos(x_3).^2.*cos(x_6).^2.*sin(x_3).^2.*1.351412437400607e-10)+(x_9.^2.*sin(x_5.*2.0).*cos(x_3).^4.*2.577480056318101e-16)./(cos(x_3).^4.*3.79080679921875e-6+sin(x_3).^4.*3.79080679921875e-6+cos(x_3).^4.*cos(x_4).^2.*6.757062187003037e-11+cos(x_3).^4.*cos(x_5).^2.*6.757062187003037e-11+cos(x_3).^4.*cos(x_6).^2.*6.757062187003037e-11+cos(x_3).^2.*sin(x_3).^2.*7.5816135984375e-6+cos(x_4).^2.*sin(x_3).^4.*6.757062187003037e-11+cos(x_5).^2.*sin(x_3).^4.*6.757062187003037e-11+cos(x_6).^2.*sin(x_3).^4.*6.757062187003037e-11+cos(x_3).^2.*cos(x_4).^2.*sin(x_3).^2.*1.351412437400607e-10+cos(x_3).^2.*cos(x_5).^2.*sin(x_3).^2.*1.351412437400607e-10+cos(x_3).^2.*cos(x_6).^2.*sin(x_3).^2.*1.351412437400607e-10)+(x_9.^2.*sin(x_6.*2.0).*cos(x_3).^4.*2.577480056318101e-16)./(cos(x_3).^4.*3.79080679921875e-6+sin(x_3).^4.*3.79080679921875e-6+cos(x_3).^4.*cos(x_4).^2.*6.757062187003037e-11+cos(x_3).^4.*cos(x_5).^2.*6.757062187003037e-11+cos(x_3).^4.*cos(x_6).^2.*6.757062187003037e-11+cos(x_3).^2.*sin(x_3).^2.*7.5816135984375e-6+cos(x_4).^2.*sin(x_3).^4.*6.757062187003037e-11+cos(x_5).^2.*sin(x_3).^4.*6.757062187003037e-11+cos(x_6).^2.*sin(x_3).^4.*6.757062187003037e-11+cos(x_3).^2.*cos(x_4).^2.*sin(x_3).^2.*1.351412437400607e-10+cos(x_3).^2.*cos(x_5).^2.*sin(x_3).^2.*1.351412437400607e-10+cos(x_3).^2.*cos(x_6).^2.*sin(x_3).^2.*1.351412437400607e-10)-(x_9.^2.*sin(x_4.*2.0).*cos(x_3).^3.*2.103394848799675e-14)./(cos(x_3).^4.*1.5163227196875e-5+sin(x_3).^4.*1.5163227196875e-5+cos(x_3).^4.*cos(x_4).^2.*2.702824874801215e-10+cos(x_3).^4.*cos(x_5).^2.*2.702824874801215e-10+cos(x_3).^4.*cos(x_6).^2.*2.702824874801215e-10+cos(x_3).^2.*sin(x_3).^2.*3.032645439375e-5+cos(x_4).^2.*sin(x_3).^4.*2.702824874801215e-10+cos(x_5).^2.*sin(x_3).^4.*2.702824874801215e-10+cos(x_6).^2.*sin(x_3).^4.*2.702824874801215e-10+cos(x_3).^2.*cos(x_4).^2.*sin(x_3).^2.*5.40564974960243e-10+cos(x_3).^2.*cos(x_5).^2.*sin(x_3).^2.*5.40564974960243e-10+cos(x_3).^2.*cos(x_6).^2.*sin(x_3).^2.*5.40564974960243e-10)-(x_9.^2.*sin(x_5.*2.0).*cos(x_3).^3.*2.103394848799675e-14)./(cos(x_3).^4.*1.5163227196875e-5+sin(x_3).^4.*1.5163227196875e-5+cos(x_3).^4.*cos(x_4).^2.*2.702824874801215e-10+cos(x_3).^4.*cos(x_5).^2.*2.702824874801215e-10+cos(x_3).^4.*cos(x_6).^2.*2.702824874801215e-10+cos(x_3).^2.*sin(x_3).^2.*3.032645439375e-5+cos(x_4).^2.*sin(x_3).^4.*2.702824874801215e-10+cos(x_5).^2.*sin(x_3).^4.*2.702824874801215e-10+cos(x_6).^2.*sin(x_3).^4.*2.702824874801215e-10+cos(x_3).^2.*cos(x_4).^2.*sin(x_3).^2.*5.40564974960243e-10+cos(x_3).^2.*cos(x_5).^2.*sin(x_3).^2.*5.40564974960243e-10+cos(x_3).^2.*cos(x_6).^2.*sin(x_3).^2.*5.40564974960243e-10)-(x_9.^2.*sin(x_6.*2.0).*cos(x_3).^3.*2.103394848799675e-14)./(cos(x_3).^4.*1.5163227196875e-5+sin(x_3).^4.*1.5163227196875e-5+cos(x_3).^4.*cos(x_4).^2.*2.702824874801215e-10+cos(x_3).^4.*cos(x_5).^2.*2.702824874801215e-10+cos(x_3).^4.*cos(x_6).^2.*2.702824874801215e-10+cos(x_3).^2.*sin(x_3).^2.*3.032645439375e-5+cos(x_4).^2.*sin(x_3).^4.*2.702824874801215e-10+cos(x_5).^2.*sin(x_3).^4.*2.702824874801215e-10+cos(x_6).^2.*sin(x_3).^4.*2.702824874801215e-10+cos(x_3).^2.*cos(x_4).^2.*sin(x_3).^2.*5.40564974960243e-10+cos(x_3).^2.*cos(x_5).^2.*sin(x_3).^2.*5.40564974960243e-10+cos(x_3).^2.*cos(x_6).^2.*sin(x_3).^2.*5.40564974960243e-10)-(x_9.^2.*sin(x_4.*2.0).*cos(x_3).^2.*2.725959609843749e-8)./(cos(x_3).^2.*6.49519052838329e-1+sin(x_3).^2.*6.49519052838329e-1)-(x_9.^2.*sin(x_5.*2.0).*cos(x_3).^2.*2.725959609843749e-8)./(cos(x_3).^2.*6.49519052838329e-1+sin(x_3).^2.*6.49519052838329e-1)-(x_9.^2.*sin(x_6.*2.0).*cos(x_3).^2.*2.725959609843749e-8)./(cos(x_3).^2.*6.49519052838329e-1+sin(x_3).^2.*6.49519052838329e-1)+(x_9.^2.*sin(x_4.*2.0).*sin(x_3).^4.*2.577480056318101e-16)./(cos(x_3).^4.*3.79080679921875e-6+sin(x_3).^4.*3.79080679921875e-6+cos(x_3).^4.*cos(x_4).^2.*6.757062187003037e-11+cos(x_3).^4.*cos(x_5).^2.*6.757062187003037e-11+cos(x_3).^4.*cos(x_6).^2.*6.757062187003037e-11+cos(x_3).^2.*sin(x_3).^2.*7.5816135984375e-6+cos(x_4).^2.*sin(x_3).^4.*6.757062187003037e-11+cos(x_5).^2.*sin(x_3).^4.*6.757062187003037e-11+cos(x_6).^2.*sin(x_3).^4.*6.757062187003037e-11+cos(x_3).^2.*cos(x_4).^2.*sin(x_3).^2.*1.351412437400607e-10+cos(x_3).^2.*cos(x_5).^2.*sin(x_3).^2.*1.351412437400607e-10+cos(x_3).^2.*cos(x_6).^2.*sin(x_3).^2.*1.351412437400607e-10)+(x_9.^2.*sin(x_5.*2.0).*sin(x_3).^4.*2.577480056318101e-16)./(cos(x_3).^4.*3.79080679921875e-6+sin(x_3).^4.*3.79080679921875e-6+cos(x_3).^4.*cos(x_4).^2.*6.757062187003037e-11+cos(x_3).^4.*cos(x_5).^2.*6.757062187003037e-11+cos(x_3).^4.*cos(x_6).^2.*6.757062187003037e-11+cos(x_3).^2.*sin(x_3).^2.*7.5816135984375e-6+cos(x_4).^2.*sin(x_3).^4.*6.757062187003037e-11+cos(x_5).^2.*sin(x_3).^4.*6.757062187003037e-11+cos(x_6).^2.*sin(x_3).^4.*6.757062187003037e-11+cos(x_3).^2.*cos(x_4).^2.*sin(x_3).^2.*1.351412437400607e-10+cos(x_3).^2.*cos(x_5).^2.*sin(x_3).^2.*1.351412437400607e-10+cos(x_3).^2.*cos(x_6).^2.*sin(x_3).^2.*1.351412437400607e-10)+(x_9.^2.*sin(x_6.*2.0).*sin(x_3).^4.*2.577480056318101e-16)./(cos(x_3).^4.*3.79080679921875e-6+sin(x_3).^4.*3.79080679921875e-6+cos(x_3).^4.*cos(x_4).^2.*6.757062187003037e-11+cos(x_3).^4.*cos(x_5).^2.*6.757062187003037e-11+cos(x_3).^4.*cos(x_6).^2.*6.757062187003037e-11+cos(x_3).^2.*sin(x_3).^2.*7.5816135984375e-6+cos(x_4).^2.*sin(x_3).^4.*6.757062187003037e-11+cos(x_5).^2.*sin(x_3).^4.*6.757062187003037e-11+cos(x_6).^2.*sin(x_3).^4.*6.757062187003037e-11+cos(x_3).^2.*cos(x_4).^2.*sin(x_3).^2.*1.351412437400607e-10+cos(x_3).^2.*cos(x_5).^2.*sin(x_3).^2.*1.351412437400607e-10+cos(x_3).^2.*cos(x_6).^2.*sin(x_3).^2.*1.351412437400607e-10)-(x_9.^2.*sin(x_4.*2.0).*sin(x_3).^3.*5.636029510996564e-15)./(cos(x_3).^4.*1.5163227196875e-5+sin(x_3).^4.*1.5163227196875e-5+cos(x_3).^4.*cos(x_4).^2.*2.702824874801215e-10+cos(x_3).^4.*cos(x_5).^2.*2.702824874801215e-10+cos(x_3).^4.*cos(x_6).^2.*2.702824874801215e-10+cos(x_3).^2.*sin(x_3).^2.*3.032645439375e-5+cos(x_4).^2.*sin(x_3).^4.*2.702824874801215e-10+cos(x_5).^2.*sin(x_3).^4.*2.702824874801215e-10+cos(x_6).^2.*sin(x_3).^4.*2.702824874801215e-10+cos(x_3).^2.*cos(x_4).^2.*sin(x_3).^2.*5.40564974960243e-10+cos(x_3).^2.*cos(x_5).^2.*sin(x_3).^2.*5.40564974960243e-10+cos(x_3).^2.*cos(x_6).^2.*sin(x_3).^2.*5.40564974960243e-10)-(x_9.^2.*sin(x_5.*2.0).*sin(x_3).^3.*5.636029510996564e-15)./(cos(x_3).^4.*1.5163227196875e-5+sin(x_3).^4.*1.5163227196875e-5+cos(x_3).^4.*cos(x_4).^2.*2.702824874801215e-10+cos(x_3).^4.*cos(x_5).^2.*2.702824874801215e-10+cos(x_3).^4.*cos(x_6).^2.*2.702824874801215e-10+cos(x_3).^2.*sin(x_3).^2.*3.032645439375e-5+cos(x_4).^2.*sin(x_3).^4.*2.702824874801215e-10+cos(x_5).^2.*sin(x_3).^4.*2.702824874801215e-10+cos(x_6).^2.*sin(x_3).^4.*2.702824874801215e-10+cos(x_3).^2.*cos(x_4).^2.*sin(x_3).^2.*5.40564974960243e-10+cos(x_3).^2.*cos(x_5).^2.*sin(x_3).^2.*5.40564974960243e-10+cos(x_3).^2.*cos(x_6).^2.*sin(x_3).^2.*5.40564974960243e-10)-(x_9.^2.*sin(x_6.*2.0).*sin(x_3).^3.*5.636029510996564e-15)./(cos(x_3).^4.*1.5163227196875e-5+sin(x_3).^4.*1.5163227196875e-5+cos(x_3).^4.*cos(x_4).^2.*2.702824874801215e-10+cos(x_3).^4.*cos(x_5).^2.*2.702824874801215e-10+cos(x_3).^4.*cos(x_6).^2.*2.702824874801215e-10+cos(x_3).^2.*sin(x_3).^2.*3.032645439375e-5+cos(x_4).^2.*sin(x_3).^4.*2.702824874801215e-10+cos(x_5).^2.*sin(x_3).^4.*2.702824874801215e-10+cos(x_6).^2.*sin(x_3).^4.*2.702824874801215e-10+cos(x_3).^2.*cos(x_4).^2.*sin(x_3).^2.*5.40564974960243e-10+cos(x_3).^2.*cos(x_5).^2.*sin(x_3).^2.*5.40564974960243e-10+cos(x_3).^2.*cos(x_6).^2.*sin(x_3).^2.*5.40564974960243e-10)-(x_9.^2.*sin(x_4.*2.0).*sin(x_3).^2.*2.725959609843749e-8)./(cos(x_3).^2.*6.49519052838329e-1+sin(x_3).^2.*6.49519052838329e-1)-(x_9.^2.*sin(x_5.*2.0).*sin(x_3).^2.*2.725959609843749e-8)./(cos(x_3).^2.*6.49519052838329e-1+sin(x_3).^2.*6.49519052838329e-1)-(x_9.^2.*sin(x_6.*2.0).*sin(x_3).^2.*2.725959609843749e-8)./(cos(x_3).^2.*6.49519052838329e-1+sin(x_3).^2.*6.49519052838329e-1)-(th_ref.*cos(x_3).*sin(x_3).^2.*3.108089821597464e-5)./(cos(x_3).^4.*1.45125e-1+sin(x_3).^4.*1.45125e-1+cos(x_3).^2.*sin(x_3).^2.*2.9025e-1)-(th_ref.*cos(x_3).^2.*sin(x_3).*8.328101577004326e-6)./(cos(x_3).^4.*1.45125e-1+sin(x_3).^4.*1.45125e-1+cos(x_3).^2.*sin(x_3).^2.*2.9025e-1)-(thp_ref.*cos(x_3).*sin(x_3).^2.*3.108089821597464e-5)./(cos(x_3).^4.*1.45125e-1+sin(x_3).^4.*1.45125e-1+cos(x_3).^2.*sin(x_3).^2.*2.9025e-1)-(thp_ref.*cos(x_3).^2.*sin(x_3).*8.328101577004326e-6)./(cos(x_3).^4.*1.45125e-1+sin(x_3).^4.*1.45125e-1+cos(x_3).^2.*sin(x_3).^2.*2.9025e-1)-(thpp_ref.*cos(x_3).*sin(x_3).^2.*7.770224553993659e-6)./(cos(x_3).^4.*1.45125e-1+sin(x_3).^4.*1.45125e-1+cos(x_3).^2.*sin(x_3).^2.*2.9025e-1)-(thpp_ref.*cos(x_3).^2.*sin(x_3).*2.082025394251082e-6)./(cos(x_3).^4.*1.45125e-1+sin(x_3).^4.*1.45125e-1+cos(x_3).^2.*sin(x_3).^2.*2.9025e-1)-(x_1.*cos(x_3).*sin(x_3).^2.*1.970449989648948e-5)./(cos(x_3).^4.*1.45125e-1+sin(x_3).^4.*1.45125e-1+cos(x_3).^2.*sin(x_3).^2.*2.9025e-1)-(x_1.*cos(x_3).^2.*sin(x_3).*1.137639831948516e-5)./(cos(x_3).^4.*1.45125e-1+sin(x_3).^4.*1.45125e-1+cos(x_3).^2.*sin(x_3).^2.*2.9025e-1)+(x_2.*cos(x_3).*sin(x_3).^2.*1.137639831948516e-5)./(cos(x_3).^4.*1.45125e-1+sin(x_3).^4.*1.45125e-1+cos(x_3).^2.*sin(x_3).^2.*2.9025e-1)-(x_2.*cos(x_3).^2.*sin(x_3).*1.970449989648948e-5)./(cos(x_3).^4.*1.45125e-1+sin(x_3).^4.*1.45125e-1+cos(x_3).^2.*sin(x_3).^2.*2.9025e-1)+(x_3.*cos(x_3).*sin(x_3).^2.*3.108089821597464e-5)./(cos(x_3).^4.*1.45125e-1+sin(x_3).^4.*1.45125e-1+cos(x_3).^2.*sin(x_3).^2.*2.9025e-1)+(x_3.*cos(x_3).^2.*sin(x_3).*8.328101577004326e-6)./(cos(x_3).^4.*1.45125e-1+sin(x_3).^4.*1.45125e-1+cos(x_3).^2.*sin(x_3).^2.*2.9025e-1)-(x_7.*cos(x_3).*sin(x_3).^2.*1.970449989648948e-5)./(cos(x_3).^4.*1.45125e-1+sin(x_3).^4.*1.45125e-1+cos(x_3).^2.*sin(x_3).^2.*2.9025e-1)-(x_7.*cos(x_3).^2.*sin(x_3).*1.137639831948516e-5)./(cos(x_3).^4.*1.45125e-1+sin(x_3).^4.*1.45125e-1+cos(x_3).^2.*sin(x_3).^2.*2.9025e-1)+(x_8.*cos(x_3).*sin(x_3).^2.*1.137639831948516e-5)./(cos(x_3).^4.*1.45125e-1+sin(x_3).^4.*1.45125e-1+cos(x_3).^2.*sin(x_3).^2.*2.9025e-1)-(x_8.*cos(x_3).^2.*sin(x_3).*1.970449989648948e-5)./(cos(x_3).^4.*1.45125e-1+sin(x_3).^4.*1.45125e-1+cos(x_3).^2.*sin(x_3).^2.*2.9025e-1)+(x_9.*cos(x_3).*sin(x_3).^2.*3.108089821597464e-5)./(cos(x_3).^4.*1.45125e-1+sin(x_3).^4.*1.45125e-1+cos(x_3).^2.*sin(x_3).^2.*2.9025e-1)+(x_9.*cos(x_3).^2.*sin(x_3).*8.328101577004326e-6)./(cos(x_3).^4.*1.45125e-1+sin(x_3).^4.*1.45125e-1+cos(x_3).^2.*sin(x_3).^2.*2.9025e-1)+(x_ref.*cos(x_3).*sin(x_3).^2.*1.970449989648948e-5)./(cos(x_3).^4.*1.45125e-1+sin(x_3).^4.*1.45125e-1+cos(x_3).^2.*sin(x_3).^2.*2.9025e-1)+(x_ref.*cos(x_3).^2.*sin(x_3).*1.137639831948516e-5)./(cos(x_3).^4.*1.45125e-1+sin(x_3).^4.*1.45125e-1+cos(x_3).^2.*sin(x_3).^2.*2.9025e-1)+(xp_ref.*cos(x_3).*sin(x_3).^2.*1.970449989648948e-5)./(cos(x_3).^4.*1.45125e-1+sin(x_3).^4.*1.45125e-1+cos(x_3).^2.*sin(x_3).^2.*2.9025e-1)+(xp_ref.*cos(x_3).^2.*sin(x_3).*1.137639831948516e-5)./(cos(x_3).^4.*1.45125e-1+sin(x_3).^4.*1.45125e-1+cos(x_3).^2.*sin(x_3).^2.*2.9025e-1)+(xpp_ref.*cos(x_3).*sin(x_3).^2.*4.92612497412237e-6)./(cos(x_3).^4.*1.45125e-1+sin(x_3).^4.*1.45125e-1+cos(x_3).^2.*sin(x_3).^2.*2.9025e-1)+(xpp_ref.*cos(x_3).^2.*sin(x_3).*2.844099579871289e-6)./(cos(x_3).^4.*1.45125e-1+sin(x_3).^4.*1.45125e-1+cos(x_3).^2.*sin(x_3).^2.*2.9025e-1)-(y_ref.*cos(x_3).*sin(x_3).^2.*1.137639831948516e-5)./(cos(x_3).^4.*1.45125e-1+sin(x_3).^4.*1.45125e-1+cos(x_3).^2.*sin(x_3).^2.*2.9025e-1)+(y_ref.*cos(x_3).^2.*sin(x_3).*1.970449989648948e-5)./(cos(x_3).^4.*1.45125e-1+sin(x_3).^4.*1.45125e-1+cos(x_3).^2.*sin(x_3).^2.*2.9025e-1)-(yp_ref.*cos(x_3).*sin(x_3).^2.*1.137639831948516e-5)./(cos(x_3).^4.*1.45125e-1+sin(x_3).^4.*1.45125e-1+cos(x_3).^2.*sin(x_3).^2.*2.9025e-1)+(yp_ref.*cos(x_3).^2.*sin(x_3).*1.970449989648948e-5)./(cos(x_3).^4.*1.45125e-1+sin(x_3).^4.*1.45125e-1+cos(x_3).^2.*sin(x_3).^2.*2.9025e-1)-(ypp_ref.*cos(x_3).*sin(x_3).^2.*2.844099579871289e-6)./(cos(x_3).^4.*1.45125e-1+sin(x_3).^4.*1.45125e-1+cos(x_3).^2.*sin(x_3).^2.*2.9025e-1)+(ypp_ref.*cos(x_3).^2.*sin(x_3).*4.92612497412237e-6)./(cos(x_3).^4.*1.45125e-1+sin(x_3).^4.*1.45125e-1+cos(x_3).^2.*sin(x_3).^2.*2.9025e-1)-(x_9.^2.*cos(x_3).*sin(x_3).^2.*4.881831459032421e-50)./(cos(x_3).^4.*1.5163227196875e-5+sin(x_3).^4.*1.5163227196875e-5+cos(x_3).^4.*cos(x_4).^2.*2.702824874801215e-10+cos(x_3).^4.*cos(x_5).^2.*2.702824874801215e-10+cos(x_3).^4.*cos(x_6).^2.*2.702824874801215e-10+cos(x_3).^2.*sin(x_3).^2.*3.032645439375e-5+cos(x_4).^2.*sin(x_3).^4.*2.702824874801215e-10+cos(x_5).^2.*sin(x_3).^4.*2.702824874801215e-10+cos(x_6).^2.*sin(x_3).^4.*2.702824874801215e-10+cos(x_3).^2.*cos(x_4).^2.*sin(x_3).^2.*5.40564974960243e-10+cos(x_3).^2.*cos(x_5).^2.*sin(x_3).^2.*5.40564974960243e-10+cos(x_3).^2.*cos(x_6).^2.*sin(x_3).^2.*5.40564974960243e-10)-(x_9.^2.*cos(x_3).^2.*sin(x_3).*1.308082797032587e-50)./(cos(x_3).^4.*1.5163227196875e-5+sin(x_3).^4.*1.5163227196875e-5+cos(x_3).^4.*cos(x_4).^2.*2.702824874801215e-10+cos(x_3).^4.*cos(x_5).^2.*2.702824874801215e-10+cos(x_3).^4.*cos(x_6).^2.*2.702824874801215e-10+cos(x_3).^2.*sin(x_3).^2.*3.032645439375e-5+cos(x_4).^2.*sin(x_3).^4.*2.702824874801215e-10+cos(x_5).^2.*sin(x_3).^4.*2.702824874801215e-10+cos(x_6).^2.*sin(x_3).^4.*2.702824874801215e-10+cos(x_3).^2.*cos(x_4).^2.*sin(x_3).^2.*5.40564974960243e-10+cos(x_3).^2.*cos(x_5).^2.*sin(x_3).^2.*5.40564974960243e-10+cos(x_3).^2.*cos(x_6).^2.*sin(x_3).^2.*5.40564974960243e-10)+(th_ref.*cos(x_3).*sin(x_3).^2.*sin(x_4).^2.*5.539832106967747e-10)./(cos(x_3).^4.*1.45125e-1+sin(x_3).^4.*1.45125e-1+cos(x_3).^2.*sin(x_3).^2.*2.9025e-1)+(th_ref.*cos(x_3).^2.*sin(x_3).*sin(x_4).^2.*1.484393539266013e-10)./(cos(x_3).^4.*1.45125e-1+sin(x_3).^4.*1.45125e-1+cos(x_3).^2.*sin(x_3).^2.*2.9025e-1)+(th_ref.*cos(x_3).*sin(x_3).^2.*sin(x_5).^2.*5.539832106967747e-10)./(cos(x_3).^4.*1.45125e-1+sin(x_3).^4.*1.45125e-1+cos(x_3).^2.*sin(x_3).^2.*2.9025e-1)+(th_ref.*cos(x_3).^2.*sin(x_3).*sin(x_5).^2.*1.484393539266013e-10)./(cos(x_3).^4.*1.45125e-1+sin(x_3).^4.*1.45125e-1+cos(x_3).^2.*sin(x_3).^2.*2.9025e-1)+(th_ref.*cos(x_3).*sin(x_3).^2.*sin(x_6).^2.*5.539832106967747e-10)./(cos(x_3).^4.*1.45125e-1+sin(x_3).^4.*1.45125e-1+cos(x_3).^2.*sin(x_3).^2.*2.9025e-1)+(th_ref.*cos(x_3).^2.*sin(x_3).*sin(x_6).^2.*1.484393539266013e-10)./(cos(x_3).^4.*1.45125e-1+sin(x_3).^4.*1.45125e-1+cos(x_3).^2.*sin(x_3).^2.*2.9025e-1)+(thp_ref.*cos(x_3).*sin(x_3).^2.*sin(x_4).^2.*5.539832106967747e-10)./(cos(x_3).^4.*1.45125e-1+sin(x_3).^4.*1.45125e-1+cos(x_3).^2.*sin(x_3).^2.*2.9025e-1)+(thp_ref.*cos(x_3).^2.*sin(x_3).*sin(x_4).^2.*1.484393539266013e-10)./(cos(x_3).^4.*1.45125e-1+sin(x_3).^4.*1.45125e-1+cos(x_3).^2.*sin(x_3).^2.*2.9025e-1)+(thp_ref.*cos(x_3).*sin(x_3).^2.*sin(x_5).^2.*5.539832106967747e-10)./(cos(x_3).^4.*1.45125e-1+sin(x_3).^4.*1.45125e-1+cos(x_3).^2.*sin(x_3).^2.*2.9025e-1)+(thp_ref.*cos(x_3).^2.*sin(x_3).*sin(x_5).^2.*1.484393539266013e-10)./(cos(x_3).^4.*1.45125e-1+sin(x_3).^4.*1.45125e-1+cos(x_3).^2.*sin(x_3).^2.*2.9025e-1)+(thp_ref.*cos(x_3).*sin(x_3).^2.*sin(x_6).^2.*5.539832106967747e-10)./(cos(x_3).^4.*1.45125e-1+sin(x_3).^4.*1.45125e-1+cos(x_3).^2.*sin(x_3).^2.*2.9025e-1)+(thp_ref.*cos(x_3).^2.*sin(x_3).*sin(x_6).^2.*1.484393539266013e-10)./(cos(x_3).^4.*1.45125e-1+sin(x_3).^4.*1.45125e-1+cos(x_3).^2.*sin(x_3).^2.*2.9025e-1)+(thpp_ref.*cos(x_3).*sin(x_3).^2.*sin(x_4).^2.*1.384958026741937e-10)./(cos(x_3).^4.*1.45125e-1+sin(x_3).^4.*1.45125e-1+cos(x_3).^2.*sin(x_3).^2.*2.9025e-1)+(thpp_ref.*cos(x_3).^2.*sin(x_3).*sin(x_4).^2.*3.710983848165032e-11)./(cos(x_3).^4.*1.45125e-1+sin(x_3).^4.*1.45125e-1+cos(x_3).^2.*sin(x_3).^2.*2.9025e-1)+(thpp_ref.*cos(x_3).*sin(x_3).^2.*sin(x_5).^2.*1.384958026741937e-10)./(cos(x_3).^4.*1.45125e-1+sin(x_3).^4.*1.45125e-1+cos(x_3).^2.*sin(x_3).^2.*2.9025e-1)+(thpp_ref.*cos(x_3).^2.*sin(x_3).*sin(x_5).^2.*3.710983848165032e-11)./(cos(x_3).^4.*1.45125e-1+sin(x_3).^4.*1.45125e-1+cos(x_3).^2.*sin(x_3).^2.*2.9025e-1)+(thpp_ref.*cos(x_3).*sin(x_3).^2.*sin(x_6).^2.*1.384958026741937e-10)./(cos(x_3).^4.*1.45125e-1+sin(x_3).^4.*1.45125e-1+cos(x_3).^2.*sin(x_3).^2.*2.9025e-1)+(thpp_ref.*cos(x_3).^2.*sin(x_3).*sin(x_6).^2.*3.710983848165032e-11)./(cos(x_3).^4.*1.45125e-1+sin(x_3).^4.*1.45125e-1+cos(x_3).^2.*sin(x_3).^2.*2.9025e-1)+(x_1.*cos(x_3).*sin(x_3).^2.*sin(x_4).^2.*3.51211282311688e-10)./(cos(x_3).^4.*1.45125e-1+sin(x_3).^4.*1.45125e-1+cos(x_3).^2.*sin(x_3).^2.*2.9025e-1)+(x_1.*cos(x_3).^2.*sin(x_3).*sin(x_4).^2.*2.027719283850867e-10)./(cos(x_3).^4.*1.45125e-1+sin(x_3).^4.*1.45125e-1+cos(x_3).^2.*sin(x_3).^2.*2.9025e-1)+(x_1.*cos(x_3).*sin(x_3).^2.*sin(x_5).^2.*3.51211282311688e-10)./(cos(x_3).^4.*1.45125e-1+sin(x_3).^4.*1.45125e-1+cos(x_3).^2.*sin(x_3).^2.*2.9025e-1)+(x_1.*cos(x_3).^2.*sin(x_3).*sin(x_5).^2.*2.027719283850867e-10)./(cos(x_3).^4.*1.45125e-1+sin(x_3).^4.*1.45125e-1+cos(x_3).^2.*sin(x_3).^2.*2.9025e-1)-(x_2.*cos(x_3).*sin(x_3).^2.*sin(x_4).^2.*2.027719283850867e-10)./(cos(x_3).^4.*1.45125e-1+sin(x_3).^4.*1.45125e-1+cos(x_3).^2.*sin(x_3).^2.*2.9025e-1)+(x_2.*cos(x_3).^2.*sin(x_3).*sin(x_4).^2.*3.51211282311688e-10)./(cos(x_3).^4.*1.45125e-1+sin(x_3).^4.*1.45125e-1+cos(x_3).^2.*sin(x_3).^2.*2.9025e-1)+(x_1.*cos(x_3).*sin(x_3).^2.*sin(x_6).^2.*3.51211282311688e-10)./(cos(x_3).^4.*1.45125e-1+sin(x_3).^4.*1.45125e-1+cos(x_3).^2.*sin(x_3).^2.*2.9025e-1)+(x_1.*cos(x_3).^2.*sin(x_3).*sin(x_6).^2.*2.027719283850867e-10)./(cos(x_3).^4.*1.45125e-1+sin(x_3).^4.*1.45125e-1+cos(x_3).^2.*sin(x_3).^2.*2.9025e-1)-(x_2.*cos(x_3).*sin(x_3).^2.*sin(x_5).^2.*2.027719283850867e-10)./(cos(x_3).^4.*1.45125e-1+sin(x_3).^4.*1.45125e-1+cos(x_3).^2.*sin(x_3).^2.*2.9025e-1)+(x_2.*cos(x_3).^2.*sin(x_3).*sin(x_5).^2.*3.51211282311688e-10)./(cos(x_3).^4.*1.45125e-1+sin(x_3).^4.*1.45125e-1+cos(x_3).^2.*sin(x_3).^2.*2.9025e-1)-(x_3.*cos(x_3).*sin(x_3).^2.*sin(x_4).^2.*5.539832106967747e-10)./(cos(x_3).^4.*1.45125e-1+sin(x_3).^4.*1.45125e-1+cos(x_3).^2.*sin(x_3).^2.*2.9025e-1)-(x_3.*cos(x_3).^2.*sin(x_3).*sin(x_4).^2.*1.484393539266013e-10)./(cos(x_3).^4.*1.45125e-1+sin(x_3).^4.*1.45125e-1+cos(x_3).^2.*sin(x_3).^2.*2.9025e-1)-(x_2.*cos(x_3).*sin(x_3).^2.*sin(x_6).^2.*2.027719283850867e-10)./(cos(x_3).^4.*1.45125e-1+sin(x_3).^4.*1.45125e-1+cos(x_3).^2.*sin(x_3).^2.*2.9025e-1)+(x_2.*cos(x_3).^2.*sin(x_3).*sin(x_6).^2.*3.51211282311688e-10)./(cos(x_3).^4.*1.45125e-1+sin(x_3).^4.*1.45125e-1+cos(x_3).^2.*sin(x_3).^2.*2.9025e-1)-(x_3.*cos(x_3).*sin(x_3).^2.*sin(x_5).^2.*5.539832106967747e-10)./(cos(x_3).^4.*1.45125e-1+sin(x_3).^4.*1.45125e-1+cos(x_3).^2.*sin(x_3).^2.*2.9025e-1)-(x_3.*cos(x_3).^2.*sin(x_3).*sin(x_5).^2.*1.484393539266013e-10)./(cos(x_3).^4.*1.45125e-1+sin(x_3).^4.*1.45125e-1+cos(x_3).^2.*sin(x_3).^2.*2.9025e-1)-(x_3.*cos(x_3).*sin(x_3).^2.*sin(x_6).^2.*5.539832106967747e-10)./(cos(x_3).^4.*1.45125e-1+sin(x_3).^4.*1.45125e-1+cos(x_3).^2.*sin(x_3).^2.*2.9025e-1)-(x_3.*cos(x_3).^2.*sin(x_3).*sin(x_6).^2.*1.484393539266013e-10)./(cos(x_3).^4.*1.45125e-1+sin(x_3).^4.*1.45125e-1+cos(x_3).^2.*sin(x_3).^2.*2.9025e-1)+(x_7.*cos(x_3).*sin(x_3).^2.*sin(x_4).^2.*3.51211282311688e-10)./(cos(x_3).^4.*1.45125e-1+sin(x_3).^4.*1.45125e-1+cos(x_3).^2.*sin(x_3).^2.*2.9025e-1)+(x_7.*cos(x_3).^2.*sin(x_3).*sin(x_4).^2.*2.027719283850867e-10)./(cos(x_3).^4.*1.45125e-1+sin(x_3).^4.*1.45125e-1+cos(x_3).^2.*sin(x_3).^2.*2.9025e-1)+(x_7.*cos(x_3).*sin(x_3).^2.*sin(x_5).^2.*3.51211282311688e-10)./(cos(x_3).^4.*1.45125e-1+sin(x_3).^4.*1.45125e-1+cos(x_3).^2.*sin(x_3).^2.*2.9025e-1)+(x_7.*cos(x_3).^2.*sin(x_3).*sin(x_5).^2.*2.027719283850867e-10)./(cos(x_3).^4.*1.45125e-1+sin(x_3).^4.*1.45125e-1+cos(x_3).^2.*sin(x_3).^2.*2.9025e-1)-(x_8.*cos(x_3).*sin(x_3).^2.*sin(x_4).^2.*2.027719283850867e-10)./(cos(x_3).^4.*1.45125e-1+sin(x_3).^4.*1.45125e-1+cos(x_3).^2.*sin(x_3).^2.*2.9025e-1)+(x_8.*cos(x_3).^2.*sin(x_3).*sin(x_4).^2.*3.51211282311688e-10)./(cos(x_3).^4.*1.45125e-1+sin(x_3).^4.*1.45125e-1+cos(x_3).^2.*sin(x_3).^2.*2.9025e-1)+(x_7.*cos(x_3).*sin(x_3).^2.*sin(x_6).^2.*3.51211282311688e-10)./(cos(x_3).^4.*1.45125e-1+sin(x_3).^4.*1.45125e-1+cos(x_3).^2.*sin(x_3).^2.*2.9025e-1)+(x_7.*cos(x_3).^2.*sin(x_3).*sin(x_6).^2.*2.027719283850867e-10)./(cos(x_3).^4.*1.45125e-1+sin(x_3).^4.*1.45125e-1+cos(x_3).^2.*sin(x_3).^2.*2.9025e-1)-(x_8.*cos(x_3).*sin(x_3).^2.*sin(x_5).^2.*2.027719283850867e-10)./(cos(x_3).^4.*1.45125e-1+sin(x_3).^4.*1.45125e-1+cos(x_3).^2.*sin(x_3).^2.*2.9025e-1)+(x_8.*cos(x_3).^2.*sin(x_3).*sin(x_5).^2.*3.51211282311688e-10)./(cos(x_3).^4.*1.45125e-1+sin(x_3).^4.*1.45125e-1+cos(x_3).^2.*sin(x_3).^2.*2.9025e-1)-(x_9.*cos(x_3).*sin(x_3).^2.*sin(x_4).^2.*5.539832106967747e-10)./(cos(x_3).^4.*1.45125e-1+sin(x_3).^4.*1.45125e-1+cos(x_3).^2.*sin(x_3).^2.*2.9025e-1)-(x_9.*cos(x_3).^2.*sin(x_3).*sin(x_4).^2.*1.484393539266013e-10)./(cos(x_3).^4.*1.45125e-1+sin(x_3).^4.*1.45125e-1+cos(x_3).^2.*sin(x_3).^2.*2.9025e-1)-(x_8.*cos(x_3).*sin(x_3).^2.*sin(x_6).^2.*2.027719283850867e-10)./(cos(x_3).^4.*1.45125e-1+sin(x_3).^4.*1.45125e-1+cos(x_3).^2.*sin(x_3).^2.*2.9025e-1)+(x_8.*cos(x_3).^2.*sin(x_3).*sin(x_6).^2.*3.51211282311688e-10)./(cos(x_3).^4.*1.45125e-1+sin(x_3).^4.*1.45125e-1+cos(x_3).^2.*sin(x_3).^2.*2.9025e-1)-(x_9.*cos(x_3).*sin(x_3).^2.*sin(x_5).^2.*5.539832106967747e-10)./(cos(x_3).^4.*1.45125e-1+sin(x_3).^4.*1.45125e-1+cos(x_3).^2.*sin(x_3).^2.*2.9025e-1)-(x_9.*cos(x_3).^2.*sin(x_3).*sin(x_5).^2.*1.484393539266013e-10)./(cos(x_3).^4.*1.45125e-1+sin(x_3).^4.*1.45125e-1+cos(x_3).^2.*sin(x_3).^2.*2.9025e-1)-(x_9.*cos(x_3).*sin(x_3).^2.*sin(x_6).^2.*5.539832106967747e-10)./(cos(x_3).^4.*1.45125e-1+sin(x_3).^4.*1.45125e-1+cos(x_3).^2.*sin(x_3).^2.*2.9025e-1)-(x_9.*cos(x_3).^2.*sin(x_3).*sin(x_6).^2.*1.484393539266013e-10)./(cos(x_3).^4.*1.45125e-1+sin(x_3).^4.*1.45125e-1+cos(x_3).^2.*sin(x_3).^2.*2.9025e-1)-(x_ref.*cos(x_3).*sin(x_3).^2.*sin(x_4).^2.*3.51211282311688e-10)./(cos(x_3).^4.*1.45125e-1+sin(x_3).^4.*1.45125e-1+cos(x_3).^2.*sin(x_3).^2.*2.9025e-1)-(x_ref.*cos(x_3).^2.*sin(x_3).*sin(x_4).^2.*2.027719283850867e-10)./(cos(x_3).^4.*1.45125e-1+sin(x_3).^4.*1.45125e-1+cos(x_3).^2.*sin(x_3).^2.*2.9025e-1)-(x_ref.*cos(x_3).*sin(x_3).^2.*sin(x_5).^2.*3.51211282311688e-10)./(cos(x_3).^4.*1.45125e-1+sin(x_3).^4.*1.45125e-1+cos(x_3).^2.*sin(x_3).^2.*2.9025e-1)-(x_ref.*cos(x_3).^2.*sin(x_3).*sin(x_5).^2.*2.027719283850867e-10)./(cos(x_3).^4.*1.45125e-1+sin(x_3).^4.*1.45125e-1+cos(x_3).^2.*sin(x_3).^2.*2.9025e-1)-(x_ref.*cos(x_3).*sin(x_3).^2.*sin(x_6).^2.*3.51211282311688e-10)./(cos(x_3).^4.*1.45125e-1+sin(x_3).^4.*1.45125e-1+cos(x_3).^2.*sin(x_3).^2.*2.9025e-1)-(x_ref.*cos(x_3).^2.*sin(x_3).*sin(x_6).^2.*2.027719283850867e-10)./(cos(x_3).^4.*1.45125e-1+sin(x_3).^4.*1.45125e-1+cos(x_3).^2.*sin(x_3).^2.*2.9025e-1)-(xp_ref.*cos(x_3).*sin(x_3).^2.*sin(x_4).^2.*3.51211282311688e-10)./(cos(x_3).^4.*1.45125e-1+sin(x_3).^4.*1.45125e-1+cos(x_3).^2.*sin(x_3).^2.*2.9025e-1)-(xp_ref.*cos(x_3).^2.*sin(x_3).*sin(x_4).^2.*2.027719283850867e-10)./(cos(x_3).^4.*1.45125e-1+sin(x_3).^4.*1.45125e-1+cos(x_3).^2.*sin(x_3).^2.*2.9025e-1)-(xp_ref.*cos(x_3).*sin(x_3).^2.*sin(x_5).^2.*3.51211282311688e-10)./(cos(x_3).^4.*1.45125e-1+sin(x_3).^4.*1.45125e-1+cos(x_3).^2.*sin(x_3).^2.*2.9025e-1)-(xp_ref.*cos(x_3).^2.*sin(x_3).*sin(x_5).^2.*2.027719283850867e-10)./(cos(x_3).^4.*1.45125e-1+sin(x_3).^4.*1.45125e-1+cos(x_3).^2.*sin(x_3).^2.*2.9025e-1)-(xp_ref.*cos(x_3).*sin(x_3).^2.*sin(x_6).^2.*3.51211282311688e-10)./(cos(x_3).^4.*1.45125e-1+sin(x_3).^4.*1.45125e-1+cos(x_3).^2.*sin(x_3).^2.*2.9025e-1)-(xp_ref.*cos(x_3).^2.*sin(x_3).*sin(x_6).^2.*2.027719283850867e-10)./(cos(x_3).^4.*1.45125e-1+sin(x_3).^4.*1.45125e-1+cos(x_3).^2.*sin(x_3).^2.*2.9025e-1)-(xpp_ref.*cos(x_3).*sin(x_3).^2.*sin(x_4).^2.*8.780282057792199e-11)./(cos(x_3).^4.*1.45125e-1+sin(x_3).^4.*1.45125e-1+cos(x_3).^2.*sin(x_3).^2.*2.9025e-1)-(xpp_ref.*cos(x_3).^2.*sin(x_3).*sin(x_4).^2.*5.069298209627167e-11)./(cos(x_3).^4.*1.45125e-1+sin(x_3).^4.*1.45125e-1+cos(x_3).^2.*sin(x_3).^2.*2.9025e-1)-(xpp_ref.*cos(x_3).*sin(x_3).^2.*sin(x_5).^2.*8.780282057792199e-11)./(cos(x_3).^4.*1.45125e-1+sin(x_3).^4.*1.45125e-1+cos(x_3).^2.*sin(x_3).^2.*2.9025e-1)-(xpp_ref.*cos(x_3).^2.*sin(x_3).*sin(x_5).^2.*5.069298209627167e-11)./(cos(x_3).^4.*1.45125e-1+sin(x_3).^4.*1.45125e-1+cos(x_3).^2.*sin(x_3).^2.*2.9025e-1)-(xpp_ref.*cos(x_3).*sin(x_3).^2.*sin(x_6).^2.*8.780282057792199e-11)./(cos(x_3).^4.*1.45125e-1+sin(x_3).^4.*1.45125e-1+cos(x_3).^2.*sin(x_3).^2.*2.9025e-1)-(xpp_ref.*cos(x_3).^2.*sin(x_3).*sin(x_6).^2.*5.069298209627167e-11)./(cos(x_3).^4.*1.45125e-1+sin(x_3).^4.*1.45125e-1+cos(x_3).^2.*sin(x_3).^2.*2.9025e-1)+(y_ref.*cos(x_3).*sin(x_3).^2.*sin(x_4).^2.*2.027719283850867e-10)./(cos(x_3).^4.*1.45125e-1+sin(x_3).^4.*1.45125e-1+cos(x_3).^2.*sin(x_3).^2.*2.9025e-1)-(y_ref.*cos(x_3).^2.*sin(x_3).*sin(x_4).^2.*3.51211282311688e-10)./(cos(x_3).^4.*1.45125e-1+sin(x_3).^4.*1.45125e-1+cos(x_3).^2.*sin(x_3).^2.*2.9025e-1)+(y_ref.*cos(x_3).*sin(x_3).^2.*sin(x_5).^2.*2.027719283850867e-10)./(cos(x_3).^4.*1.45125e-1+sin(x_3).^4.*1.45125e-1+cos(x_3).^2.*sin(x_3).^2.*2.9025e-1)-(y_ref.*cos(x_3).^2.*sin(x_3).*sin(x_5).^2.*3.51211282311688e-10)./(cos(x_3).^4.*1.45125e-1+sin(x_3).^4.*1.45125e-1+cos(x_3).^2.*sin(x_3).^2.*2.9025e-1)+(y_ref.*cos(x_3).*sin(x_3).^2.*sin(x_6).^2.*2.027719283850867e-10)./(cos(x_3).^4.*1.45125e-1+sin(x_3).^4.*1.45125e-1+cos(x_3).^2.*sin(x_3).^2.*2.9025e-1)-(y_ref.*cos(x_3).^2.*sin(x_3).*sin(x_6).^2.*3.51211282311688e-10)./(cos(x_3).^4.*1.45125e-1+sin(x_3).^4.*1.45125e-1+cos(x_3).^2.*sin(x_3).^2.*2.9025e-1)+(yp_ref.*cos(x_3).*sin(x_3).^2.*sin(x_4).^2.*2.027719283850867e-10)./(cos(x_3).^4.*1.45125e-1+sin(x_3).^4.*1.45125e-1+cos(x_3).^2.*sin(x_3).^2.*2.9025e-1)-(yp_ref.*cos(x_3).^2.*sin(x_3).*sin(x_4).^2.*3.51211282311688e-10)./(cos(x_3).^4.*1.45125e-1+sin(x_3).^4.*1.45125e-1+cos(x_3).^2.*sin(x_3).^2.*2.9025e-1)+(yp_ref.*cos(x_3).*sin(x_3).^2.*sin(x_5).^2.*2.027719283850867e-10)./(cos(x_3).^4.*1.45125e-1+sin(x_3).^4.*1.45125e-1+cos(x_3).^2.*sin(x_3).^2.*2.9025e-1)-(yp_ref.*cos(x_3).^2.*sin(x_3).*sin(x_5).^2.*3.51211282311688e-10)./(cos(x_3).^4.*1.45125e-1+sin(x_3).^4.*1.45125e-1+cos(x_3).^2.*sin(x_3).^2.*2.9025e-1)+(yp_ref.*cos(x_3).*sin(x_3).^2.*sin(x_6).^2.*2.027719283850867e-10)./(cos(x_3).^4.*1.45125e-1+sin(x_3).^4.*1.45125e-1+cos(x_3).^2.*sin(x_3).^2.*2.9025e-1)-(yp_ref.*cos(x_3).^2.*sin(x_3).*sin(x_6).^2.*3.51211282311688e-10)./(cos(x_3).^4.*1.45125e-1+sin(x_3).^4.*1.45125e-1+cos(x_3).^2.*sin(x_3).^2.*2.9025e-1)+(ypp_ref.*cos(x_3).*sin(x_3).^2.*sin(x_4).^2.*5.069298209627167e-11)./(cos(x_3).^4.*1.45125e-1+sin(x_3).^4.*1.45125e-1+cos(x_3).^2.*sin(x_3).^2.*2.9025e-1)-(ypp_ref.*cos(x_3).^2.*sin(x_3).*sin(x_4).^2.*8.780282057792199e-11)./(cos(x_3).^4.*1.45125e-1+sin(x_3).^4.*1.45125e-1+cos(x_3).^2.*sin(x_3).^2.*2.9025e-1)+(ypp_ref.*cos(x_3).*sin(x_3).^2.*sin(x_5).^2.*5.069298209627167e-11)./(cos(x_3).^4.*1.45125e-1+sin(x_3).^4.*1.45125e-1+cos(x_3).^2.*sin(x_3).^2.*2.9025e-1)-(ypp_ref.*cos(x_3).^2.*sin(x_3).*sin(x_5).^2.*8.780282057792199e-11)./(cos(x_3).^4.*1.45125e-1+sin(x_3).^4.*1.45125e-1+cos(x_3).^2.*sin(x_3).^2.*2.9025e-1)+(ypp_ref.*cos(x_3).*sin(x_3).^2.*sin(x_6).^2.*5.069298209627167e-11)./(cos(x_3).^4.*1.45125e-1+sin(x_3).^4.*1.45125e-1+cos(x_3).^2.*sin(x_3).^2.*2.9025e-1)-(ypp_ref.*cos(x_3).^2.*sin(x_3).*sin(x_6).^2.*8.780282057792199e-11)./(cos(x_3).^4.*1.45125e-1+sin(x_3).^4.*1.45125e-1+cos(x_3).^2.*sin(x_3).^2.*2.9025e-1)+(x_9.^2.*cos(x_3).*sin(x_3).^2.*sin(x_4).^2.*8.701333683996604e-55)./(cos(x_3).^4.*1.5163227196875e-5+sin(x_3).^4.*1.5163227196875e-5+cos(x_3).^4.*cos(x_4).^2.*2.702824874801215e-10+cos(x_3).^4.*cos(x_5).^2.*2.702824874801215e-10+cos(x_3).^4.*cos(x_6).^2.*2.702824874801215e-10+cos(x_3).^2.*sin(x_3).^2.*3.032645439375e-5+cos(x_4).^2.*sin(x_3).^4.*2.702824874801215e-10+cos(x_5).^2.*sin(x_3).^4.*2.702824874801215e-10+cos(x_6).^2.*sin(x_3).^4.*2.702824874801215e-10+cos(x_3).^2.*cos(x_4).^2.*sin(x_3).^2.*5.40564974960243e-10+cos(x_3).^2.*cos(x_5).^2.*sin(x_3).^2.*5.40564974960243e-10+cos(x_3).^2.*cos(x_6).^2.*sin(x_3).^2.*5.40564974960243e-10)+(x_9.^2.*cos(x_3).^2.*sin(x_3).*sin(x_4).^2.*2.331515333700616e-55)./(cos(x_3).^4.*1.5163227196875e-5+sin(x_3).^4.*1.5163227196875e-5+cos(x_3).^4.*cos(x_4).^2.*2.702824874801215e-10+cos(x_3).^4.*cos(x_5).^2.*2.702824874801215e-10+cos(x_3).^4.*cos(x_6).^2.*2.702824874801215e-10+cos(x_3).^2.*sin(x_3).^2.*3.032645439375e-5+cos(x_4).^2.*sin(x_3).^4.*2.702824874801215e-10+cos(x_5).^2.*sin(x_3).^4.*2.702824874801215e-10+cos(x_6).^2.*sin(x_3).^4.*2.702824874801215e-10+cos(x_3).^2.*cos(x_4).^2.*sin(x_3).^2.*5.40564974960243e-10+cos(x_3).^2.*cos(x_5).^2.*sin(x_3).^2.*5.40564974960243e-10+cos(x_3).^2.*cos(x_6).^2.*sin(x_3).^2.*5.40564974960243e-10)+(x_9.^2.*cos(x_3).*sin(x_3).^2.*sin(x_5).^2.*8.701333683996604e-55)./(cos(x_3).^4.*1.5163227196875e-5+sin(x_3).^4.*1.5163227196875e-5+cos(x_3).^4.*cos(x_4).^2.*2.702824874801215e-10+cos(x_3).^4.*cos(x_5).^2.*2.702824874801215e-10+cos(x_3).^4.*cos(x_6).^2.*2.702824874801215e-10+cos(x_3).^2.*sin(x_3).^2.*3.032645439375e-5+cos(x_4).^2.*sin(x_3).^4.*2.702824874801215e-10+cos(x_5).^2.*sin(x_3).^4.*2.702824874801215e-10+cos(x_6).^2.*sin(x_3).^4.*2.702824874801215e-10+cos(x_3).^2.*cos(x_4).^2.*sin(x_3).^2.*5.40564974960243e-10+cos(x_3).^2.*cos(x_5).^2.*sin(x_3).^2.*5.40564974960243e-10+cos(x_3).^2.*cos(x_6).^2.*sin(x_3).^2.*5.40564974960243e-10)+(x_9.^2.*cos(x_3).^2.*sin(x_3).*sin(x_5).^2.*2.331515333700616e-55)./(cos(x_3).^4.*1.5163227196875e-5+sin(x_3).^4.*1.5163227196875e-5+cos(x_3).^4.*cos(x_4).^2.*2.702824874801215e-10+cos(x_3).^4.*cos(x_5).^2.*2.702824874801215e-10+cos(x_3).^4.*cos(x_6).^2.*2.702824874801215e-10+cos(x_3).^2.*sin(x_3).^2.*3.032645439375e-5+cos(x_4).^2.*sin(x_3).^4.*2.702824874801215e-10+cos(x_5).^2.*sin(x_3).^4.*2.702824874801215e-10+cos(x_6).^2.*sin(x_3).^4.*2.702824874801215e-10+cos(x_3).^2.*cos(x_4).^2.*sin(x_3).^2.*5.40564974960243e-10+cos(x_3).^2.*cos(x_5).^2.*sin(x_3).^2.*5.40564974960243e-10+cos(x_3).^2.*cos(x_6).^2.*sin(x_3).^2.*5.40564974960243e-10)+(x_9.^2.*cos(x_3).*sin(x_3).^2.*sin(x_6).^2.*8.701333683996604e-55)./(cos(x_3).^4.*1.5163227196875e-5+sin(x_3).^4.*1.5163227196875e-5+cos(x_3).^4.*cos(x_4).^2.*2.702824874801215e-10+cos(x_3).^4.*cos(x_5).^2.*2.702824874801215e-10+cos(x_3).^4.*cos(x_6).^2.*2.702824874801215e-10+cos(x_3).^2.*sin(x_3).^2.*3.032645439375e-5+cos(x_4).^2.*sin(x_3).^4.*2.702824874801215e-10+cos(x_5).^2.*sin(x_3).^4.*2.702824874801215e-10+cos(x_6).^2.*sin(x_3).^4.*2.702824874801215e-10+cos(x_3).^2.*cos(x_4).^2.*sin(x_3).^2.*5.40564974960243e-10+cos(x_3).^2.*cos(x_5).^2.*sin(x_3).^2.*5.40564974960243e-10+cos(x_3).^2.*cos(x_6).^2.*sin(x_3).^2.*5.40564974960243e-10)+(x_9.^2.*cos(x_3).^2.*sin(x_3).*sin(x_6).^2.*2.331515333700616e-55)./(cos(x_3).^4.*1.5163227196875e-5+sin(x_3).^4.*1.5163227196875e-5+cos(x_3).^4.*cos(x_4).^2.*2.702824874801215e-10+cos(x_3).^4.*cos(x_5).^2.*2.702824874801215e-10+cos(x_3).^4.*cos(x_6).^2.*2.702824874801215e-10+cos(x_3).^2.*sin(x_3).^2.*3.032645439375e-5+cos(x_4).^2.*sin(x_3).^4.*2.702824874801215e-10+cos(x_5).^2.*sin(x_3).^4.*2.702824874801215e-10+cos(x_6).^2.*sin(x_3).^4.*2.702824874801215e-10+cos(x_3).^2.*cos(x_4).^2.*sin(x_3).^2.*5.40564974960243e-10+cos(x_3).^2.*cos(x_5).^2.*sin(x_3).^2.*5.40564974960243e-10+cos(x_3).^2.*cos(x_6).^2.*sin(x_3).^2.*5.40564974960243e-10)-(th_ref.*cos(x_3).^2.*sin(x_3).^2.*sin(x_4).^2.*2.715383044549796e-11)./(cos(x_3).^4.*3.628125e-2+sin(x_3).^4.*3.628125e-2+cos(x_3).^2.*sin(x_3).^2.*7.25625e-2)-(th_ref.*cos(x_3).^2.*sin(x_3).^2.*sin(x_5).^2.*2.715383044549796e-11)./(cos(x_3).^4.*3.628125e-2+sin(x_3).^4.*3.628125e-2+cos(x_3).^2.*sin(x_3).^2.*7.25625e-2)+(th_ref.*cos(x_3).^2.*sin(x_3).^2.*sin(x_4).^4.*2.419937491571796e-16)./(cos(x_3).^4.*3.628125e-2+sin(x_3).^4.*3.628125e-2+cos(x_3).^2.*sin(x_3).^2.*7.25625e-2)-(th_ref.*cos(x_3).^2.*sin(x_3).^2.*sin(x_6).^2.*2.715383044549796e-11)./(cos(x_3).^4.*3.628125e-2+sin(x_3).^4.*3.628125e-2+cos(x_3).^2.*sin(x_3).^2.*7.25625e-2)+(th_ref.*cos(x_3).^2.*sin(x_3).^2.*sin(x_5).^4.*2.419937491571796e-16)./(cos(x_3).^4.*3.628125e-2+sin(x_3).^4.*3.628125e-2+cos(x_3).^2.*sin(x_3).^2.*7.25625e-2)+(th_ref.*cos(x_3).^2.*sin(x_3).^2.*sin(x_6).^4.*2.419937491571796e-16)./(cos(x_3).^4.*3.628125e-2+sin(x_3).^4.*3.628125e-2+cos(x_3).^2.*sin(x_3).^2.*7.25625e-2)+(th_ref.*cos(x_3).^4.*sin(x_4).^2.*sin(x_5).^2.*2.419937491571796e-16)./(cos(x_3).^4.*3.628125e-2+sin(x_3).^4.*3.628125e-2+cos(x_3).^2.*sin(x_3).^2.*7.25625e-2)+(th_ref.*cos(x_3).^4.*sin(x_4).^2.*sin(x_6).^2.*2.419937491571796e-16)./(cos(x_3).^4.*3.628125e-2+sin(x_3).^4.*3.628125e-2+cos(x_3).^2.*sin(x_3).^2.*7.25625e-2)+(th_ref.*cos(x_3).^4.*sin(x_5).^2.*sin(x_6).^2.*2.419937491571796e-16)./(cos(x_3).^4.*3.628125e-2+sin(x_3).^4.*3.628125e-2+cos(x_3).^2.*sin(x_3).^2.*7.25625e-2)-(thp_ref.*cos(x_3).^2.*sin(x_3).^2.*sin(x_4).^2.*2.715383044549796e-11)./(cos(x_3).^4.*3.628125e-2+sin(x_3).^4.*3.628125e-2+cos(x_3).^2.*sin(x_3).^2.*7.25625e-2)-(thp_ref.*cos(x_3).^2.*sin(x_3).^2.*sin(x_5).^2.*2.715383044549796e-11)./(cos(x_3).^4.*3.628125e-2+sin(x_3).^4.*3.628125e-2+cos(x_3).^2.*sin(x_3).^2.*7.25625e-2)+(thp_ref.*cos(x_3).^2.*sin(x_3).^2.*sin(x_4).^4.*2.419937491571796e-16)./(cos(x_3).^4.*3.628125e-2+sin(x_3).^4.*3.628125e-2+cos(x_3).^2.*sin(x_3).^2.*7.25625e-2)-(thp_ref.*cos(x_3).^2.*sin(x_3).^2.*sin(x_6).^2.*2.715383044549796e-11)./(cos(x_3).^4.*3.628125e-2+sin(x_3).^4.*3.628125e-2+cos(x_3).^2.*sin(x_3).^2.*7.25625e-2)+(thp_ref.*cos(x_3).^2.*sin(x_3).^2.*sin(x_5).^4.*2.419937491571796e-16)./(cos(x_3).^4.*3.628125e-2+sin(x_3).^4.*3.628125e-2+cos(x_3).^2.*sin(x_3).^2.*7.25625e-2)+(thp_ref.*cos(x_3).^2.*sin(x_3).^2.*sin(x_6).^4.*2.419937491571796e-16)./(cos(x_3).^4.*3.628125e-2+sin(x_3).^4.*3.628125e-2+cos(x_3).^2.*sin(x_3).^2.*7.25625e-2)+(thp_ref.*cos(x_3).^4.*sin(x_4).^2.*sin(x_5).^2.*2.419937491571796e-16)./(cos(x_3).^4.*3.628125e-2+sin(x_3).^4.*3.628125e-2+cos(x_3).^2.*sin(x_3).^2.*7.25625e-2)+(thp_ref.*cos(x_3).^4.*sin(x_4).^2.*sin(x_6).^2.*2.419937491571796e-16)./(cos(x_3).^4.*3.628125e-2+sin(x_3).^4.*3.628125e-2+cos(x_3).^2.*sin(x_3).^2.*7.25625e-2)+(thp_ref.*cos(x_3).^4.*sin(x_5).^2.*sin(x_6).^2.*2.419937491571796e-16)./(cos(x_3).^4.*3.628125e-2+sin(x_3).^4.*3.628125e-2+cos(x_3).^2.*sin(x_3).^2.*7.25625e-2)-(thpp_ref.*cos(x_3).^2.*sin(x_3).^2.*sin(x_4).^2.*6.788457611374491e-12)./(cos(x_3).^4.*3.628125e-2+sin(x_3).^4.*3.628125e-2+cos(x_3).^2.*sin(x_3).^2.*7.25625e-2)-(thpp_ref.*cos(x_3).^2.*sin(x_3).^2.*sin(x_5).^2.*6.788457611374491e-12)./(cos(x_3).^4.*3.628125e-2+sin(x_3).^4.*3.628125e-2+cos(x_3).^2.*sin(x_3).^2.*7.25625e-2)+(thpp_ref.*cos(x_3).^2.*sin(x_3).^2.*sin(x_4).^4.*6.049843728929489e-17)./(cos(x_3).^4.*3.628125e-2+sin(x_3).^4.*3.628125e-2+cos(x_3).^2.*sin(x_3).^2.*7.25625e-2)-(thpp_ref.*cos(x_3).^2.*sin(x_3).^2.*sin(x_6).^2.*6.788457611374491e-12)./(cos(x_3).^4.*3.628125e-2+sin(x_3).^4.*3.628125e-2+cos(x_3).^2.*sin(x_3).^2.*7.25625e-2)+(thpp_ref.*cos(x_3).^2.*sin(x_3).^2.*sin(x_5).^4.*6.049843728929489e-17)./(cos(x_3).^4.*3.628125e-2+sin(x_3).^4.*3.628125e-2+cos(x_3).^2.*sin(x_3).^2.*7.25625e-2)+(thpp_ref.*cos(x_3).^2.*sin(x_3).^2.*sin(x_6).^4.*6.049843728929489e-17)./(cos(x_3).^4.*3.628125e-2+sin(x_3).^4.*3.628125e-2+cos(x_3).^2.*sin(x_3).^2.*7.25625e-2)+(thpp_ref.*cos(x_3).^4.*sin(x_4).^2.*sin(x_5).^2.*6.049843728929489e-17)./(cos(x_3).^4.*3.628125e-2+sin(x_3).^4.*3.628125e-2+cos(x_3).^2.*sin(x_3).^2.*7.25625e-2)+(thpp_ref.*cos(x_3).^4.*sin(x_4).^2.*sin(x_6).^2.*6.049843728929489e-17)./(cos(x_3).^4.*3.628125e-2+sin(x_3).^4.*3.628125e-2+cos(x_3).^2.*sin(x_3).^2.*7.25625e-2)+(thpp_ref.*cos(x_3).^4.*sin(x_5).^2.*sin(x_6).^2.*6.049843728929489e-17)./(cos(x_3).^4.*3.628125e-2+sin(x_3).^4.*3.628125e-2+cos(x_3).^2.*sin(x_3).^2.*7.25625e-2)+(x_3.*cos(x_3).^2.*sin(x_3).^2.*sin(x_4).^2.*2.715383044549796e-11)./(cos(x_3).^4.*3.628125e-2+sin(x_3).^4.*3.628125e-2+cos(x_3).^2.*sin(x_3).^2.*7.25625e-2)+(x_3.*cos(x_3).^2.*sin(x_3).^2.*sin(x_5).^2.*2.715383044549796e-11)./(cos(x_3).^4.*3.628125e-2+sin(x_3).^4.*3.628125e-2+cos(x_3).^2.*sin(x_3).^2.*7.25625e-2)-(x_3.*cos(x_3).^2.*sin(x_3).^2.*sin(x_4).^4.*2.419937491571796e-16)./(cos(x_3).^4.*3.628125e-2+sin(x_3).^4.*3.628125e-2+cos(x_3).^2.*sin(x_3).^2.*7.25625e-2)+(x_3.*cos(x_3).^2.*sin(x_3).^2.*sin(x_6).^2.*2.715383044549796e-11)./(cos(x_3).^4.*3.628125e-2+sin(x_3).^4.*3.628125e-2+cos(x_3).^2.*sin(x_3).^2.*7.25625e-2)-(x_3.*cos(x_3).^2.*sin(x_3).^2.*sin(x_5).^4.*2.419937491571796e-16)./(cos(x_3).^4.*3.628125e-2+sin(x_3).^4.*3.628125e-2+cos(x_3).^2.*sin(x_3).^2.*7.25625e-2)-(x_3.*cos(x_3).^2.*sin(x_3).^2.*sin(x_6).^4.*2.419937491571796e-16)./(cos(x_3).^4.*3.628125e-2+sin(x_3).^4.*3.628125e-2+cos(x_3).^2.*sin(x_3).^2.*7.25625e-2)-(x_3.*cos(x_3).^4.*sin(x_4).^2.*sin(x_5).^2.*2.419937491571796e-16)./(cos(x_3).^4.*3.628125e-2+sin(x_3).^4.*3.628125e-2+cos(x_3).^2.*sin(x_3).^2.*7.25625e-2)-(x_3.*cos(x_3).^4.*sin(x_4).^2.*sin(x_6).^2.*2.419937491571796e-16)./(cos(x_3).^4.*3.628125e-2+sin(x_3).^4.*3.628125e-2+cos(x_3).^2.*sin(x_3).^2.*7.25625e-2)-(x_3.*cos(x_3).^4.*sin(x_5).^2.*sin(x_6).^2.*2.419937491571796e-16)./(cos(x_3).^4.*3.628125e-2+sin(x_3).^4.*3.628125e-2+cos(x_3).^2.*sin(x_3).^2.*7.25625e-2)+(x_9.*cos(x_3).^2.*sin(x_3).^2.*sin(x_4).^2.*2.715383044549796e-11)./(cos(x_3).^4.*3.628125e-2+sin(x_3).^4.*3.628125e-2+cos(x_3).^2.*sin(x_3).^2.*7.25625e-2)+(x_9.*cos(x_3).^2.*sin(x_3).^2.*sin(x_5).^2.*2.715383044549796e-11)./(cos(x_3).^4.*3.628125e-2+sin(x_3).^4.*3.628125e-2+cos(x_3).^2.*sin(x_3).^2.*7.25625e-2)-(x_9.*cos(x_3).^2.*sin(x_3).^2.*sin(x_4).^4.*2.419937491571796e-16)./(cos(x_3).^4.*3.628125e-2+sin(x_3).^4.*3.628125e-2+cos(x_3).^2.*sin(x_3).^2.*7.25625e-2)+(x_9.*cos(x_3).^2.*sin(x_3).^2.*sin(x_6).^2.*2.715383044549796e-11)./(cos(x_3).^4.*3.628125e-2+sin(x_3).^4.*3.628125e-2+cos(x_3).^2.*sin(x_3).^2.*7.25625e-2)-(x_9.*cos(x_3).^2.*sin(x_3).^2.*sin(x_5).^4.*2.419937491571796e-16)./(cos(x_3).^4.*3.628125e-2+sin(x_3).^4.*3.628125e-2+cos(x_3).^2.*sin(x_3).^2.*7.25625e-2)-(x_9.*cos(x_3).^2.*sin(x_3).^2.*sin(x_6).^4.*2.419937491571796e-16)./(cos(x_3).^4.*3.628125e-2+sin(x_3).^4.*3.628125e-2+cos(x_3).^2.*sin(x_3).^2.*7.25625e-2)-(x_9.*cos(x_3).^4.*sin(x_4).^2.*sin(x_5).^2.*2.419937491571796e-16)./(cos(x_3).^4.*3.628125e-2+sin(x_3).^4.*3.628125e-2+cos(x_3).^2.*sin(x_3).^2.*7.25625e-2)-(x_9.*cos(x_3).^4.*sin(x_4).^2.*sin(x_6).^2.*2.419937491571796e-16)./(cos(x_3).^4.*3.628125e-2+sin(x_3).^4.*3.628125e-2+cos(x_3).^2.*sin(x_3).^2.*7.25625e-2)-(x_9.*cos(x_3).^4.*sin(x_5).^2.*sin(x_6).^2.*2.419937491571796e-16)./(cos(x_3).^4.*3.628125e-2+sin(x_3).^4.*3.628125e-2+cos(x_3).^2.*sin(x_3).^2.*7.25625e-2)+(th_ref.*sin(x_3).^4.*sin(x_4).^2.*sin(x_5).^2.*2.419937491571796e-16)./(cos(x_3).^4.*3.628125e-2+sin(x_3).^4.*3.628125e-2+cos(x_3).^2.*sin(x_3).^2.*7.25625e-2)+(th_ref.*sin(x_3).^4.*sin(x_4).^2.*sin(x_6).^2.*2.419937491571796e-16)./(cos(x_3).^4.*3.628125e-2+sin(x_3).^4.*3.628125e-2+cos(x_3).^2.*sin(x_3).^2.*7.25625e-2)+(th_ref.*sin(x_3).^4.*sin(x_5).^2.*sin(x_6).^2.*2.419937491571796e-16)./(cos(x_3).^4.*3.628125e-2+sin(x_3).^4.*3.628125e-2+cos(x_3).^2.*sin(x_3).^2.*7.25625e-2)+(thp_ref.*sin(x_3).^4.*sin(x_4).^2.*sin(x_5).^2.*2.419937491571796e-16)./(cos(x_3).^4.*3.628125e-2+sin(x_3).^4.*3.628125e-2+cos(x_3).^2.*sin(x_3).^2.*7.25625e-2)+(thp_ref.*sin(x_3).^4.*sin(x_4).^2.*sin(x_6).^2.*2.419937491571796e-16)./(cos(x_3).^4.*3.628125e-2+sin(x_3).^4.*3.628125e-2+cos(x_3).^2.*sin(x_3).^2.*7.25625e-2)+(thp_ref.*sin(x_3).^4.*sin(x_5).^2.*sin(x_6).^2.*2.419937491571796e-16)./(cos(x_3).^4.*3.628125e-2+sin(x_3).^4.*3.628125e-2+cos(x_3).^2.*sin(x_3).^2.*7.25625e-2)+(thpp_ref.*sin(x_3).^4.*sin(x_4).^2.*sin(x_5).^2.*6.049843728929489e-17)./(cos(x_3).^4.*3.628125e-2+sin(x_3).^4.*3.628125e-2+cos(x_3).^2.*sin(x_3).^2.*7.25625e-2)+(thpp_ref.*sin(x_3).^4.*sin(x_4).^2.*sin(x_6).^2.*6.049843728929489e-17)./(cos(x_3).^4.*3.628125e-2+sin(x_3).^4.*3.628125e-2+cos(x_3).^2.*sin(x_3).^2.*7.25625e-2)+(thpp_ref.*sin(x_3).^4.*sin(x_5).^2.*sin(x_6).^2.*6.049843728929489e-17)./(cos(x_3).^4.*3.628125e-2+sin(x_3).^4.*3.628125e-2+cos(x_3).^2.*sin(x_3).^2.*7.25625e-2)-(x_3.*sin(x_3).^4.*sin(x_4).^2.*sin(x_5).^2.*2.419937491571796e-16)./(cos(x_3).^4.*3.628125e-2+sin(x_3).^4.*3.628125e-2+cos(x_3).^2.*sin(x_3).^2.*7.25625e-2)-(x_3.*sin(x_3).^4.*sin(x_4).^2.*sin(x_6).^2.*2.419937491571796e-16)./(cos(x_3).^4.*3.628125e-2+sin(x_3).^4.*3.628125e-2+cos(x_3).^2.*sin(x_3).^2.*7.25625e-2)-(x_3.*sin(x_3).^4.*sin(x_5).^2.*sin(x_6).^2.*2.419937491571796e-16)./(cos(x_3).^4.*3.628125e-2+sin(x_3).^4.*3.628125e-2+cos(x_3).^2.*sin(x_3).^2.*7.25625e-2)-(x_9.*sin(x_3).^4.*sin(x_4).^2.*sin(x_5).^2.*2.419937491571796e-16)./(cos(x_3).^4.*3.628125e-2+sin(x_3).^4.*3.628125e-2+cos(x_3).^2.*sin(x_3).^2.*7.25625e-2)-(x_9.*sin(x_3).^4.*sin(x_4).^2.*sin(x_6).^2.*2.419937491571796e-16)./(cos(x_3).^4.*3.628125e-2+sin(x_3).^4.*3.628125e-2+cos(x_3).^2.*sin(x_3).^2.*7.25625e-2)-(x_9.*sin(x_3).^4.*sin(x_5).^2.*sin(x_6).^2.*2.419937491571796e-16)./(cos(x_3).^4.*3.628125e-2+sin(x_3).^4.*3.628125e-2+cos(x_3).^2.*sin(x_3).^2.*7.25625e-2)-(x_9.^2.*sin(x_4.*2.0).*cos(x_3).*sin(x_3).^2.*2.103394848799675e-14)./(cos(x_3).^4.*1.5163227196875e-5+sin(x_3).^4.*1.5163227196875e-5+cos(x_3).^4.*cos(x_4).^2.*2.702824874801215e-10+cos(x_3).^4.*cos(x_5).^2.*2.702824874801215e-10+cos(x_3).^4.*cos(x_6).^2.*2.702824874801215e-10+cos(x_3).^2.*sin(x_3).^2.*3.032645439375e-5+cos(x_4).^2.*sin(x_3).^4.*2.702824874801215e-10+cos(x_5).^2.*sin(x_3).^4.*2.702824874801215e-10+cos(x_6).^2.*sin(x_3).^4.*2.702824874801215e-10+cos(x_3).^2.*cos(x_4).^2.*sin(x_3).^2.*5.40564974960243e-10+cos(x_3).^2.*cos(x_5).^2.*sin(x_3).^2.*5.40564974960243e-10+cos(x_3).^2.*cos(x_6).^2.*sin(x_3).^2.*5.40564974960243e-10)-(x_9.^2.*sin(x_4.*2.0).*cos(x_3).^2.*sin(x_3).*5.636029510996564e-15)./(cos(x_3).^4.*1.5163227196875e-5+sin(x_3).^4.*1.5163227196875e-5+cos(x_3).^4.*cos(x_4).^2.*2.702824874801215e-10+cos(x_3).^4.*cos(x_5).^2.*2.702824874801215e-10+cos(x_3).^4.*cos(x_6).^2.*2.702824874801215e-10+cos(x_3).^2.*sin(x_3).^2.*3.032645439375e-5+cos(x_4).^2.*sin(x_3).^4.*2.702824874801215e-10+cos(x_5).^2.*sin(x_3).^4.*2.702824874801215e-10+cos(x_6).^2.*sin(x_3).^4.*2.702824874801215e-10+cos(x_3).^2.*cos(x_4).^2.*sin(x_3).^2.*5.40564974960243e-10+cos(x_3).^2.*cos(x_5).^2.*sin(x_3).^2.*5.40564974960243e-10+cos(x_3).^2.*cos(x_6).^2.*sin(x_3).^2.*5.40564974960243e-10)-(x_9.^2.*sin(x_5.*2.0).*cos(x_3).*sin(x_3).^2.*2.103394848799675e-14)./(cos(x_3).^4.*1.5163227196875e-5+sin(x_3).^4.*1.5163227196875e-5+cos(x_3).^4.*cos(x_4).^2.*2.702824874801215e-10+cos(x_3).^4.*cos(x_5).^2.*2.702824874801215e-10+cos(x_3).^4.*cos(x_6).^2.*2.702824874801215e-10+cos(x_3).